simulink model "SimulinkAnalysisofCheetahTail"  (R2022a)
(part 3 of 21)

t1533 = t1424./2.0;
t1534 = t1425./2.0;
t1535 = t1426./2.0;
t1536 = dpsi1.*t1470;
t1541 = t1432./2.0;
t1572 = Mt.*t4.*t5.*t1381;
t1573 = T_cg_H.*t1512;
t1580 = dphi2.*t1512;
t1581 = dpsi1.*t1512;
t1585 = Mb.*t2.*t10.*t1382;
t1587 = Mb.*t7.*t10.*t1382;
t1592 = -t1540;
t1594 = -t1545;
t1595 = Mb.*t2.*t5.*t1362;
t1599 = Mb.*t5.*t7.*t1362;
t1601 = -t1553;
t1602 = -t1554;
t1603 = -t1556;
t1606 = t1488./2.0;
t1621 = Mm.*t9.*t10.*t1394;
t1624 = Mb.*t11.*t15.*t459.*t964;
t1655 = Mm.*t5.*t33.*t1394;
t1656 = Mm.*t5.*t38.*t1394;
t1658 = B_cg_H.*Mb.*t382.*t1178;
t1659 = Mm.*t4.*t10.*t1470;
t1669 = -t1629;
t1680 = Mm.*t381.*t1221;
t1681 = Mm.*t382.*t1221;
t1686 = -t1652;
t1695 = B_cg_H.*Mb.*t4.*t5.*t1512;
t1698 = t496.*t1178;
t1699 = B_cg_H.*Mb.*t9.*t10.*t1512;
t1703 = B_cg_H.*Mb.*t7.*t100.*t1382;
t1705 = t11.*t420.*t1178;
C = ft_5({B_cg_H,ITail,Mb,Mm,Mt,T_cg_H,dphi1,dphi2,dpsi1,dth1,dth2,dx,dy,dz,t10,t1003,t1004,t1005,t1006,t1007,t1008,t1009,t1010,t1011,t1012,t1013,t1014,t1015,t1016,t1017,t1018,t1019,t1020,t1021,t1023,t1024,t1025,t1026,t1029,t103,t1030,t1031,t1036,t1037,t1041,t1042,t1043,t1044,t1045,t1046,t1047,t1049,t105,t1050,t1051,t1052,t1053,t1054,t1055,t1056,t1057,t1058,t1059,t1060,t1061,t1062,t1063,t1064,t1065,t1067,t1068,t1071,t1072,t1073,t1074,t1075,t1076,t1077,t1078,t1079,t1080,t1081,t1082,t1084,t1085,t1086,t1088,t1093,t1095,t1097,t11,t1102,t1105,t1108,t1109,t1113,t1114,t1115,t1116,t1117,t1118,t1119,t1120,t1121,t1122,t1123,t1124,t1125,t1126,t1127,t1128,t1129,t1130,t1131,t1132,t1133,t1134,t1135,t1136,t1137,t1138,t1139,t1140,t1141,t1142,t1143,t1144,t1145,t1146,t1147,t1148,t1149,t1150,t1152,t1153,t1154,t1155,t1156,t1157,t1158,t1159,t1160,t1161,t1162,t1163,t1164,t1165,t1166,t1167,t1168,t1169,t1170,t1171,t1172,t1173,t1174,t1176,t1177,t1178,t1179,t1180,t1181,t1182,t1183,t1184,t1185,t1186,t1187,t1188,t1189,t1190,t1191,t1192,t1193,t1194,t1195,t1196,t1197,t1199,t120,t1200,t1201,t1202,t1203,t1205,t1206,t1207,t1209,t1211,t1212,t1213,t1214,t1215,t1216,t1217,t1218,t1221,t1223,t1224,t1225,t1226,t1227,t1228,t1229,t123,t1230,t1231,t1232,t1234,t1235,t1236,t1237,t1238,t1240,t1242,t1243,t1244,t1245,t1246,t1247,t1248,t1250,t1251,t1252,t1253,t1255,t1256,t1257,t1260,t1261,t1262,t1263,t1264,t1265,t1266,t1268,t1270,t1272,t1275,t1279,t1280,t1282,t1283,t1284,t1285,t1287,t1289,t1296,t130,t1301,t1302,t1303,t1304,t1305,t1306,t1307,t1308,t1309,t1311,t1312,t1313,t1319,t1320,t1322,t1323,t1324,t1325,t1328,t1329,t1331,t1332,t1334,t1335,t1337,t1338,t134,t1340,t1341,t1342,t1343,t1344,t1345,t1348,t1349,t1352,t1354,t1355,t1356,t1357,t1358,t1360,t1361,t1362,t1363,t1365,t1366,t1367,t1368,t1370,t1371,t1372,t1373,t1374,t1377,t1378,t1379,t1380,t1381,t1382,t1383,t1384,t1385,t1386,t1388,t1389,t1390,t1391,t1393,t1394,t1395,t1396,t1397,t1399,t1400,t1402,t1403,t1405,t1406,t1407,t1408,t1409,t1410,t1412,t1413,t1414,t1415,t1416,t1418,t1419,t1421,t1422,t1424,t1425,t1426,t1427,t1429,t1430,t1431,t1432,t1433,t1434,t1435,t1437,t1438,t1439,t144,t1440,t1441,t1442,t1443,t1444,t1445,t1446,t1447,t1448,t1450,t1451,t1453,t1454,t1455,t1456,t1457,t1458,t1459,t1460,t1461,t1462,t1463,t1465,t1466,t1467,t1468,t1469,t1470,t1471,t1472,t1475,t1476,t1477,t1478,t1479,t1481,t1482,t1483,t1484,t1486,t1487,t1488,t1489,t1491,t1492,t1493,t1494,t1495,t1496,t1497,t1498,t15,t1500,t1501,t1503,t1504,t1505,t1506,t1507,t1508,t1509,t1511,t1512,t1513,t1514,t1515,t1516,t1517,t1518,t1520,t1521,t1522,t1523,t1524,t1525,t1526,t1527,t1528,t1529,t1531,t1532,t1533,t1534,t1535,t1536,t1537,t1539,t1540,t1541,t1542,t1543,t1547,t1548,t1549,t1550,t1552,t1553,t1555,t1557,t1559,t1560,t1561,t1562,t1563,t1565,t1566,t1567,t1568,t1572,t1573,t1576,t1577,t1580,t1581,t1582,t1585,t1587,t1588,t1589,t1591,t1592,t1593,t1594,t1595,t1596,t1597,t1598,t1599,t160,t1600,t1601,t1602,t1603,t1605,t1606,t1609,t161,t1610,t1613,t1614,t1615,t1616,t1617,t1618,t1619,t162,t1620,t1621,t1624,t1627,t1628,t1632,t1635,t1636,t1637,t1639,t1640,t1641,t1642,t1644,t1645,t1646,t1647,t1648,t1649,t1651,t1652,t1653,t1654,t1655,t1656,t1657,t1658,t1659,t1660,t1661,t1663,t1664,t1665,t1667,t1668,t1669,t1670,t1671,t1672,t1673,t1674,t1675,t1676,t1677,t1678,t1679,t1680,t1681,t1682,t1683,t1684,t1685,t1686,t1687,t1688,t1689,t1690,t1691,t1692,t1693,t1694,t1695,t1698,t1699,t1700,t1701,t1702,t1703,t1704,t1705,t1706,t1707,t1708,t1709,t1710,t1711,t1712,t1714,t1715,t1716,t1717,t1718,t1723,t1726,t1727,t1731,t1732,t1733,t1734,t1737,t1741,t1742,t1743,t1744,t1745,t1747,t1749,t1751,t1758,t1759,t1760,t1761,t1762,t1764,t1765,t1769,t1770,t1773,t1775,t1777,t1784,t1786,t1788,t1791,t1796,t1798,t1799,t1801,t1802,t1803,t1805,t1806,t1808,t1810,t1812,t1813,t1814,t1815,t1817,t1819,t1820,t1824,t1825,t1826,t1829,t1830,t1832,t1836,t1837,t1838,t1839,t1841,t1844,t1851,t1852,t1856,t1862,t1865,t1866,t1867,t1871,t1873,t1874,t1875,t1881,t1884,t1888,t1894,t1895,t1896,t1897,t1899,t1903,t1905,t1906,t1907,t1908,t1909,t1910,t1911,t1912,t1913,t1914,t1915,t1916,t1918,t1919,t1921,t1922,t1926,t1928,t1930,t1931,t1936,t1940,t1941,t1942,t195,t1954,t1956,t1958,t1960,t1961,t1962,t1963,t1964,t1965,t1966,t1969,t197,t1970,t1971,t1973,t1974,t1975,t1979,t1981,t1982,t1983,t1985,t1989,t1990,t1998,t1999,t2,t2004,t2007,t2008,t2015,t2025,t2026,t2028,t2031,t2035,t2037,t2042,t2043,t2045,t2046,t2047,t2050,t2052,t2053,t2056,t2057,t2058,t2059,t2062,t2063,t2064,t2066,t2067,t2068,t2069,t2072,t2078,t2087,t2090,t2091,t2094,t2095,t2096,t2097,t2098,t2102,t2104,t2118,t2119,t2120,t2121,t2127,t213,t2130,t2131,t2134,t2135,t214,t2141,t2144,t2146,t2147,t2148,t2150,t2151,t2152,t2154,t2155,t2156,t2157,t2158,t2161,t2165,t2167,t2171,t2172,t2176,t2178,t2179,t2180,t2181,t2182,t2183,t2186,t2188,t2190,t2196,t2201,t2202,t2203,t2205,t2208,t2209,t2211,t2214,t2215,t2218,t2220,t2222,t2224,t2225,t2227,t2231,t2237,t2238,t2240,t2242,t2245,t2246,t2247,t2249,t2251,t2252,t2253,t2254,t2255,t2257,t2259,t2262,t2263,t2264,t2266,t2273,t2283,t2287,t2288,t2290,t2294,t2298,t23,t2303,t2305,t2306,t2307,t2312,t2320,t2321,t2322,t2323,t2324,t2326,t2327,t2328,t2331,t2335,t2336,t2339,t2340,t2341,t2342,t2343,t2345,t2346,t2347,t2349,t2350,t2351,t2356,t2358,t2359,t2360,t2362,t2363,t2376,t2379,t2383,t2385,t2386,t2387,t2388,t2389,t2390,t2392,t2397,t2399,t24,t2400,t2401,t2404,t2407,t2408,t2409,t2411,t2412,t2420,t2427,t2429,t2430,t2431,t2433,t2435,t2447,t2461,t2462,t2463,t2464,t2466,t2467,t2468,t2469,t2474,t2475,t2476,t2477,t2479,t2480,t2482,t2485,t2487,t2488,t2489,t2492,t2493,t2494,t2495,t2497,t25,t2503,t2504,t2505,t2512,t2514,t2515,t2516,t2518,t2519,t2520,t2527,t2530,t2531,t2532,t2534,t2539,t2544,t2545,t2546,t2560,t2562,t2563,t2564,t2565,t2566,t2570,t2576,t2577,t2581,t2584,t2586,t2587,t2588,t2589,t259,t2590,t2591,t2597,t2598,t2599,t26,t260,t2600,t2603,t2604,t2607,t2608,t2611,t2612,t2613,t2614,t2615,t2616,t2617,t2619,t262,t2620,t2621,t2622,t2624,t2626,t2627,t2632,t2634,t2638,t2654,t2660,t2662,t2663,t2664,t2665,t2668,t2669,t2671,t2673,t2681,t2682,t2689,t2692,t2693,t2694,t2695,t2698,t2699,t27,t2700,t2701,t2702,t2704,t2705,t2706,t2707,t2708,t2710,t2711,t2712,t2713,t2714,t2715,t2717,t2718,t2719,t2720,t2721,t2722,t2723,t2724,t273,t2730,t2731,t2732,t2740,t2742,t2745,t2749,t2751,t2752,t2756,t276,t2763,t2764,t2765,t2766,t277,t2774,t2776,t2781,t2782,t2783,t2784,t2786,t2787,t2788,t2790,t28,t2802,t2803,t2804,t2806,t2807,t2812,t2813,t2819,t2820,t2821,t2825,t2828,t283,t2835,t2837,t2839,t284,t2841,t2842,t2844,t285,t2857,t2859,t286,t287,t2870,t2872,t2874,t2875,t2879,t288,t2880,t2883,t2884,t2886,t2887,t2888,t2889,t289,t2890,t2892,t2895,t2896,t290,t2902,t2907,t2908,t2909,t291,t2912,t2913,t2916,t2918,t292,t2928,t2929,t293,t2932,t2938,t294,t2945,t2946,t2949,t2950,t2951,t2952,t2954,t2955,t2956,t2957,t2958,t2959,t2960,t2961,t2967,t2969,t2975,t2977,t2982,t2988,t2992,t2995,t3,t30,t3004,t3010,t3011,t3017,t3019,t3020,t3022,t3023,t3025,t3028,t3030,t3034,t3035,t3039,t304,t3047,t3048,t3051,t3055,t3058,t3059,t3060,t3063,t3065,t3067,t3068,t3074,t3075,t3077,t3078,t3081,t3085,t3088,t3090,t3105,t3109,t3111,t3117,t3120,t3124,t3130,t3132,t3134,t3135,t3136,t3138,t3153,t3165,t3170,t3173,t3177,t3181,t3182,t3186,t3188,t3191,t3194,t3199,t3200,t3201,t3204,t3210,t3212,t3218,t3235,t3237,t3243,t3247,t3248,t3249,t3256,t3260,t3265,t3266,t3269,t3272,t3285,t3291,t33,t3304,t3310,t3317,t3330,t3331,t3337,t3351,t3360,t3364,t3370,t3380,t34,t3419,t3426,t3428,t3434,t3438,t3441,t3449,t3459,t346,t3469,t347,t3471,t3478,t348,t3484,t3499,t35,t3504,t3520,t3521,t3522,t3527,t3531,t3565,t3580,t3581,t3644,t3701,t3704,t3709,t375,t376,t377,t38,t380,t381,t382,t3823,t383,t3847,t3858,t3862,t3880,t3881,t3882,t3883,t390,t3902,t3908,t3909,t3916,t3926,t3930,t3931,t3932,t3937,t394,t3940,t3944,t3955,t3957,t3959,t3962,t3963,t3964,t3965,t3969,t3971,t3982,t399,t3994,t3996,t3998,t4,t40,t400,t4003,t4008,t401,t4014,t4033,t4038,t4042,t4054,t4061,t4070,t4078,t4081,t4090,t4098,t41,t410,t411,t412,t4121,t413,t414,t4141,t4142,t4143,t415,t4153,t4161,t4172,t4181,t4182,t4189,t4190,t4197,t420,t421,t4210,t4218,t4234,t4235,t4236,t424,t425,t4256,t4269,t4294,t4295,t4297,t4298,t430,t431,t4323,t433,t434,t4349,t4355,t436,t4363,t44,t445,t4474,t4475,t448,t450,t4509,t451,t456,t459,t4597,t4598,t4599,t46,t4603,t463,t465,t466,t4752,t478,t479,t48,t480,t482,t483,t484,t485,t487,t488,t49,t491,t495,t496,t5,t50,t501,t502,t504,t505,t506,t51,t514,t519,t523,t524,t527,t530,t532,t533,t534,t537,t539,t54,t541,t542,t544,t545,t546,t547,t55,t550,t553,t555,t557,t558,t559,t56,t560,t561,t563,t568,t569,t57,t572,t573,t574,t575,t578,t581,t584,t587,t59,t595,t6,t602,t603,t61,t614,t623,t624,t627,t628,t629,t631,t632,t634,t641,t643,t644,t646,t648,t649,t65,t650,t651,t652,t653,t654,t655,t657,t662,t663,t664,t665,t666,t667,t668,t669,t672,t674,t675,t676,t68,t69,t693,t699,t7,t701,t71,t720,t721,t722,t724,t73,t731,t732,t735,t736,t741,t742,t743,t744,t746,t749,t750,t751,t752,t753,t754,t755,t756,t757,t759,t760,t761,t762,t764,t765,t768,t769,t772,t774,t776,t778,t779,t792,t794,t795,t797,t799,t8,t801,t802,t803,t804,t805,t806,t811,t817,t818,t819,t820,t821,t822,t823,t824,t826,t828,t829,t830,t831,t833,t834,t835,t836,t837,t838,t839,t841,t842,t843,t844,t845,t846,t847,t848,t850,t851,t852,t853,t854,t855,t858,t859,t862,t863,t864,t865,t867,t868,t869,t870,t871,t872,t873,t874,t875,t876,t877,t879,t881,t882,t884,t885,t886,t887,t888,t889,t890,t891,t892,t893,t894,t895,t896,t897,t898,t9,t900,t901,t902,t903,t904,t906,t907,t908,t909,t910,t912,t913,t914,t915,t916,t917,t918,t919,t923,t924,t925,t926,t927,t928,t933,t934,t936,t941,t947,t948,t949,t950,t951,t952,t953,t954,t955,t956,t957,t964,t965,t966,t968,t970,t972,t973,t974,t976,t977,t979,t980,t983,t985,t986,t987,t990,t991,t992,t993,t994,t995,t996});
end
function C = ft_5(ct)
B_cg_H = ct{1};
ITail = ct{2};
Mb = ct{3};
Mm = ct{4};
Mt = ct{5};
T_cg_H = ct{6};
dphi1 = ct{7};
dphi2 = ct{8};
dpsi1 = ct{9};
dth1 = ct{10};
dth2 = ct{11};
dx = ct{12};
dy = ct{13};
dz = ct{14};
t10 = ct{15};
t1003 = ct{16};
t1004 = ct{17};
t1005 = ct{18};
t1006 = ct{19};
t1007 = ct{20};
t1008 = ct{21};
t1009 = ct{22};
t1010 = ct{23};
t1011 = ct{24};
t1012 = ct{25};
t1013 = ct{26};
t1014 = ct{27};
t1015 = ct{28};
t1016 = ct{29};
t1017 = ct{30};
t1018 = ct{31};
t1019 = ct{32};
t1020 = ct{33};
t1021 = ct{34};
t1023 = ct{35};
t1024 = ct{36};
t1025 = ct{37};
t1026 = ct{38};
t1029 = ct{39};
t103 = ct{40};
t1030 = ct{41};
t1031 = ct{42};
t1036 = ct{43};
t1037 = ct{44};
t1041 = ct{45};
t1042 = ct{46};
t1043 = ct{47};
t1044 = ct{48};
t1045 = ct{49};
t1046 = ct{50};
t1047 = ct{51};
t1049 = ct{52};
t105 = ct{53};
t1050 = ct{54};
t1051 = ct{55};
t1052 = ct{56};
t1053 = ct{57};
t1054 = ct{58};
t1055 = ct{59};
t1056 = ct{60};
t1057 = ct{61};
t1058 = ct{62};
t1059 = ct{63};
t1060 = ct{64};
t1061 = ct{65};
t1062 = ct{66};
t1063 = ct{67};
t1064 = ct{68};
t1065 = ct{69};
t1067 = ct{70};
t1068 = ct{71};
t1071 = ct{72};
t1072 = ct{73};
t1073 = ct{74};
t1074 = ct{75};
t1075 = ct{76};
t1076 = ct{77};
t1077 = ct{78};
t1078 = ct{79};
t1079 = ct{80};
t1080 = ct{81};
t1081 = ct{82};
t1082 = ct{83};
t1084 = ct{84};
t1085 = ct{85};
t1086 = ct{86};
t1088 = ct{87};
t1093 = ct{88};
t1095 = ct{89};
t1097 = ct{90};
t11 = ct{91};
t1102 = ct{92};
t1105 = ct{93};
t1108 = ct{94};
t1109 = ct{95};
t1113 = ct{96};
t1114 = ct{97};
t1115 = ct{98};
t1116 = ct{99};
t1117 = ct{100};
t1118 = ct{101};
t1119 = ct{102};
t1120 = ct{103};
t1121 = ct{104};
t1122 = ct{105};
t1123 = ct{106};
t1124 = ct{107};
t1125 = ct{108};
t1126 = ct{109};
t1127 = ct{110};
t1128 = ct{111};
t1129 = ct{112};
t1130 = ct{113};
t1131 = ct{114};
t1132 = ct{115};
t1133 = ct{116};
t1134 = ct{117};
t1135 = ct{118};
t1136 = ct{119};
t1137 = ct{120};
t1138 = ct{121};
t1139 = ct{122};
t1140 = ct{123};
t1141 = ct{124};
t1142 = ct{125};
t1143 = ct{126};
t1144 = ct{127};
t1145 = ct{128};
t1146 = ct{129};
t1147 = ct{130};
t1148 = ct{131};
t1149 = ct{132};
t1150 = ct{133};
t1152 = ct{134};
t1153 = ct{135};
t1154 = ct{136};
t1155 = ct{137};
t1156 = ct{138};
t1157 = ct{139};
t1158 = ct{140};
t1159 = ct{141};
t1160 = ct{142};
t1161 = ct{143};
t1162 = ct{144};
t1163 = ct{145};
t1164 = ct{146};
t1165 = ct{147};
t1166 = ct{148};
t1167 = ct{149};
t1168 = ct{150};
t1169 = ct{151};
t1170 = ct{152};
t1171 = ct{153};
t1172 = ct{154};
t1173 = ct{155};
t1174 = ct{156};
t1176 = ct{157};
t1177 = ct{158};
t1178 = ct{159};
t1179 = ct{160};
t1180 = ct{161};
t1181 = ct{162};
t1182 = ct{163};
t1183 = ct{164};
t1184 = ct{165};
t1185 = ct{166};
t1186 = ct{167};
t1187 = ct{168};
t1188 = ct{169};
t1189 = ct{170};
t1190 = ct{171};
t1191 = ct{172};
t1192 = ct{173};
t1193 = ct{174};
t1194 = ct{175};
t1195 = ct{176};
t1196 = ct{177};
t1197 = ct{178};
t1199 = ct{179};
t120 = ct{180};
t1200 = ct{181};
t1201 = ct{182};
t1202 = ct{183};
t1203 = ct{184};
t1205 = ct{185};
t1206 = ct{186};
t1207 = ct{187};
t1209 = ct{188};
t1211 = ct{189};
t1212 = ct{190};
t1213 = ct{191};
t1214 = ct{192};
t1215 = ct{193};
t1216 = ct{194};
t1217 = ct{195};
t1218 = ct{196};
t1221 = ct{197};
t1223 = ct{198};
t1224 = ct{199};
t1225 = ct{200};
t1226 = ct{201};
t1227 = ct{202};
t1228 = ct{203};
t1229 = ct{204};
t123 = ct{205};
t1230 = ct{206};
t1231 = ct{207};
t1232 = ct{208};
t1234 = ct{209};
t1235 = ct{210};
t1236 = ct{211};
t1237 = ct{212};
t1238 = ct{213};
t1240 = ct{214};
t1242 = ct{215};
t1243 = ct{216};
t1244 = ct{217};
t1245 = ct{218};
t1246 = ct{219};
t1247 = ct{220};
t1248 = ct{221};
t1250 = ct{222};
t1251 = ct{223};
t1252 = ct{224};
t1253 = ct{225};
t1255 = ct{226};
t1256 = ct{227};
t1257 = ct{228};
t1260 = ct{229};
t1261 = ct{230};
t1262 = ct{231};
t1263 = ct{232};
t1264 = ct{233};
t1265 = ct{234};
t1266 = ct{235};
t1268 = ct{236};
t1270 = ct{237};
t1272 = ct{238};
t1275 = ct{239};
t1279 = ct{240};
t1280 = ct{241};
t1282 = ct{242};
t1283 = ct{243};
t1284 = ct{244};
t1285 = ct{245};
t1287 = ct{246};
t1289 = ct{247};
t1296 = ct{248};
t130 = ct{249};
t1301 = ct{250};
t1302 = ct{251};
t1303 = ct{252};
t1304 = ct{253};
t1305 = ct{254};
t1306 = ct{255};
t1307 = ct{256};
t1308 = ct{257};
t1309 = ct{258};
t1311 = ct{259};
t1312 = ct{260};
t1313 = ct{261};
t1319 = ct{262};
t1320 = ct{263};
t1322 = ct{264};
t1323 = ct{265};
t1324 = ct{266};
t1325 = ct{267};
t1328 = ct{268};
t1329 = ct{269};
t1331 = ct{270};
t1332 = ct{271};
t1334 = ct{272};
t1335 = ct{273};
t1337 = ct{274};
t1338 = ct{275};
t134 = ct{276};
t1340 = ct{277};
t1341 = ct{278};
t1342 = ct{279};
t1343 = ct{280};
t1344 = ct{281};
t1345 = ct{282};
t1348 = ct{283};
t1349 = ct{284};
t1352 = ct{285};
t1354 = ct{286};
t1355 = ct{287};
t1356 = ct{288};
t1357 = ct{289};
t1358 = ct{290};
t1360 = ct{291};
t1361 = ct{292};
t1362 = ct{293};
t1363 = ct{294};
t1365 = ct{295};
t1366 = ct{296};
t1367 = ct{297};
t1368 = ct{298};
t1370 = ct{299};
t1371 = ct{300};
t1372 = ct{301};
t1373 = ct{302};
t1374 = ct{303};
t1377 = ct{304};
t1378 = ct{305};
t1379 = ct{306};
t1380 = ct{307};
t1381 = ct{308};
t1382 = ct{309};
t1383 = ct{310};
t1384 = ct{311};
t1385 = ct{312};
t1386 = ct{313};
t1388 = ct{314};
t1389 = ct{315};
t1390 = ct{316};
t1391 = ct{317};
t1393 = ct{318};
t1394 = ct{319};
t1395 = ct{320};
t1396 = ct{321};
t1397 = ct{322};
t1399 = ct{323};
t1400 = ct{324};
t1402 = ct{325};
t1403 = ct{326};
t1405 = ct{327};
t1406 = ct{328};
t1407 = ct{329};
t1408 = ct{330};
t1409 = ct{331};
t1410 = ct{332};
t1412 = ct{333};
t1413 = ct{334};
t1414 = ct{335};
t1415 = ct{336};
t1416 = ct{337};
t1418 = ct{338};
t1419 = ct{339};
t1421 = ct{340};
t1422 = ct{341};
t1424 = ct{342};
t1425 = ct{343};
t1426 = ct{344};
t1427 = ct{345};
t1429 = ct{346};
t1430 = ct{347};
t1431 = ct{348};
t1432 = ct{349};
t1433 = ct{350};
t1434 = ct{351};
t1435 = ct{352};
t1437 = ct{353};
t1438 = ct{354};
t1439 = ct{355};
t144 = ct{356};
t1440 = ct{357};
t1441 = ct{358};
t1442 = ct{359};
t1443 = ct{360};
t1444 = ct{361};
t1445 = ct{362};
t1446 = ct{363};
t1447 = ct{364};
t1448 = ct{365};
t1450 = ct{366};
t1451 = ct{367};
t1453 = ct{368};
t1454 = ct{369};
t1455 = ct{370};
t1456 = ct{371};
t1457 = ct{372};
t1458 = ct{373};
t1459 = ct{374};
t1460 = ct{375};
t1461 = ct{376};
t1462 = ct{377};
t1463 = ct{378};
t1465 = ct{379};
t1466 = ct{380};
t1467 = ct{381};
t1468 = ct{382};
t1469 = ct{383};
t1470 = ct{384};
t1471 = ct{385};
t1472 = ct{386};
t1475 = ct{387};
t1476 = ct{388};
t1477 = ct{389};
t1478 = ct{390};
t1479 = ct{391};
t1481 = ct{392};
t1482 = ct{393};
t1483 = ct{394};
t1484 = ct{395};
t1486 = ct{396};
t1487 = ct{397};
t1488 = ct{398};
t1489 = ct{399};
t1491 = ct{400};
t1492 = ct{401};
t1493 = ct{402};
t1494 = ct{403};
t1495 = ct{404};
t1496 = ct{405};
t1497 = ct{406};
t1498 = ct{407};
t15 = ct{408};
t1500 = ct{409};
t1501 = ct{410};
t1503 = ct{411};
t1504 = ct{412};
t1505 = ct{413};
t1506 = ct{414};
t1507 = ct{415};
t1508 = ct{416};
t1509 = ct{417};
t1511 = ct{418};
t1512 = ct{419};
t1513 = ct{420};
t1514 = ct{421};
t1515 = ct{422};
t1516 = ct{423};
t1517 = ct{424};
t1518 = ct{425};
t1520 = ct{426};
t1521 = ct{427};
t1522 = ct{428};
t1523 = ct{429};
t1524 = ct{430};
t1525 = ct{431};
t1526 = ct{432};
t1527 = ct{433};
t1528 = ct{434};
t1529 = ct{435};
t1531 = ct{436};
t1532 = ct{437};
t1533 = ct{438};
t1534 = ct{439};
t1535 = ct{440};
t1536 = ct{441};
t1537 = ct{442};
t1539 = ct{443};
t1540 = ct{444};
t1541 = ct{445};
t1542 = ct{446};
t1543 = ct{447};
t1547 = ct{448};
t1548 = ct{449};
t1549 = ct{450};
t1550 = ct{451};
t1552 = ct{452};
t1553 = ct{453};
t1555 = ct{454};
t1557 = ct{455};
t1559 = ct{456};
t1560 = ct{457};
t1561 = ct{458};
t1562 = ct{459};
t1563 = ct{460};
t1565 = ct{461};
t1566 = ct{462};
t1567 = ct{463};
t1568 = ct{464};
t1572 = ct{465};
t1573 = ct{466};
t1576 = ct{467};
t1577 = ct{468};
t1580 = ct{469};
t1581 = ct{470};
t1582 = ct{471};
t1585 = ct{472};
t1587 = ct{473};
t1588 = ct{474};
t1589 = ct{475};
t1591 = ct{476};
t1592 = ct{477};
t1593 = ct{478};
t1594 = ct{479};
t1595 = ct{480};
t1596 = ct{481};
t1597 = ct{482};
t1598 = ct{483};
t1599 = ct{484};
t160 = ct{485};
t1600 = ct{486};
t1601 = ct{487};
t1602 = ct{488};
t1603 = ct{489};
t1605 = ct{490};
t1606 = ct{491};
t1609 = ct{492};
t161 = ct{493};
t1610 = ct{494};
t1613 = ct{495};
t1614 = ct{496};
t1615 = ct{497};
t1616 = ct{498};
t1617 = ct{499};
t1618 = ct{500};
t1619 = ct{501};
t162 = ct{502};
t1620 = ct{503};
t1621 = ct{504};
t1624 = ct{505};
t1627 = ct{506};
t1628 = ct{507};
t1632 = ct{508};
t1635 = ct{509};
t1636 = ct{510};
t1637 = ct{511};
t1639 = ct{512};
t1640 = ct{513};
t1641 = ct{514};
t1642 = ct{515};
t1644 = ct{516};
t1645 = ct{517};
t1646 = ct{518};
t1647 = ct{519};
t1648 = ct{520};
t1649 = ct{521};
t1651 = ct{522};
t1652 = ct{523};
t1653 = ct{524};
t1654 = ct{525};
t1655 = ct{526};
t1656 = ct{527};
t1657 = ct{528};
t1658 = ct{529};
t1659 = ct{530};
t1660 = ct{531};
t1661 = ct{532};
t1663 = ct{533};
t1664 = ct{534};
t1665 = ct{535};
t1667 = ct{536};
t1668 = ct{537};
t1669 = ct{538};
t1670 = ct{539};
t1671 = ct{540};
t1672 = ct{541};
t1673 = ct{542};
t1674 = ct{543};
t1675 = ct{544};
t1676 = ct{545};
t1677 = ct{546};
t1678 = ct{547};
t1679 = ct{548};
t1680 = ct{549};
t1681 = ct{550};
t1682 = ct{551};
t1683 = ct{552};
t1684 = ct{553};
t1685 = ct{554};
t1686 = ct{555};
t1687 = ct{556};
t1688 = ct{557};
t1689 = ct{558};
t1690 = ct{559};
t1691 = ct{560};
t1692 = ct{561};
t1693 = ct{562};
t1694 = ct{563};
t1695 = ct{564};
t1698 = ct{565};
t1699 = ct{566};
t1700 = ct{567};
t1701 = ct{568};
t1702 = ct{569};
t1703 = ct{570};
t1704 = ct{571};
t1705 = ct{572};
t1706 = ct{573};
t1707 = ct{574};
t1708 = ct{575};
t1709 = ct{576};
t1710 = ct{577};
t1711 = ct{578};
t1712 = ct{579};
t1714 = ct{580};
t1715 = ct{581};
t1716 = ct{582};
t1717 = ct{583};
t1718 = ct{584};
t1723 = ct{585};
t1726 = ct{586};
t1727 = ct{587};
t1731 = ct{588};
t1732 = ct{589};
t1733 = ct{590};
t1734 = ct{591};
t1737 = ct{592};
t1741 = ct{593};
t1742 = ct{594};
t1743 = ct{595};
t1744 = ct{596};
t1745 = ct{597};
t1747 = ct{598};
t1749 = ct{599};
t1751 = ct{600};
t1758 = ct{601};
t1759 = ct{602};
t1760 = ct{603};
t1761 = ct{604};
t1762 = ct{605};
t1764 = ct{606};
t1765 = ct{607};
t1769 = ct{608};
t1770 = ct{609};
t1773 = ct{610};
t1775 = ct{611};
t1777 = ct{612};
t1784 = ct{613};
t1786 = ct{614};
t1788 = ct{615};
t1791 = ct{616};
t1796 = ct{617};
t1798 = ct{618};
t1799 = ct{619};
t1801 = ct{620};
t1802 = ct{621};
t1803 = ct{622};
t1805 = ct{623};
t1806 = ct{624};
t1808 = ct{625};
t1810 = ct{626};
t1812 = ct{627};
t1813 = ct{628};
t1814 = ct{629};
t1815 = ct{630};
t1817 = ct{631};
t1819 = ct{632};
t1820 = ct{633};
t1824 = ct{634};
t1825 = ct{635};
t1826 = ct{636};
t1829 = ct{637};
t1830 = ct{638};
t1832 = ct{639};
t1836 = ct{640};
t1837 = ct{641};
t1838 = ct{642};
t1839 = ct{643};
t1841 = ct{644};
t1844 = ct{645};
t1851 = ct{646};
t1852 = ct{647};
t1856 = ct{648};
t1862 = ct{649};
t1865 = ct{650};
t1866 = ct{651};
t1867 = ct{652};
t1871 = ct{653};
t1873 = ct{654};
t1874 = ct{655};
t1875 = ct{656};
t1881 = ct{657};
t1884 = ct{658};
t1888 = ct{659};
t1894 = ct{660};
t1895 = ct{661};
t1896 = ct{662};
t1897 = ct{663};
t1899 = ct{664};
t1903 = ct{665};
t1905 = ct{666};
t1906 = ct{667};
t1907 = ct{668};
t1908 = ct{669};
t1909 = ct{670};
t1910 = ct{671};
t1911 = ct{672};
t1912 = ct{673};
t1913 = ct{674};
t1914 = ct{675};
t1915 = ct{676};
t1916 = ct{677};
t1918 = ct{678};
t1919 = ct{679};
t1921 = ct{680};
t1922 = ct{681};
t1926 = ct{682};
t1928 = ct{683};
t1930 = ct{684};
t1931 = ct{685};
t1936 = ct{686};
t1940 = ct{687};
t1941 = ct{688};
t1942 = ct{689};
t195 = ct{690};
t1954 = ct{691};
t1956 = ct{692};
t1958 = ct{693};
t1960 = ct{694};
t1961 = ct{695};
t1962 = ct{696};
t1963 = ct{697};
t1964 = ct{698};
t1965 = ct{699};
t1966 = ct{700};
t1969 = ct{701};
t197 = ct{702};
t1970 = ct{703};
t1971 = ct{704};
t1973 = ct{705};
t1974 = ct{706};
t1975 = ct{707};
t1979 = ct{708};
t1981 = ct{709};
t1982 = ct{710};
t1983 = ct{711};
t1985 = ct{712};
t1989 = ct{713};
t1990 = ct{714};
t1998 = ct{715};
t1999 = ct{716};
t2 = ct{717};
t2004 = ct{718};
t2007 = ct{719};
t2008 = ct{720};
t2015 = ct{721};
t2025 = ct{722};
t2026 = ct{723};
t2028 = ct{724};
t2031 = ct{725};
t2035 = ct{726};
t2037 = ct{727};
t2042 = ct{728};
t2043 = ct{729};
t2045 = ct{730};
t2046 = ct{731};
t2047 = ct{732};
t2050 = ct{733};
t2052 = ct{734};
t2053 = ct{735};
t2056 = ct{736};
t2057 = ct{737};
t2058 = ct{738};
t2059 = ct{739};
t2062 = ct{740};
t2063 = ct{741};
t2064 = ct{742};
t2066 = ct{743};
t2067 = ct{744};
t2068 = ct{745};
t2069 = ct{746};
t2072 = ct{747};
t2078 = ct{748};
t2087 = ct{749};
t2090 = ct{750};
t2091 = ct{751};
t2094 = ct{752};
t2095 = ct{753};
t2096 = ct{754};
t2097 = ct{755};
t2098 = ct{756};
t2102 = ct{757};
t2104 = ct{758};
t2118 = ct{759};
t2119 = ct{760};
t2120 = ct{761};
t2121 = ct{762};
t2127 = ct{763};
t213 = ct{764};
t2130 = ct{765};
t2131 = ct{766};
t2134 = ct{767};
t2135 = ct{768};
t214 = ct{769};
t2141 = ct{770};
t2144 = ct{771};
t2146 = ct{772};
t2147 = ct{773};
t2148 = ct{774};
t2150 = ct{775};
t2151 = ct{776};
t2152 = ct{777};
t2154 = ct{778};
t2155 = ct{779};
t2156 = ct{780};
t2157 = ct{781};
t2158 = ct{782};
t2161 = ct{783};
t2165 = ct{784};
t2167 = ct{785};
t2171 = ct{786};
t2172 = ct{787};
t2176 = ct{788};
t2178 = ct{789};
t2179 = ct{790};
t2180 = ct{791};
t2181 = ct{792};
t2182 = ct{793};
t2183 = ct{794};
t2186 = ct{795};
t2188 = ct{796};
t2190 = ct{797};
t2196 = ct{798};
t2201 = ct{799};
t2202 = ct{800};
t2203 = ct{801};
t2205 = ct{802};
t2208 = ct{803};
t2209 = ct{804};
t2211 = ct{805};
t2214 = ct{806};
t2215 = ct{807};
t2218 = ct{808};
t2220 = ct{809};
t2222 = ct{810};
t2224 = ct{811};
t2225 = ct{812};
t2227 = ct{813};
t2231 = ct{814};
t2237 = ct{815};
t2238 = ct{816};
t2240 = ct{817};
t2242 = ct{818};
t2245 = ct{819};
t2246 = ct{820};
t2247 = ct{821};
t2249 = ct{822};
t2251 = ct{823};
t2252 = ct{824};
t2253 = ct{825};
t2254 = ct{826};
t2255 = ct{827};
t2257 = ct{828};
t2259 = ct{829};
t2262 = ct{830};
t2263 = ct{831};
t2264 = ct{832};
t2266 = ct{833};
t2273 = ct{834};
t2283 = ct{835};
t2287 = ct{836};
t2288 = ct{837};
t2290 = ct{838};
t2294 = ct{839};
t2298 = ct{840};
t23 = ct{841};
t2303 = ct{842};
t2305 = ct{843};
t2306 = ct{844};
t2307 = ct{845};
t2312 = ct{846};
t2320 = ct{847};
t2321 = ct{848};
t2322 = ct{849};
t2323 = ct{850};
t2324 = ct{851};
t2326 = ct{852};
t2327 = ct{853};
t2328 = ct{854};
t2331 = ct{855};
t2335 = ct{856};
t2336 = ct{857};
t2339 = ct{858};
t2340 = ct{859};
t2341 = ct{860};
t2342 = ct{861};
t2343 = ct{862};
t2345 = ct{863};
t2346 = ct{864};
t2347 = ct{865};
t2349 = ct{866};
t2350 = ct{867};
t2351 = ct{868};
t2356 = ct{869};
t2358 = ct{870};
t2359 = ct{871};
t2360 = ct{872};
t2362 = ct{873};
t2363 = ct{874};
t2376 = ct{875};
t2379 = ct{876};
t2383 = ct{877};
t2385 = ct{878};
t2386 = ct{879};
t2387 = ct{880};
t2388 = ct{881};
t2389 = ct{882};
t2390 = ct{883};
t2392 = ct{884};
t2397 = ct{885};
t2399 = ct{886};
t24 = ct{887};
t2400 = ct{888};
t2401 = ct{889};
t2404 = ct{890};
t2407 = ct{891};
t2408 = ct{892};
t2409 = ct{893};
t2411 = ct{894};
t2412 = ct{895};
t2420 = ct{896};
t2427 = ct{897};
t2429 = ct{898};
t2430 = ct{899};
t2431 = ct{900};
t2433 = ct{901};
t2435 = ct{902};
t2447 = ct{903};
t2461 = ct{904};
t2462 = ct{905};
t2463 = ct{906};
t2464 = ct{907};
t2466 = ct{908};
t2467 = ct{909};
t2468 = ct{910};
t2469 = ct{911};
t2474 = ct{912};
t2475 = ct{913};
t2476 = ct{914};
t2477 = ct{915};
t2479 = ct{916};
t2480 = ct{917};
t2482 = ct{918};
t2485 = ct{919};
t2487 = ct{920};
t2488 = ct{921};
t2489 = ct{922};
t2492 = ct{923};
t2493 = ct{924};
t2494 = ct{925};
t2495 = ct{926};
t2497 = ct{927};
t25 = ct{928};
t2503 = ct{929};
t2504 = ct{930};
t2505 = ct{931};
t2512 = ct{932};
t2514 = ct{933};
t2515 = ct{934};
t2516 = ct{935};
t2518 = ct{936};
t2519 = ct{937};
t2520 = ct{938};
t2527 = ct{939};
t2530 = ct{940};
t2531 = ct{941};
t2532 = ct{942};
t2534 = ct{943};
t2539 = ct{944};
t2544 = ct{945};
t2545 = ct{946};
t2546 = ct{947};
t2560 = ct{948};
t2562 = ct{949};
t2563 = ct{950};
t2564 = ct{951};
t2565 = ct{952};
t2566 = ct{953};
t2570 = ct{954};
t2576 = ct{955};
t2577 = ct{956};
t2581 = ct{957};
t2584 = ct{958};
t2586 = ct{959};
t2587 = ct{960};
t2588 = ct{961};
t2589 = ct{962};
t259 = ct{963};
t2590 = ct{964};
t2591 = ct{965};
t2597 = ct{966};
t2598 = ct{967};
t2599 = ct{968};
t26 = ct{969};
t260 = ct{970};
t2600 = ct{971};
t2603 = ct{972};
t2604 = ct{973};
t2607 = ct{974};
t2608 = ct{975};
t2611 = ct{976};
t2612 = ct{977};
t2613 = ct{978};
t2614 = ct{979};
t2615 = ct{980};
t2616 = ct{981};
t2617 = ct{982};
t2619 = ct{983};
t262 = ct{984};
t2620 = ct{985};
t2621 = ct{986};
t2622 = ct{987};
t2624 = ct{988};
t2626 = ct{989};
t2627 = ct{990};
t2632 = ct{991};
t2634 = ct{992};
t2638 = ct{993};
t2654 = ct{994};
t2660 = ct{995};
t2662 = ct{996};
t2663 = ct{997};
t2664 = ct{998};
t2665 = ct{999};
t2668 = ct{1000};
t2669 = ct{1001};
t2671 = ct{1002};
t2673 = ct{1003};
t2681 = ct{1004};
t2682 = ct{1005};
t2689 = ct{1006};
t2692 = ct{1007};
t2693 = ct{1008};
t2694 = ct{1009};
t2695 = ct{1010};
t2698 = ct{1011};
t2699 = ct{1012};
t27 = ct{1013};
t2700 = ct{1014};
t2701 = ct{1015};
t2702 = ct{1016};
t2704 = ct{1017};
t2705 = ct{1018};
t2706 = ct{1019};
t2707 = ct{1020};
t2708 = ct{1021};
t2710 = ct{1022};
t2711 = ct{1023};
t2712 = ct{1024};
t2713 = ct{1025};
t2714 = ct{1026};
t2715 = ct{1027};
t2717 = ct{1028};
t2718 = ct{1029};
t2719 = ct{1030};
t2720 = ct{1031};
t2721 = ct{1032};
t2722 = ct{1033};
t2723 = ct{1034};
t2724 = ct{1035};
t273 = ct{1036};
t2730 = ct{1037};
t2731 = ct{1038};
t2732 = ct{1039};
t2740 = ct{1040};
t2742 = ct{1041};
t2745 = ct{1042};
t2749 = ct{1043};
t2751 = ct{1044};
t2752 = ct{1045};
t2756 = ct{1046};
t276 = ct{1047};
t2763 = ct{1048};
t2764 = ct{1049};
t2765 = ct{1050};
t2766 = ct{1051};
t277 = ct{1052};
t2774 = ct{1053};
t2776 = ct{1054};
t2781 = ct{1055};
t2782 = ct{1056};
t2783 = ct{1057};
t2784 = ct{1058};
t2786 = ct{1059};
t2787 = ct{1060};
t2788 = ct{1061};
t2790 = ct{1062};
t28 = ct{1063};
t2802 = ct{1064};
t2803 = ct{1065};
t2804 = ct{1066};
t2806 = ct{1067};
t2807 = ct{1068};
t2812 = ct{1069};
t2813 = ct{1070};
t2819 = ct{1071};
t2820 = ct{1072};
t2821 = ct{1073};
t2825 = ct{1074};
t2828 = ct{1075};
t283 = ct{1076};
t2835 = ct{1077};
t2837 = ct{1078};
t2839 = ct{1079};
t284 = ct{1080};
t2841 = ct{1081};
t2842 = ct{1082};
t2844 = ct{1083};
t285 = ct{1084};
t2857 = ct{1085};
t2859 = ct{1086};
t286 = ct{1087};
t287 = ct{1088};
t2870 = ct{1089};
t2872 = ct{1090};
t2874 = ct{1091};
t2875 = ct{1092};
t2879 = ct{1093};
t288 = ct{1094};
t2880 = ct{1095};
t2883 = ct{1096};
t2884 = ct{1097};
t2886 = ct{1098};
t2887 = ct{1099};
t2888 = ct{1100};
t2889 = ct{1101};
t289 = ct{1102};
t2890 = ct{1103};
t2892 = ct{1104};
t2895 = ct{1105};
t2896 = ct{1106};
t290 = ct{1107};
t2902 = ct{1108};
t2907 = ct{1109};
t2908 = ct{1110};
t2909 = ct{1111};
t291 = ct{1112};
t2912 = ct{1113};
t2913 = ct{1114};
t2916 = ct{1115};
t2918 = ct{1116};
t292 = ct{1117};
t2928 = ct{1118};
t2929 = ct{1119};
t293 = ct{1120};
t2932 = ct{1121};
t2938 = ct{1122};
t294 = ct{1123};
t2945 = ct{1124};
t2946 = ct{1125};
t2949 = ct{1126};
t2950 = ct{1127};
t2951 = ct{1128};
t2952 = ct{1129};
t2954 = ct{1130};
t2955 = ct{1131};
t2956 = ct{1132};
t2957 = ct{1133};
t2958 = ct{1134};
t2959 = ct{1135};
t2960 = ct{1136};
t2961 = ct{1137};
t2967 = ct{1138};
t2969 = ct{1139};
t2975 = ct{1140};
t2977 = ct{1141};
t2982 = ct{1142};
t2988 = ct{1143};
t2992 = ct{1144};
t2995 = ct{1145};
t3 = ct{1146};
t30 = ct{1147};
t3004 = ct{1148};
t3010 = ct{1149};
t3011 = ct{1150};
t3017 = ct{1151};
t3019 = ct{1152};
t3020 = ct{1153};
t3022 = ct{1154};
t3023 = ct{1155};
t3025 = ct{1156};
t3028 = ct{1157};
t3030 = ct{1158};
t3034 = ct{1159};
t3035 = ct{1160};
t3039 = ct{1161};
t304 = ct{1162};
t3047 = ct{1163};
t3048 = ct{1164};
t3051 = ct{1165};
t3055 = ct{1166};
t3058 = ct{1167};
t3059 = ct{1168};
t3060 = ct{1169};
t3063 = ct{1170};
t3065 = ct{1171};
t3067 = ct{1172};
t3068 = ct{1173};
t3074 = ct{1174};
t3075 = ct{1175};
t3077 = ct{1176};
t3078 = ct{1177};
t3081 = ct{1178};
t3085 = ct{1179};
t3088 = ct{1180};
t3090 = ct{1181};
t3105 = ct{1182};
t3109 = ct{1183};
t3111 = ct{1184};
t3117 = ct{1185};
t3120 = ct{1186};
t3124 = ct{1187};
t3130 = ct{1188};
t3132 = ct{1189};
t3134 = ct{1190};
t3135 = ct{1191};
t3136 = ct{1192};
t3138 = ct{1193};
t3153 = ct{1194};
t3165 = ct{1195};
t3170 = ct{1196};
t3173 = ct{1197};
t3177 = ct{1198};
t3181 = ct{1199};
t3182 = ct{1200};
t3186 = ct{1201};
t3188 = ct{1202};
t3191 = ct{1203};
t3194 = ct{1204};
t3199 = ct{1205};
t3200 = ct{1206};
t3201 = ct{1207};
t3204 = ct{1208};
t3210 = ct{1209};
t3212 = ct{1210};
t3218 = ct{1211};
t3235 = ct{1212};
t3237 = ct{1213};
t3243 = ct{1214};
t3247 = ct{1215};
t3248 = ct{1216};
t3249 = ct{1217};
t3256 = ct{1218};
t3260 = ct{1219};
t3265 = ct{1220};
t3266 = ct{1221};
t3269 = ct{1222};
t3272 = ct{1223};
t3285 = ct{1224};
t3291 = ct{1225};
t33 = ct{1226};
t3304 = ct{1227};
t3310 = ct{1228};
t3317 = ct{1229};
t3330 = ct{1230};
t3331 = ct{1231};
t3337 = ct{1232};
t3351 = ct{1233};
t3360 = ct{1234};
t3364 = ct{1235};
t3370 = ct{1236};
t3380 = ct{1237};
t34 = ct{1238};
t3419 = ct{1239};
t3426 = ct{1240};
t3428 = ct{1241};
t3434 = ct{1242};
t3438 = ct{1243};
t3441 = ct{1244};
t3449 = ct{1245};
t3459 = ct{1246};
t346 = ct{1247};
t3469 = ct{1248};
t347 = ct{1249};
t3471 = ct{1250};
t3478 = ct{1251};
t348 = ct{1252};
t3484 = ct{1253};
t3499 = ct{1254};
t35 = ct{1255};
t3504 = ct{1256};
t3520 = ct{1257};
t3521 = ct{1258};
t3522 = ct{1259};
t3527 = ct{1260};
t3531 = ct{1261};
t3565 = ct{1262};
t3580 = ct{1263};
t3581 = ct{1264};
t3644 = ct{1265};
t3701 = ct{1266};
t3704 = ct{1267};
t3709 = ct{1268};
t375 = ct{1269};
t376 = ct{1270};
t377 = ct{1271};
t38 = ct{1272};
t380 = ct{1273};
t381 = ct{1274};
t382 = ct{1275};
t3823 = ct{1276};
t383 = ct{1277};
t3847 = ct{1278};
t3858 = ct{1279};
t3862 = ct{1280};
t3880 = ct{1281};
t3881 = ct{1282};
t3882 = ct{1283};
t3883 = ct{1284};
t390 = ct{1285};
t3902 = ct{1286};
t3908 = ct{1287};
t3909 = ct{1288};
t3916 = ct{1289};
t3926 = ct{1290};
t3930 = ct{1291};
t3931 = ct{1292};
t3932 = ct{1293};
t3937 = ct{1294};
t394 = ct{1295};
t3940 = ct{1296};
t3944 = ct{1297};
t3955 = ct{1298};
t3957 = ct{1299};
t3959 = ct{1300};
t3962 = ct{1301};
t3963 = ct{1302};
t3964 = ct{1303};
t3965 = ct{1304};
t3969 = ct{1305};
t3971 = ct{1306};
t3982 = ct{1307};
t399 = ct{1308};
t3994 = ct{1309};
t3996 = ct{1310};
t3998 = ct{1311};
t4 = ct{1312};
t40 = ct{1313};
t400 = ct{1314};
t4003 = ct{1315};
t4008 = ct{1316};
t401 = ct{1317};
t4014 = ct{1318};
t4033 = ct{1319};
t4038 = ct{1320};
t4042 = ct{1321};
t4054 = ct{1322};
t4061 = ct{1323};
t4070 = ct{1324};
t4078 = ct{1325};
t4081 = ct{1326};
t4090 = ct{1327};
t4098 = ct{1328};
t41 = ct{1329};
t410 = ct{1330};
t411 = ct{1331};
t412 = ct{1332};
t4121 = ct{1333};
t413 = ct{1334};
t414 = ct{1335};
t4141 = ct{1336};
t4142 = ct{1337};
t4143 = ct{1338};
t415 = ct{1339};
t4153 = ct{1340};
t4161 = ct{1341};
t4172 = ct{1342};
t4181 = ct{1343};
t4182 = ct{1344};
t4189 = ct{1345};
t4190 = ct{1346};
t4197 = ct{1347};
t420 = ct{1348};
t421 = ct{1349};
t4210 = ct{1350};
t4218 = ct{1351};
t4234 = ct{1352};
t4235 = ct{1353};
t4236 = ct{1354};
t424 = ct{1355};
t425 = ct{1356};
t4256 = ct{1357};
t4269 = ct{1358};
t4294 = ct{1359};
t4295 = ct{1360};
t4297 = ct{1361};
t4298 = ct{1362};
t430 = ct{1363};
t431 = ct{1364};
t4323 = ct{1365};
t433 = ct{1366};
t434 = ct{1367};
t4349 = ct{1368};
t4355 = ct{1369};
t436 = ct{1370};
t4363 = ct{1371};
t44 = ct{1372};
t445 = ct{1373};
t4474 = ct{1374};
t4475 = ct{1375};
t448 = ct{1376};
t450 = ct{1377};
t4509 = ct{1378};
t451 = ct{1379};
t456 = ct{1380};
t459 = ct{1381};
t4597 = ct{1382};
t4598 = ct{1383};
t4599 = ct{1384};
t46 = ct{1385};
t4603 = ct{1386};
t463 = ct{1387};
t465 = ct{1388};
t466 = ct{1389};
t4752 = ct{1390};
t478 = ct{1391};
t479 = ct{1392};
t48 = ct{1393};
t480 = ct{1394};
t482 = ct{1395};
t483 = ct{1396};
t484 = ct{1397};
t485 = ct{1398};
t487 = ct{1399};
t488 = ct{1400};
t49 = ct{1401};
t491 = ct{1402};
t495 = ct{1403};
t496 = ct{1404};
t5 = ct{1405};
t50 = ct{1406};
t501 = ct{1407};
t502 = ct{1408};
t504 = ct{1409};
t505 = ct{1410};
t506 = ct{1411};
t51 = ct{1412};
t514 = ct{1413};
t519 = ct{1414};
t523 = ct{1415};
t524 = ct{1416};
t527 = ct{1417};
t530 = ct{1418};
t532 = ct{1419};
t533 = ct{1420};
t534 = ct{1421};
t537 = ct{1422};
t539 = ct{1423};
t54 = ct{1424};
t541 = ct{1425};
t542 = ct{1426};
t544 = ct{1427};
t545 = ct{1428};
t546 = ct{1429};
t547 = ct{1430};
t55 = ct{1431};
t550 = ct{1432};
t553 = ct{1433};
t555 = ct{1434};
t557 = ct{1435};
t558 = ct{1436};
t559 = ct{1437};
t56 = ct{1438};
t560 = ct{1439};
t561 = ct{1440};
t563 = ct{1441};
t568 = ct{1442};
t569 = ct{1443};
t57 = ct{1444};
t572 = ct{1445};
t573 = ct{1446};
t574 = ct{1447};
t575 = ct{1448};
t578 = ct{1449};
t581 = ct{1450};
t584 = ct{1451};
t587 = ct{1452};
t59 = ct{1453};
t595 = ct{1454};
t6 = ct{1455};
t602 = ct{1456};
t603 = ct{1457};
t61 = ct{1458};
t614 = ct{1459};
t623 = ct{1460};
t624 = ct{1461};
t627 = ct{1462};
t628 = ct{1463};
t629 = ct{1464};
t631 = ct{1465};
t632 = ct{1466};
t634 = ct{1467};
t641 = ct{1468};
t643 = ct{1469};
t644 = ct{1470};
t646 = ct{1471};
t648 = ct{1472};
t649 = ct{1473};
t65 = ct{1474};
t650 = ct{1475};
t651 = ct{1476};
t652 = ct{1477};
t653 = ct{1478};
t654 = ct{1479};
t655 = ct{1480};
t657 = ct{1481};
t662 = ct{1482};
t663 = ct{1483};
t664 = ct{1484};
t665 = ct{1485};
t666 = ct{1486};
t667 = ct{1487};
t668 = ct{1488};
t669 = ct{1489};
t672 = ct{1490};
t674 = ct{1491};
t675 = ct{1492};
t676 = ct{1493};
t68 = ct{1494};
t69 = ct{1495};
t693 = ct{1496};
t699 = ct{1497};
t7 = ct{1498};
t701 = ct{1499};
t71 = ct{1500};
t720 = ct{1501};
t721 = ct{1502};
t722 = ct{1503};
t724 = ct{1504};
t73 = ct{1505};
t731 = ct{1506};
t732 = ct{1507};
t735 = ct{1508};
t736 = ct{1509};
t741 = ct{1510};
t742 = ct{1511};
t743 = ct{1512};
t744 = ct{1513};
t746 = ct{1514};
t749 = ct{1515};
t750 = ct{1516};
t751 = ct{1517};
t752 = ct{1518};
t753 = ct{1519};
t754 = ct{1520};
t755 = ct{1521};
t756 = ct{1522};
t757 = ct{1523};
t759 = ct{1524};
t760 = ct{1525};
t761 = ct{1526};
t762 = ct{1527};
t764 = ct{1528};
t765 = ct{1529};
t768 = ct{1530};
t769 = ct{1531};
t772 = ct{1532};
t774 = ct{1533};
t776 = ct{1534};
t778 = ct{1535};
t779 = ct{1536};
t792 = ct{1537};
t794 = ct{1538};
t795 = ct{1539};
t797 = ct{1540};
t799 = ct{1541};
t8 = ct{1542};
t801 = ct{1543};
t802 = ct{1544};
t803 = ct{1545};
t804 = ct{1546};
t805 = ct{1547};
t806 = ct{1548};
t811 = ct{1549};
t817 = ct{1550};
t818 = ct{1551};
t819 = ct{1552};
t820 = ct{1553};
t821 = ct{1554};
t822 = ct{1555};
t823 = ct{1556};
t824 = ct{1557};
t826 = ct{1558};
t828 = ct{1559};
t829 = ct{1560};
t830 = ct{1561};
t831 = ct{1562};
t833 = ct{1563};
t834 = ct{1564};
t835 = ct{1565};
t836 = ct{1566};
t837 = ct{1567};
t838 = ct{1568};
t839 = ct{1569};
t841 = ct{1570};
t842 = ct{1571};
t843 = ct{1572};
t844 = ct{1573};
t845 = ct{1574};
t846 = ct{1575};
t847 = ct{1576};
t848 = ct{1577};
t850 = ct{1578};
t851 = ct{1579};
t852 = ct{1580};
t853 = ct{1581};
t854 = ct{1582};
t855 = ct{1583};
t858 = ct{1584};
t859 = ct{1585};
t862 = ct{1586};
t863 = ct{1587};
t864 = ct{1588};
t865 = ct{1589};
t867 = ct{1590};
t868 = ct{1591};
t869 = ct{1592};
t870 = ct{1593};
t871 = ct{1594};
t872 = ct{1595};
t873 = ct{1596};
t874 = ct{1597};
t875 = ct{1598};
t876 = ct{1599};
t877 = ct{1600};
t879 = ct{1601};
t881 = ct{1602};
t882 = ct{1603};
t884 = ct{1604};
t885 = ct{1605};
t886 = ct{1606};
t887 = ct{1607};
t888 = ct{1608};
t889 = ct{1609};
t890 = ct{1610};
t891 = ct{1611};
t892 = ct{1612};
t893 = ct{1613};
t894 = ct{1614};
t895 = ct{1615};
t896 = ct{1616};
t897 = ct{1617};
t898 = ct{1618};
t9 = ct{1619};
t900 = ct{1620};
t901 = ct{1621};
t902 = ct{1622};
t903 = ct{1623};
t904 = ct{1624};
t906 = ct{1625};
t907 = ct{1626};
t908 = ct{1627};
t909 = ct{1628};
t910 = ct{1629};
t912 = ct{1630};
t913 = ct{1631};
t914 = ct{1632};
t915 = ct{1633};
t916 = ct{1634};
t917 = ct{1635};
t918 = ct{1636};
t919 = ct{1637};
t923 = ct{1638};
t924 = ct{1639};
t925 = ct{1640};
t926 = ct{1641};
t927 = ct{1642};
t928 = ct{1643};
t933 = ct{1644};
t934 = ct{1645};
t936 = ct{1646};
t941 = ct{1647};
t947 = ct{1648};
t948 = ct{1649};
t949 = ct{1650};
t950 = ct{1651};
t951 = ct{1652};
t952 = ct{1653};
t953 = ct{1654};
t954 = ct{1655};
t955 = ct{1656};
t956 = ct{1657};
t957 = ct{1658};
t964 = ct{1659};
t965 = ct{1660};
t966 = ct{1661};
t968 = ct{1662};
t970 = ct{1663};
t972 = ct{1664};
t973 = ct{1665};
t974 = ct{1666};
t976 = ct{1667};
t977 = ct{1668};
t979 = ct{1669};
t980 = ct{1670};
t983 = ct{1671};
t985 = ct{1672};
t986 = ct{1673};
t987 = ct{1674};
t990 = ct{1675};
t991 = ct{1676};
t992 = ct{1677};
t993 = ct{1678};
t994 = ct{1679};
t995 = ct{1680};
t996 = ct{1681};
t1719 = Mm.*t5.*t30.*t1470;
t1721 = Mm.*t5.*t34.*t1470;
t1725 = B_cg_H.*Mb.*t420.*t1178;
t1729 = -t1672;
t1730 = t1646./2.0;
t1735 = Mm.*t420.*t1221;
t1736 = Mm.*t421.*t1221;
t1746 = Mb.*t15.*t675.*t964;
t1748 = B_cg_H.*Mb.*t5.*t38.*t1512;
t1750 = -t964.*(t105-t465);
t1753 = t903.*t977;
t1756 = -t977.*(t105-t465);
t1767 = -t1701;
t1768 = -t1702;
t1772 = -t1706;
t1774 = t35.*t38.*t1512;
t1776 = -t1716;
t1783 = B_cg_H.*Mb.*t5.*t33.*t1512;
t1785 = t1694./2.0;
t1789 = t1701./2.0;
t1790 = t1702./2.0;
t1793 = t1706./2.0;
t1794 = t1707./2.0;
t1795 = t1708./2.0;
t1797 = t1710./2.0;
t1811 = t4.*t871.*t964;
t1816 = t8.*t872.*t964;
t1821 = -t977.*(t103-t544);
t1827 = -t1759;
t1828 = -t1760;
t1831 = -t1764;
t1842 = Mt.*t381.*t1381;
t1845 = t964.*(t105-t465).*(-1.0./2.0);
t1846 = t1817.*(-1.0./2.0);
t1849 = t977.*(t105-t465).*(-1.0./2.0);
t1850 = t1826.*(-1.0./2.0);
t1857 = Mb.*t4.*t5.*t1660;
t1859 = Mm.*t382.*t1394;
t1860 = Mb.*t5.*t9.*t1676;
t1863 = -t1813;
t1864 = t1817./2.0;
t1870 = t1826./2.0;
t1872 = -t1851;
t1877 = Mt.*t421.*t1381;
t1882 = t1813./2.0;
t1883 = t817.*t1178;
t1887 = t1819./2.0;
t1890 = t977.*(t103-t544).*(-1.0./2.0);
t1891 = t11.*t381.*t1430;
t1893 = t1824./2.0;
t1898 = Mm.*t657.*t1221;
t1900 = Mm.*t420.*t1394;
t1901 = Mm.*t381.*t1470;
t1917 = t495.*t1390;
t1924 = -t1178.*(t105-t465);
t1927 = t496.*t1430;
t1929 = B_cg_H.*Mb.*t495.*t1382;
t1935 = t11.*t420.*t1430;
t1937 = t11.*t381.*t1512;
t1938 = t465.*t1512;
t1939 = B_cg_H.*Mb.*t485.*t1362;
t1943 = -t1897;
t1944 = Mm.*t421.*t1470;
t1950 = -t1903;
t1951 = B_cg_H.*Mb.*t381.*t1512;
t1952 = B_cg_H.*Mb.*t382.*t1512;
t1953 = t487.*t1430;
t1955 = t903.*t1178;
t1957 = t903.*t1180;
t1968 = -t1936;
t1976 = t555.*t1390;
t1977 = Mb.*t15.*t964.*t977;
t1980 = -t1954;
t1986 = -t1958;
t1994 = t11.*t545.*t1430;
t1995 = t496.*t1512;
t2000 = t6.*t420.*t1512;
t2005 = t11.*t420.*t1512;
t2016 = B_cg_H.*Mb.*t420.*t1512;
t2017 = B_cg_H.*Mb.*t421.*t1512;
t2020 = B_cg_H.*Mb.*t555.*t1382;
t2021 = t9.*t495.*t1430;
t2023 = B_cg_H.*Mb.*t557.*t1382;
t2024 = B_cg_H.*Mb.*t558.*t1382;
t2029 = t487.*t1512;
t2033 = t1178.*(t105-t465).*(-1.0./2.0);
t2034 = t1990.*(-1.0./2.0);
t2060 = Mb.*t10.*t1918;
t2061 = Mb.*t15.*t964.*t1037;
t2075 = t1956./2.0;
t2079 = t1990./2.0;
t2081 = -t2037;
t2083 = t568.*t1512;
t2084 = t569.*t1512;
t2099 = t964.*t1179;
t2100 = -t1178.*(t197-t537);
t2103 = t9.*t555.*t1430;
t2106 = Mm.*t657.*t1394;
t2108 = -t2015;
t2116 = t262+t479+t563+t649;
t2123 = t8.*t575.*t1430;
t2136 = Mb.*t2.*t5.*t1918;
t2140 = Mb.*t381.*t1660;
t2142 = Mb.*t5.*t7.*t1918;
t2149 = Mb.*t382.*t1676;
t2174 = t448+t826+t956;
t2185 = t804.*t1430;
t2187 = t1044.*t1178;
t2189 = Mm.*t651.*t1470;
t2191 = t819.*t1390;
t2206 = B_cg_H.*Mb.*t819.*t1382;
t2216 = Mb.*t421.*t1660;
t2221 = t2.*t2148;
t2223 = t7.*t2148;
t2228 = -t2148;
t2229 = Mb.*t420.*t1676;
t2233 = t1178.*(t197-t537).*(-1.0./2.0);
t2239 = t817.*t1430;
t2258 = -t2215;
t2260 = -t2220;
t2267 = -t2180;
t2271 = t868.*t1390;
t2274 = t871.*t1390;
t2275 = Mm.*t1007.*t1221;
t2281 = -t2196;
t2285 = Mm.*t1016.*t1221;
t2286 = Mb.*t11.*t15.*t542.*t1512;
t2293 = B_cg_H.*Mb.*t871.*t1362;
t2296 = -t2225;
t2297 = t2180./2.0;
t2299 = -t2231;
t2309 = t903.*t1430;
t2310 = t8.*t818.*t1430;
t2314 = -t1430.*(t105-t465);
t2315 = t9.*t819.*t1430;
t2316 = Mb.*t926.*t1382;
t2317 = t817.*t1512;
t2318 = -t2283;
t2334 = Mb.*t15.*t721.*t1512;
t2348 = Mb.*t11.*t15.*t641.*t1512;
t2353 = -t2294;
t2354 = Mt.*t10.*t2240;
t2357 = -t2298;
t2366 = t9.*t868.*t1430;
t2369 = -t1430.*(t103-t544);
t2371 = t9.*t871.*t1430;
t2372 = t3.*t873.*t1430;
t2375 = t903.*t1512;
t2378 = t8.*t873.*t1430;
t2380 = -t1512.*(t105-t465);
t2382 = -t2347;
t2402 = t1367.*3.36554e-3;
t2403 = -t2359;
t2417 = t1430.*(t105-t465).*(-1.0./2.0);
t2421 = t466+t879+t1095;
t2422 = -t2383;
t2423 = -t2387;
t2424 = Mt.*t2.*t5.*t2240;
t2425 = Mt.*t5.*t7.*t2240;
t2426 = t2.*t2356;
t2428 = t7.*t2356;
t2432 = -t1430.*(t197-t537);
t2436 = t977.*t1430;
t2438 = -t2404;
t2455 = -t1512.*(t103-t544);
t2456 = t9.*t871.*t1512;
t2458 = -t2379;
t2460 = t8.*t873.*t1512;
t2465 = Mm.*t1016.*t1394;
t2470 = t1424.*3.36554e-3;
t2471 = -t2390;
t2472 = t1425.*3.36554e-3;
t2473 = t1426.*3.36554e-3;
t2483 = t1432.*3.36554e-3;
t2484 = t1430.*(t197-t537).*-2.0;
t2502 = t1430.*(t103-t544).*(-1.0./2.0);
t2513 = t1512.*(t105-t465).*(-1.0./2.0);
t2525 = -t2427;
t2528 = -t2475;
t2529 = t1037.*t1430;
t2533 = -t2429;
t2535 = -t2482;
t2536 = t964.*t1512;
t2540 = t1044.*t1430;
t2543 = -t2487;
t2547 = -t2493;
t2550 = -t2494;
t2551 = -t2495;
t2552 = -t2497;
t2567 = Mm.*t1009.*t1470;
t2568 = t1488.*3.36554e-3;
t2579 = t2539.*(-1.0./2.0);
t2592 = t1367.*3.372786875e-3;
t2605 = t1367.*9.53094055e-4;
t2610 = t1512.*(t103-t544).*(-1.0./2.0);
t2628 = dth1.*t2527;
t2635 = t1031.*t1512;
t2637 = Mb.*t15.*t925.*t1512;
t2640 = t2539./2.0;
t2646 = dth1.*t2563;
t2647 = -t2587;
t2648 = -t2586;
t2649 = -t2591;
t2656 = -t2604;
t2657 = -t2603;
t2658 = -t2608;
t2677 = t1424.*3.372786875e-3;
t2679 = t1425.*3.372786875e-3;
t2680 = t1426.*3.372786875e-3;
t2683 = t1424.*9.53094055e-4;
t2687 = t1425.*9.53094055e-4;
t2688 = t1426.*9.53094055e-4;
t2696 = t1432.*3.372786875e-3;
t2703 = t1432.*9.53094055e-4;
t2725 = -t2626;
t2735 = Mb.*t15.*t1430.*(t197-t537);
t2743 = -t2693;
t2744 = -t2694;
t2746 = -Mb.*t15.*t1512.*(t214-t541);
t2747 = -t2700;
t2748 = -t2701;
t2750 = -t2708;
t2754 = -t2712;
t2755 = -t2713;
t2757 = B_cg_H.*Mb.*t485.*t1918;
t2758 = -t2719;
t2759 = -t2720;
t2760 = -t2721;
t2761 = -t2722;
t2762 = -t2724;
t2768 = t1488.*3.372786875e-3;
t2769 = t1488.*9.53094055e-4;
t2770 = t1178.*t1430;
t2771 = t1179.*t1430;
t2778 = Mm.*t1170.*t1394;
t2792 = Mb.*t4.*t5.*t2563;
t2797 = t1646.*3.36554e-3;
t2799 = Mb.*t9.*t10.*t2563;
t2811 = Mb.*t15.*t1047.*t1512;
t2816 = Mb.*t4.*t10.*t2527;
t2817 = Mb.*t5.*t9.*t2527;
t2823 = t380.*t2264;
t2824 = t380.*t2266;
t2830 = -t1430.*(t539+t641);
t2832 = -t2803;
t2833 = t1178.*t1512;
t2836 = Mm.*t1169.*t1470;
t2838 = -t2812;
t2843 = -B_cg_H.*Mb.*t1676.*(t197-t537);
t2845 = -t2820;
t2846 = t1694.*3.36554e-3;
t2847 = Mb.*t5.*t33.*t2563;
t2849 = Mb.*t5.*t38.*t2563;
t2855 = t1701.*3.36554e-3;
t2856 = t1702.*3.36554e-3;
t2863 = t1706.*3.36554e-3;
t2864 = t1707.*3.36554e-3;
t2865 = t1708.*3.36554e-3;
t2869 = Mb.*t5.*t9.*t2627;
t2871 = t1710.*3.36554e-3;
t2876 = Mb.*t5.*t30.*t2527;
t2877 = B_cg_H.*Mb.*t964.*t1660;
t2878 = Mb.*t5.*t34.*t2527;
t2885 = Mb.*t4.*t5.*t2638;
t2906 = -t1512.*(t534-t546);
t2915 = t829+t833+t1217;
t2917 = B_cg_H.*Mb.*t1676.*(t197-t537);
t2919 = t964.*(t105-t465).*(-3.36554e-3);
t2920 = t1817.*(-3.36554e-3);
t2926 = t977.*(t105-t465).*(-3.36554e-3);
t2927 = t1826.*(-3.36554e-3);
t2931 = Mt.*t4.*t5.*t2763;
t2940 = t1430.*(t539+t641).*(-1.0./2.0);
t2944 = -t2908;
t2953 = Mt.*t5.*t9.*t2730;
t2962 = t1646.*3.367829185e-3;
t2963 = -t2888;
t2964 = t1817.*3.36554e-3;
t2966 = t1826.*3.36554e-3;
t2976 = -t2945;
t2978 = Mb.*t1362.*t1382;
t2979 = -t2958;
t2983 = t1813.*3.36554e-3;
t2989 = t1819.*3.36554e-3;
t2990 = t977.*(t103-t544).*(-3.36554e-3);
t2991 = t1824.*3.36554e-3;
t2994 = t1646.*8.56645e-6;
t3001 = t1701.*3.372786875e-3;
t3002 = t1702.*3.372786875e-3;
t3003 = t1512.*(t534-t546).*(-1.0./2.0);
t3005 = t1706.*3.372786875e-3;
t3006 = t1707.*3.372786875e-3;
t3007 = t1708.*3.372786875e-3;
t3008 = t1701.*9.53094055e-4;
t3009 = t1702.*9.53094055e-4;
t3012 = t1710.*3.372786875e-3;
t3013 = t1706.*9.53094055e-4;
t3014 = t1707.*9.53094055e-4;
t3015 = t1708.*9.53094055e-4;
t3016 = t1694.*3.367829185e-3;
t3021 = t1710.*9.53094055e-4;
t3037 = t977.*(t103-t544).*3.36554e-3;
t3053 = B_cg_H.*Mb.*t871.*t1918;
t3054 = t1694.*8.56645e-6;
t3061 = t964.*(t105-t465).*(-3.372786875e-3);
t3062 = t1817.*(-3.372786875e-3);
t3069 = t964.*(t105-t465).*(-9.53094055e-4);
t3070 = t1817.*(-9.53094055e-4);
t3083 = t977.*(t105-t465).*(-3.367829185e-3);
t3084 = t1826.*(-3.367829185e-3);
t3089 = -t3055;
t3091 = Mb.*t381.*t2563;
t3092 = Mb.*t382.*t2563;
t3094 = -t3034;
t3098 = -t3058;
t3100 = t1817.*3.372786875e-3;
t3102 = t1817.*9.53094055e-4;
t3106 = Mb.*t381.*t2527;
t3107 = Mb.*t382.*t2527;
t3108 = t1826.*3.367829185e-3;
t3112 = -t3088;
t3115 = t977.*(t105-t465).*(-8.56645e-6);
t3116 = t1826.*(-8.56645e-6);
t3118 = t1813.*3.372786875e-3;
t3125 = t1813.*9.53094055e-4;
t3127 = t1819.*3.372786875e-3;
t3129 = t1430.*t1512;
t3133 = t1819.*9.53094055e-4;
t3140 = t977.*(t103-t544).*(-3.367829185e-3);
t3141 = t1824.*3.367829185e-3;
t3146 = t1956.*3.36554e-3;
t3148 = Mb.*t420.*t2563;
t3149 = Mb.*t421.*t2563;
t3151 = t1178.*(t105-t465).*(-3.36554e-3);
t3152 = t1990.*(-3.36554e-3);
t3157 = t1826.*8.56645e-6;
t3159 = Mb.*t382.*t2627;
t3160 = -t3120;
t3171 = Mb.*t420.*t2527;
t3172 = Mb.*t421.*t2527;
t3174 = t977.*(t103-t544).*3.367829185e-3;
t3175 = Mb.*t381.*t2638;
t3180 = -t3111;
t3184 = t1990.*3.36554e-3;
t3187 = t977.*(t103-t544).*(-8.56645e-6);
t3189 = t1824.*8.56645e-6;
t3203 = dphi1.*t3138;
t3220 = -t3186;
t3222 = Mt.*t381.*t2763;
t3224 = -t3188;
t3226 = -t3191;
t3228 = Mb.*t420.*t2627;
t3233 = -t3194;
t3238 = -t3199;
t3241 = -t3201;
t3242 = Mt.*t382.*t2730;
t3246 = Mb.*t421.*t2638;
t3263 = B_cg_H.*Mb.*t11.*t459.*t2527;
t3274 = Mt.*t421.*t2763;
t3277 = t1956.*3.372786875e-3;
t3284 = t1178.*(t105-t465).*(-3.372786875e-3);
t3286 = t1956.*9.53094055e-4;
t3290 = t1178.*(t105-t465).*(-9.53094055e-4);
t3294 = Mt.*t420.*t2730;
t3297 = t1990.*(-3.367829185e-3);
t3305 = t1178.*(t197-t537).*(-3.36554e-3);
t3318 = t646+t741+t936+t973;
t3319 = -t3269;
t3321 = B_cg_H.*Mb.*t11.*t542.*t2563;
t3322 = Mb.*t4.*t10.*t3138;
t3323 = Mb.*t5.*t9.*t3138;
t3325 = -t3256;
t3332 = t1990.*3.367829185e-3;
t3339 = -t3265;
t3341 = -t3310;
t3383 = t2180.*3.36554e-3;
t3394 = t1990.*(-8.56645e-6);
t3403 = B_cg_H.*Mb.*t675.*t2527;
t3415 = B_cg_H.*Mb.*t721.*t2563;
t3416 = Mb.*t5.*t30.*t3138;
t3417 = Mb.*t5.*t34.*t3138;
t3420 = t1990.*8.56645e-6;
t3453 = t1178.*(t197-t537).*(-9.52624335e-4);
t3457 = t1178.*(t197-t537).*(-3.372816795e-3);
t3474 = -t3428;
t3483 = t23+t40+t852+t2240;
t3487 = B_cg_H.*Mb.*t1512.*t1676;
t3495 = t1430.*(t105-t465).*(-3.36554e-3);
t3503 = t2180.*9.52624335e-4;
t3505 = t2180.*3.372816795e-3;
t3523 = t380.*t3067;
t3524 = t380.*t3068;
t3539 = t1430.*(t103-t544).*(-3.36554e-3);
t3547 = t1512.*(t105-t465).*(-3.36554e-3);
t3548 = t3471./2.0;
t3551 = t1430.*(t197-t537).*(-6.73108e-3);
t3559 = t1512.*(t105-t465).*3.36554e-3;
t3562 = t1430.*(t105-t465).*(-3.372786875e-3);
t3569 = t1430.*(t105-t465).*(-9.53094055e-4);
t3577 = Mb.*t1382.*t1918;
t3583 = t2539.*(-3.36554e-3);
t3595 = t1512.*(t103-t544).*(-3.36554e-3);
t3609 = B_cg_H.*Mb.*t925.*t2563;
t3611 = t2539.*3.36554e-3;
t3617 = Mb.*t381.*t3138;
t3619 = Mb.*t382.*t3138;
t3635 = t1430.*(t103-t544).*(-9.53094055e-4);
t3639 = t1512.*(t105-t465).*(-3.372786875e-3);
t3643 = t1512.*(t105-t465).*(-9.53094055e-4);
t3650 = t1512.*(t105-t465).*(-3.367829185e-3);
t3657 = Mb.*t1362.*t1981;
t3666 = t1430.*(t103-t544).*(-3.372786875e-3);
t3671 = -B_cg_H.*Mb.*t2527.*(t197-t537);
t3672 = B_cg_H.*Mb.*t977.*t2527;
t3677 = t1512.*(t105-t465).*3.367829185e-3;
t3678 = B_cg_H.*Mb.*t964.*t2563;
t3680 = -B_cg_H.*Mb.*t2563.*(t214-t541);
t3683 = Mb.*t420.*t3138;
t3684 = Mb.*t421.*t3138;
t3699 = t2.*t3644;
t3702 = t7.*t3644;
t3706 = -t3644;
t3708 = t1512.*(t103-t544).*(-3.367829185e-3);
t3713 = t1430.*(t197-t537).*(-1.90524867e-3);
t3715 = t2539.*(-9.52624335e-4);
t3717 = t1430.*(t197-t537).*(-6.74563359e-3);
t3721 = t2539.*(-3.372816795e-3);
t3730 = t1512.*(t105-t465).*(-8.56645e-6);
t3739 = B_cg_H.*Mb.*t1037.*t2527;
t3740 = -B_cg_H.*Mb.*t2527.*(t195-t634);
t3743 = B_cg_H.*Mb.*t964.*t2638;
t3749 = B_cg_H.*Mb.*t1047.*t2563;
t3750 = -B_cg_H.*Mb.*t2627.*(t197-t537);
t3752 = t2539.*9.52624335e-4;
t3761 = t2539.*3.372816795e-3;
t3768 = -t3704;
t3769 = -t3709;
t3771 = t480.*t3182;
t3772 = t485.*t3182;
t3787 = B_cg_H.*Mb.*t11.*t459.*t3138;
t3790 = t1512.*(t103-t544).*(-8.56645e-6);
t3791 = t1512.*t2031;
t3792 = B_cg_H.*Mb.*t2527.*(t195-t634);
t3819 = t1430.*(t539+t641).*(-3.36554e-3);
t3828 = B_cg_H.*Mb.*t675.*t3138;
t3832 = B_cg_H.*Mb.*t1178.*t2563;
t3835 = B_cg_H.*Mb.*t1179.*t2527;
t3842 = t1512.*(t534-t546).*(-3.36554e-3);
t3855 = Mt.*t1531.*t2240;
t3866 = t1430.*(t539+t641).*(-9.52624335e-4);
t3873 = t1430.*(t539+t641).*(-3.372816795e-3);
t3900 = t868.*t3182;
t3906 = t870.*t3182;
t3907 = t871.*t3182;
t3910 = t1512.*(t534-t546).*(-9.52624335e-4);
t3913 = t1512.*(t534-t546).*(-3.372816795e-3);
t3915 = -t3881;
t3917 = -t1512.*(t273-t602-t742+t743);
t3928 = -t3908;
t3929 = -t3909;
t3933 = -t3916;
t3936 = t1512.*(t273-t602-t742+t743);
t3942 = -t977.*(-t488+t603+dpsi1.*(t105-t465)+dth2.*(t103-t544));
t3952 = -B_cg_H.*Mb.*t3138.*(t197-t537);
t3956 = B_cg_H.*Mb.*t977.*t3138;
t3960 = dth1.*t3937;
t3961 = t532+t1708+t1714;
t3967 = t533+t1710+t1717;
t3968 = dth1.*t3940;
t3974 = B_cg_H.*Mb.*t1037.*t3138;
t3976 = -B_cg_H.*Mb.*t3138.*(t195-t634);
t3981 = B_cg_H.*Mb.*t3138.*(t197-t537);
t3983 = t3235.*3.36554e-3;
t3993 = B_cg_H.*Mb.*t1512.*t2527;
t3995 = -t3963;
t4004 = t3265.*3.36554e-3;
t4012 = B_cg_H.*Mb.*t1512.*t2627;
t4028 = Mt.*t4.*t10.*t3940;
t4029 = Mt.*t5.*t9.*t3940;
t4035 = Mt.*t4.*t5.*t3937;
t4036 = Mt.*t9.*t10.*t3937;
t4047 = Mb.*t1660.*t2527;
t4048 = B_cg_H.*Mb.*t1179.*t3138;
t4049 = Mt.*t4.*t5.*t3971;
t4051 = Mt.*t5.*t33.*t3937;
t4052 = Mt.*t5.*t38.*t3937;
t4056 = Mt.*t5.*t30.*t3940;
t4058 = Mt.*t5.*t34.*t3940;
t4059 = Mb.*t1676.*t2563;
t4060 = Mt.*t5.*t9.*t3969;
t4064 = t3471.*3.36554e-3;
t4068 = -t4054;
t4073 = t3521.*3.36554e-3;
t4074 = t3522.*3.36554e-3;
t4086 = t3471.*3.372786875e-3;
t4087 = t3471.*9.53094055e-4;
t4088 = dy.*t4078;
t4089 = dz.*t4081;
t4092 = Mt.*t381.*t3937;
t4093 = Mt.*t382.*t3937;
C = ft_6({B_cg_H,ITail,Mb,Mm,Mt,T_cg_H,dphi1,dphi2,dpsi1,dth1,dth2,dx,dy,dz,t10,t1003,t1004,t1005,t1006,t1007,t1008,t1009,t1010,t1011,t1012,t1013,t1014,t1015,t1016,t1017,t1018,t1019,t1020,t1021,t1023,t1024,t1025,t1026,t1029,t103,t1030,t1031,t1036,t1037,t1041,t1042,t1043,t1044,t1045,t1046,t1047,t1049,t105,t1050,t1051,t1052,t1053,t1054,t1055,t1056,t1057,t1058,t1059,t1060,t1061,t1062,t1063,t1064,t1065,t1067,t1068,t1071,t1072,t1073,t1074,t1075,t1076,t1077,t1078,t1079,t1080,t1081,t1082,t1084,t1085,t1086,t1088,t1093,t1097,t11,t1102,t1105,t1108,t1109,t1113,t1114,t1115,t1116,t1117,t1118,t1119,t1120,t1121,t1122,t1123,t1124,t1125,t1126,t1127,t1128,t1129,t1130,t1131,t1132,t1133,t1134,t1135,t1136,t1137,t1138,t1139,t1140,t1141,t1142,t1143,t1144,t1145,t1146,t1147,t1148,t1149,t1150,t1152,t1153,t1154,t1155,t1156,t1157,t1158,t1159,t1160,t1161,t1162,t1163,t1164,t1165,t1166,t1167,t1168,t1169,t1170,t1171,t1172,t1173,t1174,t1176,t1177,t1178,t1179,t1181,t1182,t1183,t1184,t1185,t1186,t1187,t1188,t1189,t1190,t1191,t1192,t1193,t1194,t1195,t1196,t1197,t1199,t120,t1200,t1201,t1202,t1203,t1205,t1206,t1207,t1209,t1211,t1212,t1213,t1214,t1215,t1216,t1218,t1221,t1223,t1224,t1225,t1226,t1227,t1228,t1229,t123,t1230,t1231,t1232,t1234,t1235,t1236,t1237,t1238,t1240,t1242,t1243,t1244,t1245,t1246,t1247,t1248,t1250,t1251,t1252,t1253,t1255,t1256,t1257,t1260,t1261,t1262,t1263,t1264,t1265,t1266,t1268,t1270,t1272,t1275,t1279,t1280,t1282,t1283,t1284,t1285,t1287,t1289,t1296,t130,t1301,t1302,t1303,t1304,t1305,t1306,t1307,t1308,t1309,t1311,t1312,t1313,t1319,t1320,t1322,t1323,t1324,t1325,t1328,t1329,t1331,t1332,t1334,t1335,t1337,t1338,t134,t1340,t1341,t1342,t1343,t1344,t1345,t1348,t1349,t1352,t1354,t1355,t1356,t1357,t1358,t1360,t1361,t1362,t1363,t1365,t1366,t1367,t1368,t1370,t1371,t1372,t1373,t1374,t1377,t1378,t1379,t1380,t1381,t1382,t1383,t1384,t1385,t1386,t1388,t1389,t1391,t1393,t1394,t1395,t1396,t1397,t1399,t1400,t1402,t1403,t1405,t1406,t1407,t1408,t1409,t1410,t1412,t1413,t1414,t1415,t1416,t1418,t1419,t1421,t1422,t1424,t1426,t1427,t1429,t1430,t1431,t1432,t1433,t1434,t1435,t1437,t1438,t1439,t144,t1440,t1441,t1442,t1443,t1444,t1445,t1446,t1447,t1448,t1450,t1451,t1453,t1454,t1455,t1456,t1457,t1458,t1459,t1460,t1461,t1462,t1463,t1465,t1466,t1467,t1468,t1469,t1470,t1471,t1472,t1475,t1476,t1477,t1478,t1479,t1481,t1482,t1483,t1484,t1486,t1487,t1488,t1489,t1491,t1492,t1493,t1494,t1495,t1496,t1497,t1498,t15,t1500,t1501,t1503,t1504,t1505,t1506,t1507,t1508,t1509,t1511,t1512,t1513,t1514,t1515,t1516,t1517,t1518,t1520,t1521,t1522,t1523,t1524,t1525,t1526,t1527,t1528,t1529,t1531,t1532,t1533,t1534,t1535,t1536,t1537,t1539,t1540,t1541,t1542,t1543,t1547,t1548,t1549,t1550,t1552,t1553,t1555,t1557,t1559,t1560,t1561,t1562,t1563,t1565,t1566,t1567,t1568,t1572,t1573,t1576,t1577,t1580,t1581,t1582,t1585,t1587,t1588,t1589,t1591,t1592,t1593,t1594,t1595,t1596,t1597,t1598,t1599,t160,t1600,t1601,t1602,t1603,t1605,t1606,t1609,t161,t1610,t1613,t1614,t1615,t1616,t1617,t1618,t1619,t162,t1620,t1621,t1624,t1627,t1628,t1632,t1635,t1636,t1637,t1639,t1640,t1641,t1642,t1644,t1645,t1646,t1647,t1648,t1649,t1651,t1652,t1653,t1654,t1655,t1656,t1657,t1658,t1659,t1660,t1661,t1663,t1664,t1665,t1667,t1668,t1669,t1670,t1671,t1672,t1673,t1674,t1675,t1676,t1677,t1678,t1679,t1680,t1681,t1682,t1683,t1684,t1685,t1686,t1687,t1688,t1689,t1690,t1691,t1692,t1693,t1694,t1695,t1698,t1699,t1700,t1701,t1702,t1703,t1704,t1705,t1706,t1707,t1709,t1711,t1712,t1715,t1716,t1718,t1719,t1721,t1723,t1725,t1726,t1727,t1729,t1730,t1731,t1732,t1733,t1734,t1735,t1736,t1737,t1741,t1742,t1743,t1744,t1745,t1746,t1747,t1748,t1749,t1750,t1751,t1753,t1756,t1758,t1759,t1760,t1761,t1762,t1764,t1765,t1767,t1768,t1769,t1770,t1772,t1773,t1774,t1775,t1776,t1777,t1783,t1784,t1785,t1786,t1788,t1789,t1790,t1791,t1793,t1794,t1795,t1796,t1797,t1798,t1799,t1801,t1802,t1803,t1805,t1806,t1808,t1810,t1811,t1812,t1813,t1814,t1815,t1816,t1817,t1819,t1820,t1821,t1824,t1825,t1826,t1827,t1828,t1829,t1830,t1831,t1832,t1836,t1837,t1838,t1839,t1841,t1842,t1844,t1845,t1846,t1849,t1851,t1852,t1856,t1857,t1859,t1860,t1862,t1863,t1864,t1865,t1866,t1867,t1870,t1871,t1872,t1873,t1874,t1875,t1877,t1881,t1882,t1883,t1884,t1887,t1888,t1890,t1891,t1893,t1894,t1895,t1896,t1897,t1898,t1899,t1900,t1901,t1903,t1905,t1906,t1907,t1908,t1909,t1910,t1911,t1912,t1913,t1914,t1915,t1916,t1917,t1918,t1919,t1921,t1922,t1924,t1926,t1927,t1928,t1929,t1930,t1931,t1935,t1937,t1938,t1939,t1940,t1941,t1942,t1943,t1944,t195,t1950,t1951,t1952,t1953,t1955,t1956,t1957,t1960,t1961,t1962,t1963,t1964,t1965,t1966,t1968,t1969,t197,t1970,t1971,t1973,t1974,t1975,t1976,t1977,t1979,t1980,t1981,t1982,t1983,t1985,t1986,t1989,t1990,t1994,t1995,t1998,t1999,t2,t2000,t2004,t2005,t2007,t2008,t2015,t2016,t2017,t2020,t2021,t2023,t2024,t2025,t2026,t2028,t2029,t2033,t2035,t2037,t2042,t2043,t2045,t2046,t2047,t2050,t2052,t2053,t2056,t2057,t2058,t2059,t2060,t2061,t2062,t2063,t2064,t2066,t2067,t2068,t2069,t2072,t2075,t2078,t2079,t2081,t2083,t2084,t2087,t2090,t2091,t2094,t2095,t2096,t2097,t2098,t2099,t2100,t2102,t2103,t2104,t2106,t2108,t2116,t2118,t2119,t2120,t2121,t2123,t2127,t213,t2130,t2131,t2134,t2135,t2136,t214,t2140,t2141,t2142,t2144,t2146,t2147,t2148,t2149,t2150,t2151,t2152,t2154,t2155,t2156,t2157,t2158,t2161,t2165,t2167,t2171,t2172,t2174,t2176,t2178,t2179,t2181,t2182,t2183,t2185,t2186,t2187,t2188,t2189,t2190,t2191,t2196,t2201,t2202,t2203,t2205,t2206,t2208,t2209,t2211,t2214,t2215,t2216,t2218,t2220,t2221,t2222,t2223,t2224,t2225,t2227,t2228,t2229,t2231,t2233,t2237,t2238,t2239,t2240,t2242,t2245,t2246,t2247,t2249,t2251,t2252,t2253,t2254,t2255,t2257,t2258,t2259,t2260,t2262,t2263,t2267,t2271,t2273,t2274,t2275,t2281,t2285,t2286,t2287,t2288,t2290,t2293,t2294,t2296,t2297,t2298,t2299,t2303,t2305,t2306,t2307,t2309,t2310,t2312,t2314,t2315,t2316,t2317,t2318,t2320,t2321,t2322,t2323,t2324,t2326,t2327,t2328,t2331,t2334,t2335,t2336,t2339,t2340,t2341,t2342,t2343,t2345,t2346,t2347,t2348,t2349,t2350,t2351,t2353,t2354,t2356,t2357,t2358,t2360,t2362,t2363,t2366,t2369,t2371,t2372,t2375,t2376,t2378,t2380,t2382,t2385,t2386,t2387,t2388,t2389,t2390,t2392,t2397,t2399,t24,t2400,t2401,t2402,t2403,t2404,t2407,t2408,t2409,t2411,t2412,t2417,t2420,t2422,t2423,t2424,t2425,t2426,t2427,t2428,t2429,t2430,t2431,t2432,t2433,t2435,t2436,t2438,t2447,t2455,t2456,t2458,t2460,t2461,t2462,t2463,t2464,t2465,t2466,t2467,t2468,t2469,t2470,t2471,t2472,t2473,t2474,t2476,t2477,t2479,t2480,t2483,t2484,t2485,t2487,t2488,t2489,t2492,t2495,t25,t2502,t2503,t2504,t2505,t2512,t2513,t2514,t2515,t2516,t2518,t2519,t2520,t2525,t2527,t2528,t2529,t2530,t2531,t2532,t2533,t2534,t2535,t2536,t2539,t2540,t2543,t2544,t2545,t2546,t2547,t2550,t2551,t2552,t2560,t2562,t2563,t2564,t2565,t2566,t2567,t2568,t2570,t2576,t2577,t2579,t2581,t2584,t2587,t2588,t2589,t259,t2590,t2591,t2592,t2597,t2598,t2599,t26,t260,t2600,t2605,t2607,t2610,t2611,t2612,t2613,t2614,t2615,t2616,t2617,t2619,t2620,t2621,t2622,t2624,t2627,t2628,t2632,t2634,t2635,t2637,t2638,t2640,t2646,t2647,t2648,t2649,t2654,t2656,t2657,t2658,t2660,t2662,t2663,t2664,t2665,t2668,t2669,t2671,t2673,t2677,t2679,t2680,t2681,t2682,t2683,t2687,t2688,t2689,t2692,t2695,t2696,t2698,t2699,t27,t2700,t2702,t2703,t2704,t2705,t2706,t2707,t2708,t2710,t2711,t2712,t2714,t2715,t2717,t2718,t2722,t2723,t2725,t2730,t2731,t2732,t2735,t2740,t2742,t2743,t2744,t2745,t2746,t2747,t2748,t2749,t2750,t2751,t2752,t2754,t2755,t2756,t2757,t2758,t2759,t276,t2760,t2761,t2762,t2763,t2764,t2765,t2766,t2768,t2769,t277,t2770,t2771,t2774,t2776,t2778,t2781,t2782,t2783,t2784,t2786,t2787,t2788,t2790,t2792,t2797,t2799,t28,t2802,t2803,t2804,t2806,t2807,t2811,t2813,t2816,t2817,t2819,t2821,t2823,t2824,t2825,t2828,t283,t2830,t2832,t2833,t2835,t2836,t2837,t2838,t2839,t284,t2841,t2842,t2843,t2844,t2845,t2846,t2847,t2849,t285,t2855,t2856,t2857,t2859,t286,t2863,t2864,t2865,t2869,t287,t2870,t2871,t2872,t2874,t2875,t2876,t2877,t2878,t2879,t288,t2880,t2883,t2884,t2885,t2886,t2887,t2889,t289,t2890,t2892,t2895,t2896,t290,t2902,t2906,t2907,t2909,t291,t2912,t2913,t2915,t2916,t2917,t2918,t2919,t292,t2920,t2926,t2927,t2928,t2929,t293,t2931,t2932,t2938,t294,t2940,t2944,t2945,t2946,t2949,t2950,t2951,t2952,t2953,t2954,t2955,t2956,t2957,t2959,t2960,t2961,t2962,t2963,t2964,t2966,t2967,t2969,t2975,t2976,t2977,t2978,t2979,t2982,t2983,t2988,t2989,t2991,t2992,t2994,t2995,t3,t30,t3001,t3002,t3003,t3004,t3005,t3006,t3007,t3008,t3009,t3010,t3011,t3012,t3013,t3014,t3015,t3016,t3017,t3019,t3020,t3021,t3022,t3023,t3025,t3028,t3030,t3034,t3035,t3037,t3039,t304,t3047,t3048,t3051,t3053,t3054,t3059,t3060,t3061,t3062,t3063,t3065,t3069,t3070,t3074,t3075,t3077,t3078,t3081,t3083,t3084,t3085,t3089,t3090,t3091,t3092,t3094,t3098,t3100,t3102,t3105,t3106,t3107,t3108,t3109,t3112,t3115,t3117,t3118,t3124,t3125,t3127,t3129,t3130,t3132,t3133,t3134,t3135,t3136,t3138,t3141,t3146,t3148,t3149,t3151,t3153,t3157,t3159,t3160,t3165,t3170,t3171,t3172,t3173,t3174,t3175,t3177,t3180,t3181,t3184,t3186,t3187,t3189,t3199,t3200,t3203,t3204,t3210,t3212,t3218,t3220,t3222,t3224,t3226,t3228,t3233,t3235,t3237,t3238,t3241,t3242,t3243,t3246,t3247,t3248,t3249,t3256,t3260,t3263,t3265,t3266,t3272,t3274,t3277,t3284,t3285,t3286,t3290,t3291,t3294,t33,t3304,t3305,t3317,t3319,t3321,t3322,t3323,t3325,t3330,t3331,t3332,t3337,t3339,t3341,t3351,t3360,t3364,t3370,t3380,t3383,t34,t3403,t3415,t3416,t3417,t3419,t3420,t3426,t3434,t3438,t3441,t3449,t3453,t3457,t3459,t346,t3469,t347,t3471,t3474,t3478,t348,t3483,t3484,t3487,t3495,t3499,t35,t3503,t3504,t3505,t3520,t3521,t3522,t3523,t3524,t3527,t3531,t3539,t3547,t3548,t3551,t3559,t3562,t3565,t3569,t3577,t3580,t3581,t3583,t3595,t3609,t3611,t3617,t3619,t3635,t3639,t3643,t3644,t3657,t3666,t3671,t3672,t3677,t3678,t3680,t3683,t3684,t3699,t3701,t3702,t3704,t3706,t3708,t3709,t3713,t3717,t3721,t3730,t3739,t3743,t3749,t375,t3750,t3752,t376,t3761,t3768,t3769,t377,t3771,t3772,t3787,t3790,t3791,t3792,t38,t381,t3819,t382,t3823,t3828,t383,t3832,t3835,t3842,t3847,t3855,t3858,t3862,t3866,t3873,t3880,t3882,t3883,t390,t3900,t3902,t3906,t3907,t3908,t3909,t3910,t3913,t3915,t3916,t3926,t3928,t3929,t3930,t3931,t3932,t3933,t3936,t3937,t394,t3940,t3942,t3944,t3952,t3955,t3956,t3957,t3959,t3960,t3961,t3962,t3964,t3965,t3967,t3968,t3969,t3971,t3974,t3976,t3981,t3982,t3983,t399,t3993,t3994,t3995,t3996,t3998,t4,t400,t4003,t4004,t4008,t401,t4012,t4014,t4028,t4029,t4033,t4035,t4036,t4038,t4042,t4047,t4048,t4049,t4051,t4052,t4054,t4056,t4058,t4059,t4060,t4061,t4064,t4068,t4070,t4073,t4074,t4078,t4081,t4086,t4087,t4088,t4089,t4090,t4092,t4093,t4098,t41,t410,t411,t412,t4121,t413,t414,t4141,t4142,t4143,t415,t4153,t4161,t4172,t4181,t4182,t4189,t4190,t4197,t420,t421,t4210,t4218,t4234,t4235,t4236,t424,t425,t4256,t4269,t4294,t4295,t4297,t4298,t430,t431,t4323,t433,t434,t4349,t4355,t436,t4363,t44,t445,t4474,t4475,t448,t450,t4509,t451,t456,t459,t4597,t4598,t4599,t46,t4603,t463,t465,t466,t4752,t478,t48,t482,t483,t484,t485,t487,t488,t49,t491,t495,t496,t5,t50,t501,t502,t504,t505,t506,t51,t514,t519,t523,t524,t527,t530,t534,t537,t539,t54,t541,t542,t544,t546,t547,t55,t550,t553,t555,t557,t558,t559,t56,t560,t561,t57,t572,t573,t574,t575,t578,t581,t584,t587,t59,t595,t6,t603,t61,t614,t623,t624,t627,t628,t629,t631,t632,t634,t641,t643,t644,t648,t65,t650,t651,t652,t653,t654,t655,t657,t662,t663,t664,t665,t666,t667,t668,t669,t672,t674,t675,t676,t68,t69,t693,t699,t7,t701,t71,t720,t721,t722,t724,t73,t731,t732,t735,t736,t741,t744,t746,t749,t750,t751,t752,t753,t754,t755,t756,t757,t759,t760,t761,t762,t764,t765,t768,t769,t772,t774,t776,t778,t779,t792,t794,t795,t797,t799,t8,t801,t802,t803,t805,t806,t811,t817,t818,t819,t820,t821,t822,t823,t824,t826,t828,t830,t831,t834,t835,t836,t837,t838,t839,t841,t842,t843,t844,t845,t846,t847,t848,t850,t851,t852,t853,t854,t855,t858,t859,t862,t863,t864,t865,t867,t868,t869,t870,t871,t872,t873,t874,t875,t876,t877,t879,t881,t882,t884,t885,t886,t887,t888,t889,t890,t891,t892,t893,t894,t895,t896,t897,t898,t9,t900,t901,t902,t903,t904,t906,t907,t908,t909,t910,t912,t913,t914,t915,t916,t917,t918,t919,t923,t924,t925,t926,t927,t928,t933,t934,t941,t947,t948,t949,t950,t951,t952,t953,t954,t955,t957,t964,t965,t966,t968,t970,t972,t974,t976,t977,t979,t980,t983,t985,t986,t987,t990,t991,t992,t993,t994,t995,t996});
end
function C = ft_6(ct)
B_cg_H = ct{1};
ITail = ct{2};
Mb = ct{3};
Mm = ct{4};
Mt = ct{5};
T_cg_H = ct{6};
dphi1 = ct{7};
dphi2 = ct{8};
dpsi1 = ct{9};
dth1 = ct{10};
dth2 = ct{11};
dx = ct{12};
dy = ct{13};
dz = ct{14};
t10 = ct{15};
t1003 = ct{16};
t1004 = ct{17};
t1005 = ct{18};
t1006 = ct{19};
t1007 = ct{20};
t1008 = ct{21};
t1009 = ct{22};
t1010 = ct{23};
t1011 = ct{24};
t1012 = ct{25};
t1013 = ct{26};
t1014 = ct{27};
t1015 = ct{28};
t1016 = ct{29};
t1017 = ct{30};
t1018 = ct{31};
t1019 = ct{32};
t1020 = ct{33};
t1021 = ct{34};
t1023 = ct{35};
t1024 = ct{36};
t1025 = ct{37};
t1026 = ct{38};
t1029 = ct{39};
t103 = ct{40};
t1030 = ct{41};
t1031 = ct{42};
t1036 = ct{43};
t1037 = ct{44};
t1041 = ct{45};
t1042 = ct{46};
t1043 = ct{47};
t1044 = ct{48};
t1045 = ct{49};
t1046 = ct{50};
t1047 = ct{51};
t1049 = ct{52};
t105 = ct{53};
t1050 = ct{54};
t1051 = ct{55};
t1052 = ct{56};
t1053 = ct{57};
t1054 = ct{58};
t1055 = ct{59};
t1056 = ct{60};
t1057 = ct{61};
t1058 = ct{62};
t1059 = ct{63};
t1060 = ct{64};
t1061 = ct{65};
t1062 = ct{66};
t1063 = ct{67};
t1064 = ct{68};
t1065 = ct{69};
t1067 = ct{70};
t1068 = ct{71};
t1071 = ct{72};
t1072 = ct{73};
t1073 = ct{74};
t1074 = ct{75};
t1075 = ct{76};
t1076 = ct{77};
t1077 = ct{78};
t1078 = ct{79};
t1079 = ct{80};
t1080 = ct{81};
t1081 = ct{82};
t1082 = ct{83};
t1084 = ct{84};
t1085 = ct{85};
t1086 = ct{86};
t1088 = ct{87};
t1093 = ct{88};
t1097 = ct{89};
t11 = ct{90};
t1102 = ct{91};
t1105 = ct{92};
t1108 = ct{93};
t1109 = ct{94};
t1113 = ct{95};
t1114 = ct{96};
t1115 = ct{97};
t1116 = ct{98};
t1117 = ct{99};
t1118 = ct{100};
t1119 = ct{101};
t1120 = ct{102};
t1121 = ct{103};
t1122 = ct{104};
t1123 = ct{105};
t1124 = ct{106};
t1125 = ct{107};
t1126 = ct{108};
t1127 = ct{109};
t1128 = ct{110};
t1129 = ct{111};
t1130 = ct{112};
t1131 = ct{113};
t1132 = ct{114};
t1133 = ct{115};
t1134 = ct{116};
t1135 = ct{117};
t1136 = ct{118};
t1137 = ct{119};
t1138 = ct{120};
t1139 = ct{121};
t1140 = ct{122};
t1141 = ct{123};
t1142 = ct{124};
t1143 = ct{125};
t1144 = ct{126};
t1145 = ct{127};
t1146 = ct{128};
t1147 = ct{129};
t1148 = ct{130};
t1149 = ct{131};
t1150 = ct{132};
t1152 = ct{133};
t1153 = ct{134};
t1154 = ct{135};
t1155 = ct{136};
t1156 = ct{137};
t1157 = ct{138};
t1158 = ct{139};
t1159 = ct{140};
t1160 = ct{141};
t1161 = ct{142};
t1162 = ct{143};
t1163 = ct{144};
t1164 = ct{145};
t1165 = ct{146};
t1166 = ct{147};
t1167 = ct{148};
t1168 = ct{149};
t1169 = ct{150};
t1170 = ct{151};
t1171 = ct{152};
t1172 = ct{153};
t1173 = ct{154};
t1174 = ct{155};
t1176 = ct{156};
t1177 = ct{157};
t1178 = ct{158};
t1179 = ct{159};
t1181 = ct{160};
t1182 = ct{161};
t1183 = ct{162};
t1184 = ct{163};
t1185 = ct{164};
t1186 = ct{165};
t1187 = ct{166};
t1188 = ct{167};
t1189 = ct{168};
t1190 = ct{169};
t1191 = ct{170};
t1192 = ct{171};
t1193 = ct{172};
t1194 = ct{173};
t1195 = ct{174};
t1196 = ct{175};
t1197 = ct{176};
t1199 = ct{177};
t120 = ct{178};
t1200 = ct{179};
t1201 = ct{180};
t1202 = ct{181};
t1203 = ct{182};
t1205 = ct{183};
t1206 = ct{184};
t1207 = ct{185};
t1209 = ct{186};
t1211 = ct{187};
t1212 = ct{188};
t1213 = ct{189};
t1214 = ct{190};
t1215 = ct{191};
t1216 = ct{192};
t1218 = ct{193};
t1221 = ct{194};
t1223 = ct{195};
t1224 = ct{196};
t1225 = ct{197};
t1226 = ct{198};
t1227 = ct{199};
t1228 = ct{200};
t1229 = ct{201};
t123 = ct{202};
t1230 = ct{203};
t1231 = ct{204};
t1232 = ct{205};
t1234 = ct{206};
t1235 = ct{207};
t1236 = ct{208};
t1237 = ct{209};
t1238 = ct{210};
t1240 = ct{211};
t1242 = ct{212};
t1243 = ct{213};
t1244 = ct{214};
t1245 = ct{215};
t1246 = ct{216};
t1247 = ct{217};
t1248 = ct{218};
t1250 = ct{219};
t1251 = ct{220};
t1252 = ct{221};
t1253 = ct{222};
t1255 = ct{223};
t1256 = ct{224};
t1257 = ct{225};
t1260 = ct{226};
t1261 = ct{227};
t1262 = ct{228};
t1263 = ct{229};
t1264 = ct{230};
t1265 = ct{231};
t1266 = ct{232};
t1268 = ct{233};
t1270 = ct{234};
t1272 = ct{235};
t1275 = ct{236};
t1279 = ct{237};
t1280 = ct{238};
t1282 = ct{239};
t1283 = ct{240};
t1284 = ct{241};
t1285 = ct{242};
t1287 = ct{243};
t1289 = ct{244};
t1296 = ct{245};
t130 = ct{246};
t1301 = ct{247};
t1302 = ct{248};
t1303 = ct{249};
t1304 = ct{250};
t1305 = ct{251};
t1306 = ct{252};
t1307 = ct{253};
t1308 = ct{254};
t1309 = ct{255};
t1311 = ct{256};
t1312 = ct{257};
t1313 = ct{258};
t1319 = ct{259};
t1320 = ct{260};
t1322 = ct{261};
t1323 = ct{262};
t1324 = ct{263};
t1325 = ct{264};
t1328 = ct{265};
t1329 = ct{266};
t1331 = ct{267};
t1332 = ct{268};
t1334 = ct{269};
t1335 = ct{270};
t1337 = ct{271};
t1338 = ct{272};
t134 = ct{273};
t1340 = ct{274};
t1341 = ct{275};
t1342 = ct{276};
t1343 = ct{277};
t1344 = ct{278};
t1345 = ct{279};
t1348 = ct{280};
t1349 = ct{281};
t1352 = ct{282};
t1354 = ct{283};
t1355 = ct{284};
t1356 = ct{285};
t1357 = ct{286};
t1358 = ct{287};
t1360 = ct{288};
t1361 = ct{289};
t1362 = ct{290};
t1363 = ct{291};
t1365 = ct{292};
t1366 = ct{293};
t1367 = ct{294};
t1368 = ct{295};
t1370 = ct{296};
t1371 = ct{297};
t1372 = ct{298};
t1373 = ct{299};
t1374 = ct{300};
t1377 = ct{301};
t1378 = ct{302};
t1379 = ct{303};
t1380 = ct{304};
t1381 = ct{305};
t1382 = ct{306};
t1383 = ct{307};
t1384 = ct{308};
t1385 = ct{309};
t1386 = ct{310};
t1388 = ct{311};
t1389 = ct{312};
t1391 = ct{313};
t1393 = ct{314};
t1394 = ct{315};
t1395 = ct{316};
t1396 = ct{317};
t1397 = ct{318};
t1399 = ct{319};
t1400 = ct{320};
t1402 = ct{321};
t1403 = ct{322};
t1405 = ct{323};
t1406 = ct{324};
t1407 = ct{325};
t1408 = ct{326};
t1409 = ct{327};
t1410 = ct{328};
t1412 = ct{329};
t1413 = ct{330};
t1414 = ct{331};
t1415 = ct{332};
t1416 = ct{333};
t1418 = ct{334};
t1419 = ct{335};
t1421 = ct{336};
t1422 = ct{337};
t1424 = ct{338};
t1426 = ct{339};
t1427 = ct{340};
t1429 = ct{341};
t1430 = ct{342};
t1431 = ct{343};
t1432 = ct{344};
t1433 = ct{345};
t1434 = ct{346};
t1435 = ct{347};
t1437 = ct{348};
t1438 = ct{349};
t1439 = ct{350};
t144 = ct{351};
t1440 = ct{352};
t1441 = ct{353};
t1442 = ct{354};
t1443 = ct{355};
t1444 = ct{356};
t1445 = ct{357};
t1446 = ct{358};
t1447 = ct{359};
t1448 = ct{360};
t1450 = ct{361};
t1451 = ct{362};
t1453 = ct{363};
t1454 = ct{364};
t1455 = ct{365};
t1456 = ct{366};
t1457 = ct{367};
t1458 = ct{368};
t1459 = ct{369};
t1460 = ct{370};
t1461 = ct{371};
t1462 = ct{372};
t1463 = ct{373};
t1465 = ct{374};
t1466 = ct{375};
t1467 = ct{376};
t1468 = ct{377};
t1469 = ct{378};
t1470 = ct{379};
t1471 = ct{380};
t1472 = ct{381};
t1475 = ct{382};
t1476 = ct{383};
t1477 = ct{384};
t1478 = ct{385};
t1479 = ct{386};
t1481 = ct{387};
t1482 = ct{388};
t1483 = ct{389};
t1484 = ct{390};
t1486 = ct{391};
t1487 = ct{392};
t1488 = ct{393};
t1489 = ct{394};
t1491 = ct{395};
t1492 = ct{396};
t1493 = ct{397};
t1494 = ct{398};
t1495 = ct{399};
t1496 = ct{400};
t1497 = ct{401};
t1498 = ct{402};
t15 = ct{403};
t1500 = ct{404};
t1501 = ct{405};
t1503 = ct{406};
t1504 = ct{407};
t1505 = ct{408};
t1506 = ct{409};
t1507 = ct{410};
t1508 = ct{411};
t1509 = ct{412};
t1511 = ct{413};
t1512 = ct{414};
t1513 = ct{415};
t1514 = ct{416};
t1515 = ct{417};
t1516 = ct{418};
t1517 = ct{419};
t1518 = ct{420};
t1520 = ct{421};
t1521 = ct{422};
t1522 = ct{423};
t1523 = ct{424};
t1524 = ct{425};
t1525 = ct{426};
t1526 = ct{427};
t1527 = ct{428};
t1528 = ct{429};
t1529 = ct{430};
t1531 = ct{431};
t1532 = ct{432};
t1533 = ct{433};
t1534 = ct{434};
t1535 = ct{435};
t1536 = ct{436};
t1537 = ct{437};
t1539 = ct{438};
t1540 = ct{439};
t1541 = ct{440};
t1542 = ct{441};
t1543 = ct{442};
t1547 = ct{443};
t1548 = ct{444};
t1549 = ct{445};
t1550 = ct{446};
t1552 = ct{447};
t1553 = ct{448};
t1555 = ct{449};
t1557 = ct{450};
t1559 = ct{451};
t1560 = ct{452};
t1561 = ct{453};
t1562 = ct{454};
t1563 = ct{455};
t1565 = ct{456};
t1566 = ct{457};
t1567 = ct{458};
t1568 = ct{459};
t1572 = ct{460};
t1573 = ct{461};
t1576 = ct{462};
t1577 = ct{463};
t1580 = ct{464};
t1581 = ct{465};
t1582 = ct{466};
t1585 = ct{467};
t1587 = ct{468};
t1588 = ct{469};
t1589 = ct{470};
t1591 = ct{471};
t1592 = ct{472};
t1593 = ct{473};
t1594 = ct{474};
t1595 = ct{475};
t1596 = ct{476};
t1597 = ct{477};
t1598 = ct{478};
t1599 = ct{479};
t160 = ct{480};
t1600 = ct{481};
t1601 = ct{482};
t1602 = ct{483};
t1603 = ct{484};
t1605 = ct{485};
t1606 = ct{486};
t1609 = ct{487};
t161 = ct{488};
t1610 = ct{489};
t1613 = ct{490};
t1614 = ct{491};
t1615 = ct{492};
t1616 = ct{493};
t1617 = ct{494};
t1618 = ct{495};
t1619 = ct{496};
t162 = ct{497};
t1620 = ct{498};
t1621 = ct{499};
t1624 = ct{500};
t1627 = ct{501};
t1628 = ct{502};
t1632 = ct{503};
t1635 = ct{504};
t1636 = ct{505};
t1637 = ct{506};
t1639 = ct{507};
t1640 = ct{508};
t1641 = ct{509};
t1642 = ct{510};
t1644 = ct{511};
t1645 = ct{512};
t1646 = ct{513};
t1647 = ct{514};
t1648 = ct{515};
t1649 = ct{516};
t1651 = ct{517};
t1652 = ct{518};
t1653 = ct{519};
t1654 = ct{520};
t1655 = ct{521};
t1656 = ct{522};
t1657 = ct{523};
t1658 = ct{524};
t1659 = ct{525};
t1660 = ct{526};
t1661 = ct{527};
t1663 = ct{528};
t1664 = ct{529};
t1665 = ct{530};
t1667 = ct{531};
t1668 = ct{532};
t1669 = ct{533};
t1670 = ct{534};
t1671 = ct{535};
t1672 = ct{536};
t1673 = ct{537};
t1674 = ct{538};
t1675 = ct{539};
t1676 = ct{540};
t1677 = ct{541};
t1678 = ct{542};
t1679 = ct{543};
t1680 = ct{544};
t1681 = ct{545};
t1682 = ct{546};
t1683 = ct{547};
t1684 = ct{548};
t1685 = ct{549};
t1686 = ct{550};
t1687 = ct{551};
t1688 = ct{552};
t1689 = ct{553};
t1690 = ct{554};
t1691 = ct{555};
t1692 = ct{556};
t1693 = ct{557};
t1694 = ct{558};
t1695 = ct{559};
t1698 = ct{560};
t1699 = ct{561};
t1700 = ct{562};
t1701 = ct{563};
t1702 = ct{564};
t1703 = ct{565};
t1704 = ct{566};
t1705 = ct{567};
t1706 = ct{568};
t1707 = ct{569};
t1709 = ct{570};
t1711 = ct{571};
t1712 = ct{572};
t1715 = ct{573};
t1716 = ct{574};
t1718 = ct{575};
t1719 = ct{576};
t1721 = ct{577};
t1723 = ct{578};
t1725 = ct{579};
t1726 = ct{580};
t1727 = ct{581};
t1729 = ct{582};
t1730 = ct{583};
t1731 = ct{584};
t1732 = ct{585};
t1733 = ct{586};
t1734 = ct{587};
t1735 = ct{588};
t1736 = ct{589};
t1737 = ct{590};
t1741 = ct{591};
t1742 = ct{592};
t1743 = ct{593};
t1744 = ct{594};
t1745 = ct{595};
t1746 = ct{596};
t1747 = ct{597};
t1748 = ct{598};
t1749 = ct{599};
t1750 = ct{600};
t1751 = ct{601};
t1753 = ct{602};
t1756 = ct{603};
t1758 = ct{604};
t1759 = ct{605};
t1760 = ct{606};
t1761 = ct{607};
t1762 = ct{608};
t1764 = ct{609};
t1765 = ct{610};
t1767 = ct{611};
t1768 = ct{612};
t1769 = ct{613};
t1770 = ct{614};
t1772 = ct{615};
t1773 = ct{616};
t1774 = ct{617};
t1775 = ct{618};
t1776 = ct{619};
t1777 = ct{620};
t1783 = ct{621};
t1784 = ct{622};
t1785 = ct{623};
t1786 = ct{624};
t1788 = ct{625};
t1789 = ct{626};
t1790 = ct{627};
t1791 = ct{628};
t1793 = ct{629};
t1794 = ct{630};
t1795 = ct{631};
t1796 = ct{632};
t1797 = ct{633};
t1798 = ct{634};
t1799 = ct{635};
t1801 = ct{636};
t1802 = ct{637};
t1803 = ct{638};
t1805 = ct{639};
t1806 = ct{640};
t1808 = ct{641};
t1810 = ct{642};
t1811 = ct{643};
t1812 = ct{644};
t1813 = ct{645};
t1814 = ct{646};
t1815 = ct{647};
t1816 = ct{648};
t1817 = ct{649};
t1819 = ct{650};
t1820 = ct{651};
t1821 = ct{652};
t1824 = ct{653};
t1825 = ct{654};
t1826 = ct{655};
t1827 = ct{656};
t1828 = ct{657};
t1829 = ct{658};
t1830 = ct{659};
t1831 = ct{660};
t1832 = ct{661};
t1836 = ct{662};
t1837 = ct{663};
t1838 = ct{664};
t1839 = ct{665};
t1841 = ct{666};
t1842 = ct{667};
t1844 = ct{668};
t1845 = ct{669};
t1846 = ct{670};
t1849 = ct{671};
t1851 = ct{672};
t1852 = ct{673};
t1856 = ct{674};
t1857 = ct{675};
t1859 = ct{676};
t1860 = ct{677};
t1862 = ct{678};
t1863 = ct{679};
t1864 = ct{680};
t1865 = ct{681};
t1866 = ct{682};
t1867 = ct{683};
t1870 = ct{684};
t1871 = ct{685};
t1872 = ct{686};
t1873 = ct{687};
t1874 = ct{688};
t1875 = ct{689};
t1877 = ct{690};
t1881 = ct{691};
t1882 = ct{692};
t1883 = ct{693};
t1884 = ct{694};
t1887 = ct{695};
t1888 = ct{696};
t1890 = ct{697};
t1891 = ct{698};
t1893 = ct{699};
t1894 = ct{700};
t1895 = ct{701};
t1896 = ct{702};
t1897 = ct{703};
t1898 = ct{704};
t1899 = ct{705};
t1900 = ct{706};
t1901 = ct{707};
t1903 = ct{708};
t1905 = ct{709};
t1906 = ct{710};
t1907 = ct{711};
t1908 = ct{712};
t1909 = ct{713};
t1910 = ct{714};
t1911 = ct{715};
t1912 = ct{716};
t1913 = ct{717};
t1914 = ct{718};
t1915 = ct{719};
t1916 = ct{720};
t1917 = ct{721};
t1918 = ct{722};
t1919 = ct{723};
t1921 = ct{724};
t1922 = ct{725};
t1924 = ct{726};
t1926 = ct{727};
t1927 = ct{728};
t1928 = ct{729};
t1929 = ct{730};
t1930 = ct{731};
t1931 = ct{732};
t1935 = ct{733};
t1937 = ct{734};
t1938 = ct{735};
t1939 = ct{736};
t1940 = ct{737};
t1941 = ct{738};
t1942 = ct{739};
t1943 = ct{740};
t1944 = ct{741};
t195 = ct{742};
t1950 = ct{743};
t1951 = ct{744};
t1952 = ct{745};
t1953 = ct{746};
t1955 = ct{747};
t1956 = ct{748};
t1957 = ct{749};
t1960 = ct{750};
t1961 = ct{751};
t1962 = ct{752};
t1963 = ct{753};
t1964 = ct{754};
t1965 = ct{755};
t1966 = ct{756};
t1968 = ct{757};
t1969 = ct{758};
t197 = ct{759};
t1970 = ct{760};
t1971 = ct{761};
t1973 = ct{762};
t1974 = ct{763};
t1975 = ct{764};
t1976 = ct{765};
t1977 = ct{766};
t1979 = ct{767};
t1980 = ct{768};
t1981 = ct{769};
t1982 = ct{770};
t1983 = ct{771};
t1985 = ct{772};
t1986 = ct{773};
t1989 = ct{774};
t1990 = ct{775};
t1994 = ct{776};
t1995 = ct{777};
t1998 = ct{778};
t1999 = ct{779};
t2 = ct{780};
t2000 = ct{781};
t2004 = ct{782};
t2005 = ct{783};
t2007 = ct{784};
t2008 = ct{785};
t2015 = ct{786};
t2016 = ct{787};
t2017 = ct{788};
t2020 = ct{789};
t2021 = ct{790};
t2023 = ct{791};
t2024 = ct{792};
t2025 = ct{793};
t2026 = ct{794};
t2028 = ct{795};
t2029 = ct{796};
t2033 = ct{797};
t2035 = ct{798};
t2037 = ct{799};
t2042 = ct{800};
t2043 = ct{801};
t2045 = ct{802};
t2046 = ct{803};
t2047 = ct{804};
t2050 = ct{805};
t2052 = ct{806};
t2053 = ct{807};
t2056 = ct{808};
t2057 = ct{809};
t2058 = ct{810};
t2059 = ct{811};
t2060 = ct{812};
t2061 = ct{813};
t2062 = ct{814};
t2063 = ct{815};
t2064 = ct{816};
t2066 = ct{817};
t2067 = ct{818};
t2068 = ct{819};
t2069 = ct{820};
t2072 = ct{821};
t2075 = ct{822};
t2078 = ct{823};
t2079 = ct{824};
t2081 = ct{825};
t2083 = ct{826};
t2084 = ct{827};
t2087 = ct{828};
t2090 = ct{829};
t2091 = ct{830};
t2094 = ct{831};
t2095 = ct{832};
t2096 = ct{833};
t2097 = ct{834};
t2098 = ct{835};
t2099 = ct{836};
t2100 = ct{837};
t2102 = ct{838};
t2103 = ct{839};
t2104 = ct{840};
t2106 = ct{841};
t2108 = ct{842};
t2116 = ct{843};
t2118 = ct{844};
t2119 = ct{845};
t2120 = ct{846};
t2121 = ct{847};
t2123 = ct{848};
t2127 = ct{849};
t213 = ct{850};
t2130 = ct{851};
t2131 = ct{852};
t2134 = ct{853};
t2135 = ct{854};
t2136 = ct{855};
t214 = ct{856};
t2140 = ct{857};
t2141 = ct{858};
t2142 = ct{859};
t2144 = ct{860};
t2146 = ct{861};
t2147 = ct{862};
t2148 = ct{863};
t2149 = ct{864};
t2150 = ct{865};
t2151 = ct{866};
t2152 = ct{867};
t2154 = ct{868};
t2155 = ct{869};
t2156 = ct{870};
t2157 = ct{871};
t2158 = ct{872};
t2161 = ct{873};
t2165 = ct{874};
t2167 = ct{875};
t2171 = ct{876};
t2172 = ct{877};
t2174 = ct{878};
t2176 = ct{879};
t2178 = ct{880};
t2179 = ct{881};
t2181 = ct{882};
t2182 = ct{883};
t2183 = ct{884};
t2185 = ct{885};
t2186 = ct{886};
t2187 = ct{887};
t2188 = ct{888};
t2189 = ct{889};
t2190 = ct{890};
t2191 = ct{891};
t2196 = ct{892};
t2201 = ct{893};
t2202 = ct{894};
t2203 = ct{895};
t2205 = ct{896};
t2206 = ct{897};
t2208 = ct{898};
t2209 = ct{899};
t2211 = ct{900};
t2214 = ct{901};
t2215 = ct{902};
t2216 = ct{903};
t2218 = ct{904};
t2220 = ct{905};
t2221 = ct{906};
t2222 = ct{907};
t2223 = ct{908};
t2224 = ct{909};
t2225 = ct{910};
t2227 = ct{911};
t2228 = ct{912};
t2229 = ct{913};
t2231 = ct{914};
t2233 = ct{915};
t2237 = ct{916};
t2238 = ct{917};
t2239 = ct{918};
t2240 = ct{919};
t2242 = ct{920};
t2245 = ct{921};
t2246 = ct{922};
t2247 = ct{923};
t2249 = ct{924};
t2251 = ct{925};
t2252 = ct{926};
t2253 = ct{927};
t2254 = ct{928};
t2255 = ct{929};
t2257 = ct{930};
t2258 = ct{931};
t2259 = ct{932};
t2260 = ct{933};
t2262 = ct{934};
t2263 = ct{935};
t2267 = ct{936};
t2271 = ct{937};
t2273 = ct{938};
t2274 = ct{939};
t2275 = ct{940};
t2281 = ct{941};
t2285 = ct{942};
t2286 = ct{943};
t2287 = ct{944};
t2288 = ct{945};
t2290 = ct{946};
t2293 = ct{947};
t2294 = ct{948};
t2296 = ct{949};
t2297 = ct{950};
t2298 = ct{951};
t2299 = ct{952};
t2303 = ct{953};
t2305 = ct{954};
t2306 = ct{955};
t2307 = ct{956};
t2309 = ct{957};
t2310 = ct{958};
t2312 = ct{959};
t2314 = ct{960};
t2315 = ct{961};
t2316 = ct{962};
t2317 = ct{963};
t2318 = ct{964};
t2320 = ct{965};
t2321 = ct{966};
t2322 = ct{967};
t2323 = ct{968};
t2324 = ct{969};
t2326 = ct{970};
t2327 = ct{971};
t2328 = ct{972};
t2331 = ct{973};
t2334 = ct{974};
t2335 = ct{975};
t2336 = ct{976};
t2339 = ct{977};
t2340 = ct{978};
t2341 = ct{979};
t2342 = ct{980};
t2343 = ct{981};
t2345 = ct{982};
t2346 = ct{983};
t2347 = ct{984};
t2348 = ct{985};
t2349 = ct{986};
t2350 = ct{987};
t2351 = ct{988};
t2353 = ct{989};
t2354 = ct{990};
t2356 = ct{991};
t2357 = ct{992};
t2358 = ct{993};
t2360 = ct{994};
t2362 = ct{995};
t2363 = ct{996};
t2366 = ct{997};
t2369 = ct{998};
t2371 = ct{999};
t2372 = ct{1000};
t2375 = ct{1001};
t2376 = ct{1002};
t2378 = ct{1003};
t2380 = ct{1004};
t2382 = ct{1005};
t2385 = ct{1006};
t2386 = ct{1007};
t2387 = ct{1008};
t2388 = ct{1009};
t2389 = ct{1010};
t2390 = ct{1011};
t2392 = ct{1012};
t2397 = ct{1013};
t2399 = ct{1014};
t24 = ct{1015};
t2400 = ct{1016};
t2401 = ct{1017};
t2402 = ct{1018};
t2403 = ct{1019};
t2404 = ct{1020};
t2407 = ct{1021};
t2408 = ct{1022};
t2409 = ct{1023};
t2411 = ct{1024};
t2412 = ct{1025};
t2417 = ct{1026};
t2420 = ct{1027};
t2422 = ct{1028};
t2423 = ct{1029};
t2424 = ct{1030};
t2425 = ct{1031};
t2426 = ct{1032};
t2427 = ct{1033};
t2428 = ct{1034};
t2429 = ct{1035};
t2430 = ct{1036};
t2431 = ct{1037};
t2432 = ct{1038};
t2433 = ct{1039};
t2435 = ct{1040};
t2436 = ct{1041};
t2438 = ct{1042};
t2447 = ct{1043};
t2455 = ct{1044};
t2456 = ct{1045};
t2458 = ct{1046};
t2460 = ct{1047};
t2461 = ct{1048};
t2462 = ct{1049};
t2463 = ct{1050};
t2464 = ct{1051};
t2465 = ct{1052};
t2466 = ct{1053};
t2467 = ct{1054};
t2468 = ct{1055};
t2469 = ct{1056};
t2470 = ct{1057};
t2471 = ct{1058};
t2472 = ct{1059};
t2473 = ct{1060};
t2474 = ct{1061};
t2476 = ct{1062};
t2477 = ct{1063};
t2479 = ct{1064};
t2480 = ct{1065};
t2483 = ct{1066};
t2484 = ct{1067};
t2485 = ct{1068};
t2487 = ct{1069};
t2488 = ct{1070};
t2489 = ct{1071};
t2492 = ct{1072};
t2495 = ct{1073};
t25 = ct{1074};
t2502 = ct{1075};
t2503 = ct{1076};
t2504 = ct{1077};
t2505 = ct{1078};
t2512 = ct{1079};
t2513 = ct{1080};
t2514 = ct{1081};
t2515 = ct{1082};
t2516 = ct{1083};
t2518 = ct{1084};
t2519 = ct{1085};
t2520 = ct{1086};
t2525 = ct{1087};
t2527 = ct{1088};
t2528 = ct{1089};
t2529 = ct{1090};
t2530 = ct{1091};
t2531 = ct{1092};
t2532 = ct{1093};
t2533 = ct{1094};
t2534 = ct{1095};
t2535 = ct{1096};
t2536 = ct{1097};
t2539 = ct{1098};
t2540 = ct{1099};
t2543 = ct{1100};
t2544 = ct{1101};
t2545 = ct{1102};
t2546 = ct{1103};
t2547 = ct{1104};
t2550 = ct{1105};
t2551 = ct{1106};
t2552 = ct{1107};
t2560 = ct{1108};
t2562 = ct{1109};
t2563 = ct{1110};
t2564 = ct{1111};
t2565 = ct{1112};
t2566 = ct{1113};
t2567 = ct{1114};
t2568 = ct{1115};
t2570 = ct{1116};
t2576 = ct{1117};
t2577 = ct{1118};
t2579 = ct{1119};
t2581 = ct{1120};
t2584 = ct{1121};
t2587 = ct{1122};
t2588 = ct{1123};
t2589 = ct{1124};
t259 = ct{1125};
t2590 = ct{1126};
t2591 = ct{1127};
t2592 = ct{1128};
t2597 = ct{1129};
t2598 = ct{1130};
t2599 = ct{1131};
t26 = ct{1132};
t260 = ct{1133};
t2600 = ct{1134};
t2605 = ct{1135};
t2607 = ct{1136};
t2610 = ct{1137};
t2611 = ct{1138};
t2612 = ct{1139};
t2613 = ct{1140};
t2614 = ct{1141};
t2615 = ct{1142};
t2616 = ct{1143};
t2617 = ct{1144};
t2619 = ct{1145};
t2620 = ct{1146};
t2621 = ct{1147};
t2622 = ct{1148};
t2624 = ct{1149};
t2627 = ct{1150};
t2628 = ct{1151};
t2632 = ct{1152};
t2634 = ct{1153};
t2635 = ct{1154};
t2637 = ct{1155};
t2638 = ct{1156};
t2640 = ct{1157};
t2646 = ct{1158};
t2647 = ct{1159};
t2648 = ct{1160};
t2649 = ct{1161};
t2654 = ct{1162};
t2656 = ct{1163};
t2657 = ct{1164};
t2658 = ct{1165};
t2660 = ct{1166};
t2662 = ct{1167};
t2663 = ct{1168};
t2664 = ct{1169};
t2665 = ct{1170};
t2668 = ct{1171};
t2669 = ct{1172};
t2671 = ct{1173};
t2673 = ct{1174};
t2677 = ct{1175};
t2679 = ct{1176};
t2680 = ct{1177};
t2681 = ct{1178};
t2682 = ct{1179};
t2683 = ct{1180};
t2687 = ct{1181};
t2688 = ct{1182};
t2689 = ct{1183};
t2692 = ct{1184};
t2695 = ct{1185};
t2696 = ct{1186};
t2698 = ct{1187};
t2699 = ct{1188};
t27 = ct{1189};
t2700 = ct{1190};
t2702 = ct{1191};
t2703 = ct{1192};
t2704 = ct{1193};
t2705 = ct{1194};
t2706 = ct{1195};
t2707 = ct{1196};
t2708 = ct{1197};
t2710 = ct{1198};
t2711 = ct{1199};
t2712 = ct{1200};
t2714 = ct{1201};
t2715 = ct{1202};
t2717 = ct{1203};
t2718 = ct{1204};
t2722 = ct{1205};
t2723 = ct{1206};
t2725 = ct{1207};
t2730 = ct{1208};
t2731 = ct{1209};
t2732 = ct{1210};
t2735 = ct{1211};
t2740 = ct{1212};
t2742 = ct{1213};
t2743 = ct{1214};
t2744 = ct{1215};
t2745 = ct{1216};
t2746 = ct{1217};
t2747 = ct{1218};
t2748 = ct{1219};
t2749 = ct{1220};
t2750 = ct{1221};
t2751 = ct{1222};
t2752 = ct{1223};
t2754 = ct{1224};
t2755 = ct{1225};
t2756 = ct{1226};
t2757 = ct{1227};
t2758 = ct{1228};
t2759 = ct{1229};
t276 = ct{1230};
t2760 = ct{1231};
t2761 = ct{1232};
t2762 = ct{1233};
t2763 = ct{1234};
t2764 = ct{1235};
t2765 = ct{1236};
t2766 = ct{1237};
t2768 = ct{1238};
t2769 = ct{1239};
t277 = ct{1240};
t2770 = ct{1241};
t2771 = ct{1242};
t2774 = ct{1243};
t2776 = ct{1244};
t2778 = ct{1245};
t2781 = ct{1246};
t2782 = ct{1247};
t2783 = ct{1248};
t2784 = ct{1249};
t2786 = ct{1250};
t2787 = ct{1251};
t2788 = ct{1252};
t2790 = ct{1253};
t2792 = ct{1254};
t2797 = ct{1255};
t2799 = ct{1256};
t28 = ct{1257};
t2802 = ct{1258};
t2803 = ct{1259};
t2804 = ct{1260};
t2806 = ct{1261};
t2807 = ct{1262};
t2811 = ct{1263};
t2813 = ct{1264};
t2816 = ct{1265};
t2817 = ct{1266};
t2819 = ct{1267};
t2821 = ct{1268};
t2823 = ct{1269};
t2824 = ct{1270};
t2825 = ct{1271};
t2828 = ct{1272};
t283 = ct{1273};
t2830 = ct{1274};
t2832 = ct{1275};
t2833 = ct{1276};
t2835 = ct{1277};
t2836 = ct{1278};
t2837 = ct{1279};
t2838 = ct{1280};
t2839 = ct{1281};
t284 = ct{1282};
t2841 = ct{1283};
t2842 = ct{1284};
t2843 = ct{1285};
t2844 = ct{1286};
t2845 = ct{1287};
t2846 = ct{1288};
t2847 = ct{1289};
t2849 = ct{1290};
t285 = ct{1291};
t2855 = ct{1292};
t2856 = ct{1293};
t2857 = ct{1294};
t2859 = ct{1295};
t286 = ct{1296};
t2863 = ct{1297};
t2864 = ct{1298};
t2865 = ct{1299};
t2869 = ct{1300};
t287 = ct{1301};
t2870 = ct{1302};
t2871 = ct{1303};
t2872 = ct{1304};
t2874 = ct{1305};
t2875 = ct{1306};
t2876 = ct{1307};
t2877 = ct{1308};
t2878 = ct{1309};
t2879 = ct{1310};
t288 = ct{1311};
t2880 = ct{1312};
t2883 = ct{1313};
t2884 = ct{1314};
t2885 = ct{1315};
t2886 = ct{1316};
t2887 = ct{1317};
t2889 = ct{1318};
t289 = ct{1319};
t2890 = ct{1320};
t2892 = ct{1321};
t2895 = ct{1322};
t2896 = ct{1323};
t290 = ct{1324};
t2902 = ct{1325};
t2906 = ct{1326};
t2907 = ct{1327};
t2909 = ct{1328};
t291 = ct{1329};
t2912 = ct{1330};
t2913 = ct{1331};
t2915 = ct{1332};
t2916 = ct{1333};
t2917 = ct{1334};
t2918 = ct{1335};
t2919 = ct{1336};
t292 = ct{1337};
t2920 = ct{1338};
t2926 = ct{1339};
t2927 = ct{1340};
t2928 = ct{1341};
t2929 = ct{1342};
t293 = ct{1343};
t2931 = ct{1344};
t2932 = ct{1345};
t2938 = ct{1346};
t294 = ct{1347};
t2940 = ct{1348};
t2944 = ct{1349};
t2945 = ct{1350};
t2946 = ct{1351};
t2949 = ct{1352};
t2950 = ct{1353};
t2951 = ct{1354};
t2952 = ct{1355};
t2953 = ct{1356};
t2954 = ct{1357};
t2955 = ct{1358};
t2956 = ct{1359};
t2957 = ct{1360};
t2959 = ct{1361};
t2960 = ct{1362};
t2961 = ct{1363};
t2962 = ct{1364};
t2963 = ct{1365};
t2964 = ct{1366};
t2966 = ct{1367};
t2967 = ct{1368};
t2969 = ct{1369};
t2975 = ct{1370};
t2976 = ct{1371};
t2977 = ct{1372};
t2978 = ct{1373};
t2979 = ct{1374};
t2982 = ct{1375};
t2983 = ct{1376};
t2988 = ct{1377};
t2989 = ct{1378};
t2991 = ct{1379};
t2992 = ct{1380};
t2994 = ct{1381};
t2995 = ct{1382};
t3 = ct{1383};
t30 = ct{1384};
t3001 = ct{1385};
t3002 = ct{1386};
t3003 = ct{1387};
t3004 = ct{1388};
t3005 = ct{1389};
t3006 = ct{1390};
t3007 = ct{1391};
t3008 = ct{1392};
t3009 = ct{1393};
t3010 = ct{1394};
t3011 = ct{1395};
t3012 = ct{1396};
t3013 = ct{1397};
t3014 = ct{1398};
t3015 = ct{1399};
t3016 = ct{1400};
t3017 = ct{1401};
t3019 = ct{1402};
t3020 = ct{1403};
t3021 = ct{1404};
t3022 = ct{1405};
t3023 = ct{1406};
t3025 = ct{1407};
t3028 = ct{1408};
t3030 = ct{1409};
t3034 = ct{1410};
t3035 = ct{1411};
t3037 = ct{1412};
t3039 = ct{1413};
t304 = ct{1414};
t3047 = ct{1415};
t3048 = ct{1416};
t3051 = ct{1417};
t3053 = ct{1418};
t3054 = ct{1419};
t3059 = ct{1420};
t3060 = ct{1421};
t3061 = ct{1422};
t3062 = ct{1423};
t3063 = ct{1424};
t3065 = ct{1425};
t3069 = ct{1426};
t3070 = ct{1427};
t3074 = ct{1428};
t3075 = ct{1429};
t3077 = ct{1430};
t3078 = ct{1431};
t3081 = ct{1432};
t3083 = ct{1433};
t3084 = ct{1434};
t3085 = ct{1435};
t3089 = ct{1436};
t3090 = ct{1437};
t3091 = ct{1438};
t3092 = ct{1439};
t3094 = ct{1440};
t3098 = ct{1441};
t3100 = ct{1442};
t3102 = ct{1443};
t3105 = ct{1444};
t3106 = ct{1445};
t3107 = ct{1446};
t3108 = ct{1447};
t3109 = ct{1448};
t3112 = ct{1449};
t3115 = ct{1450};
t3117 = ct{1451};
t3118 = ct{1452};
t3124 = ct{1453};
t3125 = ct{1454};
t3127 = ct{1455};
t3129 = ct{1456};
t3130 = ct{1457};
t3132 = ct{1458};
t3133 = ct{1459};
t3134 = ct{1460};
t3135 = ct{1461};
t3136 = ct{1462};
t3138 = ct{1463};
t3141 = ct{1464};
t3146 = ct{1465};
t3148 = ct{1466};
t3149 = ct{1467};
t3151 = ct{1468};
t3153 = ct{1469};
t3157 = ct{1470};
t3159 = ct{1471};
t3160 = ct{1472};
t3165 = ct{1473};
t3170 = ct{1474};
t3171 = ct{1475};
t3172 = ct{1476};
t3173 = ct{1477};
t3174 = ct{1478};
t3175 = ct{1479};
t3177 = ct{1480};
t3180 = ct{1481};
t3181 = ct{1482};
t3184 = ct{1483};
t3186 = ct{1484};
t3187 = ct{1485};
t3189 = ct{1486};
t3199 = ct{1487};
t3200 = ct{1488};
t3203 = ct{1489};
t3204 = ct{1490};
t3210 = ct{1491};
t3212 = ct{1492};
t3218 = ct{1493};
t3220 = ct{1494};
t3222 = ct{1495};
t3224 = ct{1496};
t3226 = ct{1497};
t3228 = ct{1498};
t3233 = ct{1499};
t3235 = ct{1500};
t3237 = ct{1501};
t3238 = ct{1502};
t3241 = ct{1503};
t3242 = ct{1504};
t3243 = ct{1505};
t3246 = ct{1506};
t3247 = ct{1507};
t3248 = ct{1508};
t3249 = ct{1509};
t3256 = ct{1510};
t3260 = ct{1511};
t3263 = ct{1512};
t3265 = ct{1513};
t3266 = ct{1514};
t3272 = ct{1515};
t3274 = ct{1516};
t3277 = ct{1517};
t3284 = ct{1518};
t3285 = ct{1519};
t3286 = ct{1520};
t3290 = ct{1521};
t3291 = ct{1522};
t3294 = ct{1523};
t33 = ct{1524};
t3304 = ct{1525};
t3305 = ct{1526};
t3317 = ct{1527};
t3319 = ct{1528};
t3321 = ct{1529};
t3322 = ct{1530};
t3323 = ct{1531};
t3325 = ct{1532};
t3330 = ct{1533};
t3331 = ct{1534};
t3332 = ct{1535};
t3337 = ct{1536};
t3339 = ct{1537};
t3341 = ct{1538};
t3351 = ct{1539};
t3360 = ct{1540};
t3364 = ct{1541};
t3370 = ct{1542};
t3380 = ct{1543};
t3383 = ct{1544};
t34 = ct{1545};
t3403 = ct{1546};
t3415 = ct{1547};
t3416 = ct{1548};
t3417 = ct{1549};
t3419 = ct{1550};
t3420 = ct{1551};
t3426 = ct{1552};
t3434 = ct{1553};
t3438 = ct{1554};
t3441 = ct{1555};
t3449 = ct{1556};
t3453 = ct{1557};
t3457 = ct{1558};
t3459 = ct{1559};
t346 = ct{1560};
t3469 = ct{1561};
t347 = ct{1562};
t3471 = ct{1563};
t3474 = ct{1564};
t3478 = ct{1565};
t348 = ct{1566};
t3483 = ct{1567};
t3484 = ct{1568};
t3487 = ct{1569};
t3495 = ct{1570};
t3499 = ct{1571};
t35 = ct{1572};
t3503 = ct{1573};
t3504 = ct{1574};
t3505 = ct{1575};
t3520 = ct{1576};
t3521 = ct{1577};
t3522 = ct{1578};
t3523 = ct{1579};
t3524 = ct{1580};
t3527 = ct{1581};
t3531 = ct{1582};
t3539 = ct{1583};
t3547 = ct{1584};
t3548 = ct{1585};
t3551 = ct{1586};
t3559 = ct{1587};
t3562 = ct{1588};
t3565 = ct{1589};
t3569 = ct{1590};
t3577 = ct{1591};
t3580 = ct{1592};
t3581 = ct{1593};
t3583 = ct{1594};
t3595 = ct{1595};
t3609 = ct{1596};
t3611 = ct{1597};
t3617 = ct{1598};
t3619 = ct{1599};
t3635 = ct{1600};
t3639 = ct{1601};
t3643 = ct{1602};
t3644 = ct{1603};
t3657 = ct{1604};
t3666 = ct{1605};
t3671 = ct{1606};
t3672 = ct{1607};
t3677 = ct{1608};
t3678 = ct{1609};
t3680 = ct{1610};
t3683 = ct{1611};
t3684 = ct{1612};
t3699 = ct{1613};
t3701 = ct{1614};
t3702 = ct{1615};
t3704 = ct{1616};
t3706 = ct{1617};
t3708 = ct{1618};
t3709 = ct{1619};
t3713 = ct{1620};
t3717 = ct{1621};
t3721 = ct{1622};
t3730 = ct{1623};
t3739 = ct{1624};
t3743 = ct{1625};
t3749 = ct{1626};
t375 = ct{1627};
t3750 = ct{1628};
t3752 = ct{1629};
t376 = ct{1630};
t3761 = ct{1631};
t3768 = ct{1632};
t3769 = ct{1633};
t377 = ct{1634};
t3771 = ct{1635};
t3772 = ct{1636};
t3787 = ct{1637};
t3790 = ct{1638};
t3791 = ct{1639};
t3792 = ct{1640};
t38 = ct{1641};
t381 = ct{1642};
t3819 = ct{1643};
t382 = ct{1644};
t3823 = ct{1645};
t3828 = ct{1646};
t383 = ct{1647};
t3832 = ct{1648};
t3835 = ct{1649};
t3842 = ct{1650};
t3847 = ct{1651};
t3855 = ct{1652};
t3858 = ct{1653};
t3862 = ct{1654};
t3866 = ct{1655};
t3873 = ct{1656};
t3880 = ct{1657};
t3882 = ct{1658};
t3883 = ct{1659};
t390 = ct{1660};
t3900 = ct{1661};
t3902 = ct{1662};
t3906 = ct{1663};
t3907 = ct{1664};
t3908 = ct{1665};
t3909 = ct{1666};
t3910 = ct{1667};
t3913 = ct{1668};
t3915 = ct{1669};
t3916 = ct{1670};
t3926 = ct{1671};
t3928 = ct{1672};
t3929 = ct{1673};
t3930 = ct{1674};
t3931 = ct{1675};
t3932 = ct{1676};
t3933 = ct{1677};
t3936 = ct{1678};
t3937 = ct{1679};
t394 = ct{1680};
t3940 = ct{1681};
t3942 = ct{1682};
t3944 = ct{1683};
t3952 = ct{1684};
t3955 = ct{1685};
t3956 = ct{1686};
t3957 = ct{1687};
t3959 = ct{1688};
t3960 = ct{1689};
t3961 = ct{1690};
t3962 = ct{1691};
t3964 = ct{1692};
t3965 = ct{1693};
t3967 = ct{1694};
t3968 = ct{1695};
t3969 = ct{1696};
t3971 = ct{1697};
t3974 = ct{1698};
t3976 = ct{1699};
t3981 = ct{1700};
t3982 = ct{1701};
t3983 = ct{1702};
t399 = ct{1703};
t3993 = ct{1704};
t3994 = ct{1705};
t3995 = ct{1706};
t3996 = ct{1707};
t3998 = ct{1708};
t4 = ct{1709};
t400 = ct{1710};
t4003 = ct{1711};
t4004 = ct{1712};
t4008 = ct{1713};
t401 = ct{1714};
t4012 = ct{1715};
t4014 = ct{1716};
t4028 = ct{1717};
t4029 = ct{1718};
t4033 = ct{1719};
t4035 = ct{1720};
t4036 = ct{1721};
t4038 = ct{1722};
t4042 = ct{1723};
t4047 = ct{1724};
t4048 = ct{1725};
t4049 = ct{1726};
t4051 = ct{1727};
t4052 = ct{1728};
t4054 = ct{1729};
t4056 = ct{1730};
t4058 = ct{1731};
t4059 = ct{1732};
t4060 = ct{1733};
t4061 = ct{1734};
t4064 = ct{1735};
t4068 = ct{1736};
t4070 = ct{1737};
t4073 = ct{1738};
t4074 = ct{1739};
t4078 = ct{1740};
t4081 = ct{1741};
t4086 = ct{1742};
t4087 = ct{1743};
t4088 = ct{1744};
t4089 = ct{1745};
t4090 = ct{1746};
t4092 = ct{1747};
t4093 = ct{1748};
t4098 = ct{1749};
t41 = ct{1750};
t410 = ct{1751};
t411 = ct{1752};
t412 = ct{1753};
t4121 = ct{1754};
t413 = ct{1755};
t414 = ct{1756};
t4141 = ct{1757};
t4142 = ct{1758};
t4143 = ct{1759};
t415 = ct{1760};
t4153 = ct{1761};
t4161 = ct{1762};
t4172 = ct{1763};
t4181 = ct{1764};
t4182 = ct{1765};
t4189 = ct{1766};
t4190 = ct{1767};
t4197 = ct{1768};
t420 = ct{1769};
t421 = ct{1770};
t4210 = ct{1771};
t4218 = ct{1772};
t4234 = ct{1773};
t4235 = ct{1774};
t4236 = ct{1775};
t424 = ct{1776};
t425 = ct{1777};
t4256 = ct{1778};
t4269 = ct{1779};
t4294 = ct{1780};
t4295 = ct{1781};
t4297 = ct{1782};
t4298 = ct{1783};
t430 = ct{1784};
t431 = ct{1785};
t4323 = ct{1786};
t433 = ct{1787};
t434 = ct{1788};
t4349 = ct{1789};
t4355 = ct{1790};
t436 = ct{1791};
t4363 = ct{1792};
t44 = ct{1793};
t445 = ct{1794};
t4474 = ct{1795};
t4475 = ct{1796};
t448 = ct{1797};
t450 = ct{1798};
t4509 = ct{1799};
t451 = ct{1800};
t456 = ct{1801};
t459 = ct{1802};
t4597 = ct{1803};
t4598 = ct{1804};
t4599 = ct{1805};
t46 = ct{1806};
t4603 = ct{1807};
t463 = ct{1808};
t465 = ct{1809};
t466 = ct{1810};
t4752 = ct{1811};
t478 = ct{1812};
t48 = ct{1813};
t482 = ct{1814};
t483 = ct{1815};
t484 = ct{1816};
t485 = ct{1817};
t487 = ct{1818};
t488 = ct{1819};
t49 = ct{1820};
t491 = ct{1821};
t495 = ct{1822};
t496 = ct{1823};
t5 = ct{1824};
t50 = ct{1825};
t501 = ct{1826};
t502 = ct{1827};
t504 = ct{1828};
t505 = ct{1829};
t506 = ct{1830};
t51 = ct{1831};
t514 = ct{1832};
t519 = ct{1833};
t523 = ct{1834};
t524 = ct{1835};
t527 = ct{1836};
t530 = ct{1837};
t534 = ct{1838};
t537 = ct{1839};
t539 = ct{1840};
t54 = ct{1841};
t541 = ct{1842};
t542 = ct{1843};
t544 = ct{1844};
t546 = ct{1845};
t547 = ct{1846};
t55 = ct{1847};
t550 = ct{1848};
t553 = ct{1849};
t555 = ct{1850};
t557 = ct{1851};
t558 = ct{1852};
t559 = ct{1853};
t56 = ct{1854};
t560 = ct{1855};
t561 = ct{1856};
t57 = ct{1857};
t572 = ct{1858};
t573 = ct{1859};
t574 = ct{1860};
t575 = ct{1861};
t578 = ct{1862};
t581 = ct{1863};
t584 = ct{1864};
t587 = ct{1865};
t59 = ct{1866};
t595 = ct{1867};
t6 = ct{1868};
t603 = ct{1869};
t61 = ct{1870};
t614 = ct{1871};
t623 = ct{1872};
t624 = ct{1873};
t627 = ct{1874};
t628 = ct{1875};
t629 = ct{1876};
t631 = ct{1877};
t632 = ct{1878};
t634 = ct{1879};
t641 = ct{1880};
t643 = ct{1881};
t644 = ct{1882};
t648 = ct{1883};
t65 = ct{1884};
t650 = ct{1885};
t651 = ct{1886};
t652 = ct{1887};
t653 = ct{1888};
t654 = ct{1889};
t655 = ct{1890};
t657 = ct{1891};
t662 = ct{1892};
t663 = ct{1893};
t664 = ct{1894};
t665 = ct{1895};
t666 = ct{1896};
t667 = ct{1897};
t668 = ct{1898};
t669 = ct{1899};
t672 = ct{1900};
t674 = ct{1901};
t675 = ct{1902};
t676 = ct{1903};
t68 = ct{1904};
t69 = ct{1905};
t693 = ct{1906};
t699 = ct{1907};
t7 = ct{1908};
t701 = ct{1909};
t71 = ct{1910};
t720 = ct{1911};
t721 = ct{1912};
t722 = ct{1913};
t724 = ct{1914};
t73 = ct{1915};
t731 = ct{1916};
t732 = ct{1917};
t735 = ct{1918};
t736 = ct{1919};
t741 = ct{1920};
t744 = ct{1921};
t746 = ct{1922};
t749 = ct{1923};
t750 = ct{1924};
t751 = ct{1925};
t752 = ct{1926};
t753 = ct{1927};
t754 = ct{1928};
t755 = ct{1929};
t756 = ct{1930};
t757 = ct{1931};
t759 = ct{1932};
t760 = ct{1933};
t761 = ct{1934};
t762 = ct{1935};
t764 = ct{1936};
t765 = ct{1937};
t768 = ct{1938};
t769 = ct{1939};
t772 = ct{1940};
t774 = ct{1941};
t776 = ct{1942};
t778 = ct{1943};
t779 = ct{1944};
t792 = ct{1945};
t794 = ct{1946};
t795 = ct{1947};
t797 = ct{1948};
t799 = ct{1949};
t8 = ct{1950};
t801 = ct{1951};
t802 = ct{1952};
t803 = ct{1953};
t805 = ct{1954};
t806 = ct{1955};
t811 = ct{1956};
t817 = ct{1957};
t818 = ct{1958};
t819 = ct{1959};
t820 = ct{1960};
t821 = ct{1961};
t822 = ct{1962};
t823 = ct{1963};
t824 = ct{1964};
t826 = ct{1965};
t828 = ct{1966};
t830 = ct{1967};
t831 = ct{1968};
t834 = ct{1969};
t835 = ct{1970};
t836 = ct{1971};
t837 = ct{1972};
t838 = ct{1973};
t839 = ct{1974};
t841 = ct{1975};
t842 = ct{1976};
t843 = ct{1977};
t844 = ct{1978};
t845 = ct{1979};
t846 = ct{1980};
t847 = ct{1981};
t848 = ct{1982};
t850 = ct{1983};
t851 = ct{1984};
t852 = ct{1985};
t853 = ct{1986};
t854 = ct{1987};
t855 = ct{1988};
t858 = ct{1989};
t859 = ct{1990};
t862 = ct{1991};
t863 = ct{1992};
t864 = ct{1993};
t865 = ct{1994};
t867 = ct{1995};
t868 = ct{1996};
t869 = ct{1997};
t870 = ct{1998};
t871 = ct{1999};
t872 = ct{2000};
t873 = ct{2001};
t874 = ct{2002};
t875 = ct{2003};
t876 = ct{2004};
t877 = ct{2005};
t879 = ct{2006};
t881 = ct{2007};
t882 = ct{2008};
t884 = ct{2009};
t885 = ct{2010};
t886 = ct{2011};
t887 = ct{2012};
t888 = ct{2013};
t889 = ct{2014};
t890 = ct{2015};
t891 = ct{2016};
t892 = ct{2017};
t893 = ct{2018};
t894 = ct{2019};
t895 = ct{2020};
t896 = ct{2021};
t897 = ct{2022};
t898 = ct{2023};
t9 = ct{2024};
t900 = ct{2025};
t901 = ct{2026};
t902 = ct{2027};
t903 = ct{2028};
t904 = ct{2029};
t906 = ct{2030};
t907 = ct{2031};
t908 = ct{2032};
t909 = ct{2033};
t910 = ct{2034};
t912 = ct{2035};
t913 = ct{2036};
t914 = ct{2037};
t915 = ct{2038};
t916 = ct{2039};
t917 = ct{2040};
t918 = ct{2041};
t919 = ct{2042};
t923 = ct{2043};
t924 = ct{2044};
t925 = ct{2045};
t926 = ct{2046};
t927 = ct{2047};
t928 = ct{2048};
t933 = ct{2049};
t934 = ct{2050};
t941 = ct{2051};
t947 = ct{2052};
t948 = ct{2053};
t949 = ct{2054};
t950 = ct{2055};
t951 = ct{2056};
t952 = ct{2057};
t953 = ct{2058};
t954 = ct{2059};
t955 = ct{2060};
t957 = ct{2061};
t964 = ct{2062};
t965 = ct{2063};
t966 = ct{2064};
t968 = ct{2065};
t970 = ct{2066};
t972 = ct{2067};
t974 = ct{2068};
t976 = ct{2069};
t977 = ct{2070};
t979 = ct{2071};
t980 = ct{2072};
t983 = ct{2073};
t985 = ct{2074};
t986 = ct{2075};
t987 = ct{2076};
t990 = ct{2077};
t991 = ct{2078};
t992 = ct{2079};
t993 = ct{2080};
t994 = ct{2081};
t995 = ct{2082};
t996 = ct{2083};
t4094 = Mt.*t381.*t3940;
t4095 = Mt.*t382.*t3940;
t4099 = -t4090;
t4101 = Mt.*t381.*t3971;
t4103 = Mt.*t420.*t3937;
t4104 = Mt.*t421.*t3937;
t4106 = Mt.*t382.*t3969;
t4109 = Mt.*t420.*t3940;
t4110 = Mt.*t421.*t3940;
t4112 = t399+t530+t736+t836+t858+t1287;
t4113 = t663+t768+t968+t1097+t1150;
t4114 = t676+t910+t933+t1093+t1109;
t4118 = Mt.*t421.*t3971;
t4119 = B_cg_H.*Mb.*t1512.*t3138;
t4124 = Mt.*t420.*t3969;
t4136 = t722+t913+t941+t1105+t1148;
t4149 = Mt.*t2240.*(-t44+t390+t430-t524+t587);
t4155 = -t4141;
t4156 = -t4142;
t4159 = -t1512.*(t553-t741+dpsi1.*(t103-t544)+dth2.*(t105-t465));
t4164 = t1185+t1707+t1775;
t4169 = Mb.*t1660.*t3138;
t4171 = -t4153;
t4185 = dx.*t4172;
t4188 = dx.*t4161;
t4196 = t3862.*3.36554e-3;
t4207 = -t4189;
t4222 = -Mt.*t2730.*(t433-t828+T_cg_H.*(t197-t537));
t4224 = t3930.*3.36554e-3;
t4231 = t977.*(-t488+t603+dpsi1.*(t105-t465)+dth2.*(t103-t544)).*(-3.36554e-3);
t4232 = Mt.*t2730.*(t433-t828+T_cg_H.*(t197-t537));
t4253 = -t4235;
t4279 = t4070.*(-3.36554e-3);
t4282 = t4070.*3.36554e-3;
t4290 = -t4098.*(t105-t465);
t4301 = Mt.*t1381.*t3940;
t4304 = -t4294;
t4306 = -t4297;
t4316 = Mb.*t2563.*t3138;
t4330 = Mb.*t2638.*t3138;
t4332 = -t4323;
t4335 = Mt.*t2240.*t3531;
t4342 = t1512.*(t553-t741+dpsi1.*(t103-t544)+dth2.*(t105-t465)).*(-3.36554e-3);
t4354 = Mt.*t1734.*t3937;
t4356 = Mt.*t1727.*t3940;
t4358 = -t4349;
t4367 = dy.*t4363;
t4368 = dz.*t4363;
t4418 = t4098.*(t105-t465).*(-3.36554e-3);
t4420 = -Mt.*t3937.*(t451-t831+T_cg_H.*(t214-t541));
t4421 = -Mt.*t3940.*(t433-t828+T_cg_H.*(t197-t537));
t4432 = -Mt.*t3969.*(t433-t828+T_cg_H.*(t197-t537));
t4454 = t822+t1377+t1432+t1454+t1514;
t4457 = Mt.*t2763.*t3940;
t4458 = Mt.*t2730.*t3937;
t4479 = Mt.*t3940.*(-t120+t425+t519-t651+t765);
t4481 = Mt.*t3937.*(-t130+t436+t523-t657+t769);
t4492 = -t4474;
t4512 = dphi1.*t4509;
t4581 = t986+t1062+t1372+t1424+t1507+t1524;
t4714 = t346+t347+t348+t578+t581+t584+t652+t653+t654+t4081;
t4716 = -dphi1.*(t4078-t4081);
t4796 = t28+t57+t160+t1600+t2306+t2477+t3580;
t4995 = t4181+t4599;
t1099 = -t1024;
t1107 = -t1030;
t1220 = -t1167;
t1271 = -t1202;
t1276 = B_cg_H.*t1240;
t1278 = -t1207;
t1286 = T_cg_H.*t1240;
t1288 = -t1218;
t1291 = dphi1.*t1238;
t1293 = dphi1.*t1240;
t1295 = dphi2.*t1240;
t1297 = dpsi1.*t1240;
t1299 = -t1230;
t1423 = -t1363;
t1473 = -t1400;
t1480 = -t1406;
t1510 = t213+t1238;
t1519 = -t1447;
t1544 = t1435./2.0;
t1546 = -t1468;
t1551 = -t1471;
t1558 = B_cg_H.*t1505;
t1564 = T_cg_H.*t1505;
t1570 = dphi2.*t1505;
t1571 = dpsi1.*t1505;
t1578 = t2.*t1508;
t1579 = -t1501;
t1583 = -t1534;
t1584 = -t1535;
t1586 = t7.*t1508;
t1590 = -t1508;
t1604 = t1505.^2;
t1607 = t1501./2.0;
t1612 = B_cg_H.*t1580;
t1625 = -t1572;
t1626 = t1527./2.0;
t1633 = -t1585;
t1638 = -t1595;
t1643 = Mb.*t5.*t9.*t1487;
t1666 = Mt.*t5.*t9.*t1528;
t1720 = -t1655;
t1722 = -t1656;
t1739 = -t1680;
t1740 = -t1681;
t1754 = t496.*t1240;
t1755 = -t1698;
t1771 = t11.*t420.*t1240;
t1778 = -t1719;
t1779 = -t1721;
t1787 = t1698./2.0;
t1792 = t1705./2.0;
t1800 = -t1736;
t1809 = -t1746;
t1833 = -t1789;
t1834 = -t1790;
t1835 = -t1793;
t1843 = -t1783;
t1847 = t1753./2.0;
t1858 = t1774./2.0;
t1878 = -t1842;
t1880 = t1811./2.0;
t1885 = t1816./2.0;
t1902 = Mb.*t382.*t1487;
t1904 = -t1882;
t1920 = Mt.*t382.*t1528;
t1923 = t817.*t1240;
t1933 = t11.*t381.*t1505;
t1945 = -t1901;
t1949 = Mb.*t420.*t1487;
t1959 = t1883./2.0;
t1967 = t1891./2.0;
t1978 = -t1917;
t1984 = Mt.*t420.*t1528;
t1987 = t11.*t463.*t1505;
t1988 = -t1240.*(t105-t465);
t1992 = -t1927;
t1993 = -t1929;
t1996 = t11.*t420.*t1505;
t2006 = -t1938;
t2009 = -t1944;
t2014 = t487.*t1505;
t2018 = -t1952;
t2022 = t8.*t1927;
t2027 = t903.*t1240;
t2030 = t496.*t1505;
t2036 = t1927./2.0;
t2041 = t1935./2.0;
t2048 = t1937./2.0;
t2049 = t1938./2.0;
t2065 = -t1977;
t2070 = t1953./2.0;
t2074 = t1955./2.0;
t2076 = t1957./2.0;
t2077 = t9.*t871.*t1240;
t2082 = t8.*t873.*t1240;
t2088 = -t2000;
t2092 = -t2005;
t2105 = t4.*t495.*t1505;
t2109 = -t2016;
t2110 = t8.*t506.*t1505;
t2113 = -t2020;
t2114 = -t2021;
t2117 = -t2024;
t2124 = -t2029;
t2126 = t1240.*(t105-t465).*(-1.0./2.0);
t2129 = t1994./2.0;
t2132 = t1995./2.0;
t2137 = t2000./2.0;
t2143 = t2005./2.0;
t2153 = -t2061;
t2163 = t2021./2.0;
t2168 = t2029./2.0;
t2184 = t4.*t555.*t1505;
t2192 = -t2106;
t2199 = -t2123;
t2212 = t2083./2.0;
t2213 = t2084./2.0;
t2217 = -t2140;
t2219 = -t2142;
t2230 = -t2149;
t2232 = t2099./2.0;
t2235 = t2103./2.0;
t2248 = t2123./2.0;
t2265 = t794.*t1505;
t2268 = Mb.*t15.*t2099;
t2269 = Mb.*t15.*t2100;
t2272 = -t2185;
t2276 = -t2189;
t2277 = -t2191;
t2289 = -t2206;
t2292 = -t2216;
t2301 = t2185./2.0;
t2304 = t2187./2.0;
t2308 = t817.*t1505;
t2319 = t424+t881+t1021;
t2325 = t434+t884+t1025;
t2330 = -t2297;
t2338 = -t2275;
t2344 = t2239./2.0;
t2352 = -t2293;
t2361 = t2274./2.0;
t2364 = t903.*t1505;
t2365 = t4.*t819.*t1505;
t2367 = -t1505.*(t105-t465);
t2373 = -t2310;
t2377 = -t2315;
t2381 = -t2317;
t2396 = Mt.*t5.*t9.*t2174;
t2406 = -t2334;
t2414 = t2309./2.0;
t2415 = t2310./2.0;
t2418 = t2315./2.0;
t2419 = t2317./2.0;
t2434 = t1178.*t1240;
t2437 = -t2402;
t2439 = t4.*t868.*t1505;
t2440 = t4.*t871.*t1505;
t2441 = t3.*t872.*t1505;
t2442 = t8.*t869.*t1505;
t2443 = -t1505.*(t103-t544);
t2445 = -t2366;
t2446 = t8.*t872.*t1505;
t2449 = t1505.*(t105-t465);
t2453 = -t2372;
t2486 = t1435.*3.36554e-3;
t2499 = t2366./2.0;
t2506 = t2371./2.0;
t2507 = t2372./2.0;
t2509 = t2375./2.0;
t2511 = t2378./2.0;
t2521 = -t2424;
t2522 = -t2473;
t2523 = -t2426;
t2524 = t964.*t1505;
t2526 = -t2428;
t2541 = -t1505.*(t214-t541);
t2542 = -t2436;
t2561 = -t2456;
t2569 = -t2465;
t2571 = t1501.*3.36554e-3;
t2580 = t2540.*2.0;
t2582 = t2436./2.0;
t2596 = t1505.*(t103-t544).*(-1.0./2.0);
t2618 = t2456./2.0;
t2623 = t2460./2.0;
t2629 = t1527.*3.36554e-3;
t2631 = t1031.*t1505;
t2636 = Mb.*t15.*t2432;
t2641 = t1047.*t1505;
t2643 = -t2540;
t2650 = -t2592;
t2666 = t1435.*3.367829185e-3;
t2667 = -t2567;
t2678 = t2529./2.0;
t2684 = t2536./2.0;
t2691 = t1505.*(t214-t541).*(-1.0./2.0);
t2727 = -t2628;
t2729 = -Mt.*t4.*t5.*(t431+t909+T_cg_H.*(t195-t634));
t2733 = Mb.*t15.*t2536;
t2736 = -t2680;
t2738 = -t2687;
t2739 = -t2688;
t2772 = t2635./2.0;
t2775 = t1435.*8.56645e-6;
t2785 = t1501.*3.367829185e-3;
t2791 = Mt.*t382.*t2174;
t2793 = t1527.*9.52624335e-4;
t2795 = Mt.*t4.*t5.*(t431+t909+T_cg_H.*(t195-t634));
t2800 = t1527.*3.372816795e-3;
t2818 = -t2757;
t2822 = t1501.*8.56645e-6;
t2826 = t1178.*t1505;
t2827 = t1179.*t1505;
t2831 = t1240.*t1430;
t2834 = -t2778;
t2850 = t1698.*3.36554e-3;
t2851 = Mt.*t420.*t2174;
t2853 = -t2792;
t2860 = t1705.*3.36554e-3;
t2862 = -t2799;
t2866 = t2770./2.0;
t2867 = t2771./2.0;
t2881 = -t2816;
t2882 = -t2817;
t2897 = -t2855;
t2898 = -t2856;
t2899 = t1238.*t1505;
t2900 = -t1505.*(t534-t546);
t2903 = -t2863;
t2914 = t750+t882+t1216;
t2923 = -t2847;
t2924 = t1753.*3.36554e-3;
t2935 = t1505.*(t534-t546).*-2.0;
t2942 = t1774.*3.36554e-3;
t2943 = t2833./2.0;
t2947 = -t2876;
t2972 = Mb.*t15.*t2833;
t2981 = t1811.*3.36554e-3;
t2985 = t1816.*3.36554e-3;
t2996 = -t2931;
t2998 = t1505.*(t534-t546).*(-1.0./2.0);
t3026 = t1698.*3.367829185e-3;
t3027 = -t2953;
t3031 = t1705.*3.367829185e-3;
t3033 = -t2983;
t3036 = -Mt.*t381.*(t431+t909+T_cg_H.*(t195-t634));
t3038 = -t2991;
t3041 = -t3001;
t3042 = -t3002;
t3043 = -t3005;
t3044 = -t3008;
t3045 = -t3009;
t3046 = -t3013;
t3050 = -t2978;
t3057 = t1698.*8.56645e-6;
t3064 = t1705.*8.56645e-6;
t3066 = t1753.*3.372786875e-3;
t3072 = t1753.*9.53094055e-4;
t3082 = t400+t1170+t1279;
t3087 = t1774.*3.367829185e-3;
t3093 = t1883.*3.36554e-3;
t3095 = -Mt.*t421.*(t431+t909+T_cg_H.*(t195-t634));
t3097 = t1891.*3.36554e-3;
t3099 = Mt.*t4.*t5.*t2915;
t3110 = -t3053;
t3113 = t561+t631+t895+t974;
t3114 = t1811.*9.52624335e-4;
t3119 = t1816.*9.52624335e-4;
t3122 = t1811.*3.372816795e-3;
t3128 = t1816.*3.372816795e-3;
t3131 = t1774.*8.56645e-6;
t3142 = t1917.*3.36554e-3;
t3143 = t478+t701+t894+t976;
t3145 = t1955.*3.36554e-3;
t3147 = t1957.*3.36554e-3;
t3154 = t1927.*3.36554e-3;
t3158 = -t3118;
t3162 = t1935.*3.36554e-3;
t3164 = -t3125;
t3166 = t1937.*3.36554e-3;
t3167 = t1938.*3.36554e-3;
t3169 = t3129.*2.0;
t3176 = -t3141;
t3179 = t1953.*3.36554e-3;
t3195 = t1505.*t1512;
t3197 = -t3129;
t3207 = t1976.*3.36554e-3;
t3213 = t2029.*3.36554e-3;
t3216 = -t3148;
t3217 = t1240.*(t105-t465).*(-3.36554e-3);
t3221 = t1994.*3.36554e-3;
t3223 = t1995.*3.36554e-3;
t3229 = -t3159;
t3230 = t2000.*3.36554e-3;
t3236 = t2005.*3.36554e-3;
t3239 = t1891.*3.372786875e-3;
t3240 = t1891.*9.53094055e-4;
t3244 = t1883.*3.367829185e-3;
t3245 = -t3172;
t3252 = t2021.*3.36554e-3;
t3270 = t2123.*3.36554e-3;
t3273 = t1953.*3.372786875e-3;
t3275 = -t3222;
t3278 = t1957.*3.372786875e-3;
t3279 = t2083.*3.36554e-3;
t3280 = t2084.*3.36554e-3;
t3281 = t1953.*9.53094055e-4;
t3282 = -t3228;
t3287 = t1957.*9.53094055e-4;
t3295 = -t3242;
t3296 = t1955.*3.367829185e-3;
t3298 = t1927.*3.367829185e-3;
t3301 = t2099.*3.36554e-3;
t3303 = t1935.*3.367829185e-3;
t3306 = t1937.*3.367829185e-3;
t3307 = t1938.*3.367829185e-3;
t3309 = t2103.*3.36554e-3;
t3315 = t1883.*8.56645e-6;
t3333 = -t3263;
t3345 = t2021.*9.52624335e-4;
t3353 = t1935.*8.56645e-6;
t3357 = t2021.*3.372816795e-3;
t3359 = t1240.*(t105-t465).*(-3.372786875e-3);
t3361 = t1937.*8.56645e-6;
t3362 = t1938.*8.56645e-6;
t3366 = t1994.*9.52624335e-4;
t3368 = t1995.*3.372786875e-3;
t3369 = t1240.*(t105-t465).*(-9.53094055e-4);
t3372 = t1994.*3.372816795e-3;
t3373 = t1995.*9.53094055e-4;
t3376 = t2005.*3.372786875e-3;
t3378 = t2005.*9.53094055e-4;
t3379 = -t3294;
t3381 = t2029.*3.367829185e-3;
t3384 = t1995.*3.367829185e-3;
t3385 = t2000.*3.367829185e-3;
t3389 = t2185.*3.36554e-3;
t3390 = t2005.*3.367829185e-3;
t3391 = t2187.*3.36554e-3;
t3392 = t2191.*3.36554e-3;
t3393 = t1955.*8.56645e-6;
t3395 = t1927.*8.56645e-6;
t3397 = Mt.*t381.*t2915;
t3399 = -t3322;
t3412 = -t3383;
t3418 = t2239.*3.36554e-3;
t3422 = t2103.*3.372816795e-3;
t3425 = t1995.*8.56645e-6;
t3427 = t2123.*9.52624335e-4;
t3429 = t2000.*8.56645e-6;
t3436 = t2005.*8.56645e-6;
t3437 = t2123.*3.372816795e-3;
t3446 = t2083.*3.367829185e-3;
t3447 = t2084.*3.367829185e-3;
t3448 = t2271.*3.36554e-3;
t3450 = t2099.*9.52624335e-4;
t3451 = t2274.*3.36554e-3;
t3454 = t2099.*3.372816795e-3;
t3460 = t2103.*9.52624335e-4;
t3461 = t2029.*8.56645e-6;
t3468 = Mt.*t421.*t2915;
t3488 = -t3416;
t3490 = t2309.*3.36554e-3;
t3492 = -t3417;
t3493 = t2310.*3.36554e-3;
t3498 = t2315.*3.36554e-3;
t3500 = t2317.*3.36554e-3;
t3501 = t2083.*8.56645e-6;
t3502 = t2084.*8.56645e-6;
t3507 = t2185.*9.52624335e-4;
t3512 = t2187.*9.52624335e-4;
t3514 = t2185.*3.372816795e-3;
t3516 = t2187.*3.372816795e-3;
t3525 = t2239.*3.367829185e-3;
t3528 = -t3503;
t3529 = -t3505;
t3530 = -t3487;
t3536 = t2366.*3.36554e-3;
t3542 = t2371.*3.36554e-3;
t3543 = t2372.*3.36554e-3;
t3545 = t2375.*3.36554e-3;
t3546 = t2378.*3.36554e-3;
t3549 = t2274.*3.367829185e-3;
t3560 = t2310.*9.52624335e-4;
t3561 = t2460.*3.36554e-3;
t3564 = t2309.*9.53094055e-4;
t3566 = t2315.*9.52624335e-4;
t3567 = t2310.*3.372816795e-3;
t3568 = t2317.*3.372786875e-3;
t3570 = -t3523;
t3571 = -t3524;
t3572 = t2315.*3.372816795e-3;
t3573 = t2317.*9.53094055e-4;
t3574 = Mt.*t10.*t3483;
t3576 = t2309.*3.367829185e-3;
t3579 = t2317.*3.367829185e-3;
t3584 = t2436.*3.36554e-3;
t3589 = t1505.*(t103-t544).*(-3.36554e-3);
t3590 = t2239.*8.56645e-6;
t3596 = t2456.*3.36554e-3;
t3598 = t2309.*3.372786875e-3;
t3612 = t2540.*6.73108e-3;
t3614 = t2274.*8.56645e-6;
t3621 = t1505.*(t103-t544).*3.36554e-3;
t3626 = t2371.*9.52624335e-4;
t3627 = t2372.*9.52624335e-4;
t3628 = Mt.*t5.*t7.*t3483;
t3630 = t2366.*3.372816795e-3;
t3632 = t2375.*3.372786875e-3;
t3636 = t2378.*9.52624335e-4;
t3637 = t2371.*3.372816795e-3;
t3638 = t2372.*3.372816795e-3;
t3641 = t2375.*9.53094055e-4;
t3642 = t2378.*3.372816795e-3;
t3647 = -t3577;
t3649 = t2375.*3.367829185e-3;
t3651 = t2529.*3.36554e-3;
t3652 = t2536.*3.36554e-3;
t3655 = t1505.*(t214-t541).*(-3.36554e-3);
t3656 = t2309.*8.56645e-6;
t3659 = t2317.*8.56645e-6;
t3662 = t2366.*9.52624335e-4;
t3663 = Mt.*t2.*t5.*t3483;
t3679 = t448+t826+t835+t1494;
t3686 = -t3617;
t3687 = -t3619;
t3696 = t2456.*9.52624335e-4;
t3698 = t2460.*9.52624335e-4;
t3700 = t2456.*3.372816795e-3;
t3703 = t2460.*3.372816795e-3;
t3705 = t1505.*(t103-t544).*(-3.367829185e-3);
t3710 = t2635.*3.36554e-3;
t3716 = t2436.*9.52624335e-4;
t3722 = t2436.*3.372816795e-3;
t3724 = -t3657;
t3726 = t2375.*8.56645e-6;
C = ft_7({B_cg_H,ITail,Mb,Mm,Mt,T_cg_H,dphi1,dphi2,dpsi1,dth1,dth2,dx,dy,dz,t10,t1003,t1004,t1005,t1006,t1007,t1008,t1009,t1010,t1011,t1012,t1013,t1014,t1015,t1016,t1017,t1018,t1019,t1020,t1023,t1026,t1029,t103,t1031,t1036,t1037,t1041,t1042,t1043,t1044,t1045,t1046,t1047,t1049,t105,t1050,t1051,t1052,t1053,t1054,t1055,t1056,t1057,t1058,t1059,t1060,t1061,t1063,t1064,t1065,t1067,t1068,t1071,t1072,t1073,t1074,t1075,t1076,t1077,t1078,t1079,t1080,t1081,t1082,t1084,t1085,t1086,t1088,t1097,t1099,t11,t1102,t1107,t1108,t1113,t1114,t1115,t1116,t1117,t1118,t1119,t1120,t1121,t1122,t1123,t1124,t1125,t1126,t1127,t1128,t1129,t1130,t1131,t1132,t1133,t1134,t1135,t1136,t1137,t1138,t1139,t1140,t1141,t1142,t1143,t1144,t1145,t1146,t1147,t1149,t1152,t1153,t1154,t1155,t1156,t1157,t1158,t1159,t1160,t1161,t1162,t1163,t1164,t1165,t1166,t1167,t1168,t1169,t1170,t1171,t1172,t1173,t1174,t1176,t1177,t1178,t1179,t1181,t1182,t1183,t1184,t1185,t1186,t1187,t1188,t1189,t1190,t1191,t1192,t1193,t1194,t1195,t1196,t1197,t1199,t120,t1200,t1201,t1202,t1203,t1205,t1206,t1209,t1211,t1212,t1213,t1214,t1215,t1220,t1221,t1223,t1224,t1225,t1226,t1227,t1228,t1229,t123,t1230,t1231,t1232,t1234,t1235,t1236,t1237,t1240,t1242,t1243,t1244,t1245,t1246,t1247,t1248,t1250,t1251,t1252,t1253,t1255,t1256,t1257,t1260,t1261,t1262,t1263,t1264,t1265,t1266,t1268,t1270,t1271,t1272,t1275,t1276,t1278,t1280,t1282,t1283,t1284,t1285,t1286,t1288,t1289,t1291,t1293,t1295,t1296,t1297,t1299,t130,t1301,t1302,t1303,t1304,t1305,t1306,t1307,t1308,t1309,t1311,t1312,t1313,t1319,t1320,t1322,t1323,t1324,t1325,t1328,t1329,t1331,t1332,t1334,t1335,t1337,t1338,t134,t1340,t1341,t1342,t1343,t1344,t1345,t1348,t1349,t1352,t1354,t1355,t1356,t1357,t1358,t1360,t1361,t1362,t1365,t1366,t1367,t1368,t1370,t1371,t1373,t1374,t1378,t1379,t1380,t1381,t1382,t1383,t1384,t1385,t1386,t1388,t1389,t1391,t1393,t1394,t1395,t1396,t1397,t1399,t1402,t1403,t1405,t1406,t1407,t1408,t1409,t1410,t1412,t1413,t1414,t1415,t1416,t1418,t1419,t1421,t1422,t1423,t1426,t1427,t1429,t1430,t1431,t1433,t1434,t1435,t1437,t1438,t1439,t144,t1440,t1441,t1442,t1443,t1444,t1445,t1446,t1448,t1450,t1451,t1453,t1455,t1456,t1457,t1458,t1459,t1460,t1461,t1462,t1463,t1465,t1466,t1467,t1468,t1469,t1470,t1472,t1473,t1475,t1476,t1477,t1478,t1479,t1480,t1481,t1482,t1483,t1484,t1486,t1487,t1488,t1489,t1491,t1492,t1493,t1495,t1496,t1497,t1498,t15,t1500,t1503,t1504,t1505,t1506,t1508,t1509,t1510,t1511,t1512,t1513,t1515,t1516,t1517,t1518,t1519,t1520,t1521,t1522,t1523,t1525,t1526,t1527,t1528,t1529,t1531,t1532,t1533,t1535,t1536,t1537,t1539,t1540,t1541,t1542,t1543,t1544,t1546,t1547,t1548,t1549,t1550,t1551,t1552,t1553,t1555,t1557,t1558,t1559,t1560,t1561,t1562,t1563,t1564,t1565,t1566,t1567,t1568,t1570,t1571,t1573,t1576,t1577,t1578,t1579,t1580,t1581,t1582,t1583,t1584,t1585,t1586,t1587,t1588,t1589,t1590,t1591,t1592,t1593,t1594,t1595,t1596,t1597,t1598,t1599,t160,t1601,t1602,t1603,t1604,t1605,t1606,t1607,t1609,t161,t1610,t1612,t1613,t1614,t1615,t1616,t1617,t1618,t1619,t162,t1620,t1621,t1624,t1625,t1626,t1627,t1628,t1632,t1633,t1635,t1636,t1637,t1638,t1639,t1640,t1641,t1642,t1643,t1644,t1645,t1646,t1647,t1648,t1649,t1651,t1652,t1653,t1654,t1655,t1656,t1657,t1658,t1659,t1660,t1661,t1663,t1664,t1665,t1666,t1667,t1668,t1669,t1670,t1671,t1672,t1673,t1674,t1675,t1676,t1677,t1678,t1679,t1680,t1681,t1682,t1683,t1684,t1685,t1686,t1687,t1688,t1689,t1690,t1691,t1692,t1693,t1694,t1695,t1698,t1699,t1700,t1701,t1702,t1703,t1704,t1705,t1706,t1709,t1711,t1712,t1715,t1716,t1718,t1719,t1720,t1721,t1722,t1723,t1725,t1726,t1727,t1729,t1730,t1731,t1732,t1733,t1734,t1735,t1736,t1737,t1739,t1740,t1741,t1742,t1743,t1744,t1745,t1746,t1747,t1748,t1749,t1750,t1751,t1753,t1754,t1755,t1756,t1758,t1759,t1760,t1761,t1762,t1764,t1765,t1767,t1768,t1769,t1770,t1771,t1772,t1773,t1774,t1776,t1777,t1778,t1779,t1783,t1784,t1785,t1786,t1787,t1788,t1789,t1790,t1791,t1792,t1794,t1795,t1796,t1797,t1798,t1799,t1800,t1801,t1802,t1803,t1805,t1806,t1808,t1809,t1810,t1811,t1812,t1813,t1814,t1815,t1816,t1817,t1819,t1820,t1821,t1824,t1825,t1826,t1827,t1828,t1829,t1830,t1831,t1832,t1833,t1834,t1835,t1836,t1837,t1838,t1839,t1841,t1842,t1843,t1844,t1845,t1846,t1847,t1849,t1851,t1852,t1856,t1857,t1858,t1859,t1860,t1862,t1863,t1864,t1865,t1866,t1867,t1870,t1871,t1872,t1873,t1874,t1875,t1877,t1878,t1880,t1881,t1882,t1883,t1884,t1885,t1887,t1888,t1890,t1891,t1893,t1894,t1895,t1896,t1897,t1898,t1899,t1900,t1902,t1903,t1904,t1905,t1906,t1907,t1908,t1909,t1910,t1911,t1912,t1913,t1914,t1915,t1916,t1917,t1918,t1919,t1920,t1921,t1922,t1923,t1924,t1926,t1928,t1929,t1930,t1931,t1933,t1935,t1937,t1938,t1939,t1940,t1941,t1942,t1943,t1945,t1949,t195,t1950,t1951,t1952,t1953,t1955,t1956,t1957,t1959,t1960,t1961,t1962,t1963,t1964,t1965,t1966,t1967,t1968,t1969,t197,t1970,t1971,t1973,t1974,t1975,t1976,t1977,t1978,t1979,t1980,t1981,t1982,t1983,t1984,t1985,t1986,t1987,t1988,t1989,t1990,t1992,t1993,t1994,t1995,t1996,t1998,t1999,t2,t2000,t2004,t2005,t2006,t2007,t2008,t2009,t2014,t2015,t2016,t2017,t2018,t2020,t2022,t2023,t2024,t2025,t2026,t2027,t2028,t2030,t2033,t2035,t2036,t2037,t2041,t2042,t2043,t2045,t2046,t2047,t2048,t2049,t2050,t2052,t2053,t2056,t2057,t2058,t2059,t2060,t2061,t2062,t2063,t2064,t2065,t2066,t2067,t2068,t2069,t2070,t2072,t2074,t2075,t2076,t2077,t2078,t2079,t2081,t2082,t2083,t2084,t2087,t2088,t2090,t2091,t2092,t2094,t2095,t2096,t2097,t2098,t2099,t2100,t2102,t2103,t2104,t2105,t2106,t2108,t2109,t2110,t2113,t2114,t2116,t2117,t2118,t2119,t2120,t2121,t2123,t2124,t2126,t2127,t2129,t2130,t2131,t2132,t2134,t2135,t2136,t2137,t214,t2141,t2142,t2143,t2144,t2146,t2147,t2148,t2149,t2150,t2151,t2152,t2153,t2154,t2155,t2156,t2157,t2158,t2161,t2163,t2165,t2167,t2168,t2171,t2172,t2174,t2176,t2178,t2179,t2181,t2182,t2183,t2184,t2186,t2187,t2188,t2189,t2190,t2191,t2192,t2196,t2199,t2201,t2202,t2203,t2205,t2206,t2208,t2209,t2211,t2212,t2213,t2214,t2215,t2216,t2217,t2218,t2219,t2220,t2221,t2222,t2223,t2224,t2225,t2227,t2228,t2229,t2230,t2231,t2232,t2233,t2235,t2237,t2238,t2239,t2240,t2242,t2245,t2246,t2247,t2248,t2249,t2251,t2252,t2253,t2254,t2255,t2257,t2258,t2259,t2260,t2262,t2263,t2265,t2267,t2268,t2269,t2271,t2272,t2273,t2274,t2276,t2277,t2281,t2285,t2286,t2287,t2288,t2289,t2290,t2292,t2293,t2294,t2296,t2298,t2299,t2301,t2303,t2304,t2305,t2307,t2308,t2309,t2312,t2314,t2316,t2317,t2318,t2319,t2320,t2321,t2322,t2323,t2324,t2325,t2326,t2327,t2328,t2330,t2331,t2334,t2335,t2336,t2338,t2339,t2340,t2341,t2342,t2343,t2344,t2345,t2346,t2347,t2348,t2349,t2350,t2351,t2352,t2353,t2354,t2356,t2357,t2358,t2360,t2361,t2362,t2363,t2364,t2365,t2369,t2371,t2373,t2375,t2376,t2377,t2378,t2380,t2381,t2382,t2385,t2386,t2387,t2388,t2389,t2390,t2392,t2396,t2397,t2399,t24,t2400,t2401,t2403,t2404,t2406,t2407,t2408,t2409,t2411,t2412,t2414,t2415,t2417,t2418,t2419,t2420,t2422,t2423,t2425,t2426,t2427,t2428,t2429,t2430,t2431,t2432,t2433,t2434,t2435,t2436,t2437,t2438,t2439,t2440,t2441,t2442,t2443,t2445,t2446,t2447,t2449,t2453,t2455,t2458,t2460,t2461,t2462,t2463,t2464,t2465,t2466,t2467,t2468,t2469,t2470,t2471,t2472,t2474,t2476,t2479,t2480,t2483,t2484,t2485,t2486,t2487,t2488,t2489,t2492,t2495,t2499,t25,t2502,t2503,t2504,t2505,t2506,t2507,t2509,t2511,t2512,t2513,t2514,t2515,t2516,t2518,t2519,t2520,t2521,t2522,t2523,t2524,t2525,t2526,t2527,t2528,t2529,t2530,t2531,t2532,t2533,t2534,t2535,t2536,t2539,t2540,t2541,t2542,t2543,t2544,t2545,t2546,t2547,t2550,t2551,t2552,t2560,t2561,t2562,t2563,t2564,t2565,t2566,t2567,t2568,t2569,t2570,t2571,t2576,t2577,t2579,t2580,t2581,t2582,t2584,t2587,t2588,t2589,t259,t2590,t2591,t2596,t2597,t2598,t2599,t26,t260,t2600,t2605,t2607,t2610,t2611,t2612,t2613,t2614,t2615,t2616,t2617,t2618,t2619,t2620,t2621,t2622,t2623,t2624,t2627,t2629,t2631,t2632,t2634,t2635,t2636,t2637,t2638,t2640,t2641,t2643,t2646,t2647,t2648,t2649,t2650,t2654,t2656,t2657,t2658,t2660,t2662,t2663,t2664,t2665,t2666,t2667,t2668,t2669,t2671,t2673,t2677,t2678,t2679,t2681,t2682,t2683,t2684,t2688,t2689,t2691,t2692,t2695,t2696,t2698,t2699,t27,t2700,t2702,t2703,t2704,t2705,t2706,t2707,t2708,t2710,t2711,t2712,t2714,t2715,t2717,t2718,t2722,t2723,t2725,t2727,t2730,t2731,t2732,t2733,t2735,t2736,t2738,t2739,t2740,t2742,t2743,t2744,t2745,t2746,t2747,t2748,t2749,t2750,t2751,t2752,t2754,t2755,t2756,t2758,t2759,t276,t2760,t2761,t2762,t2763,t2764,t2765,t2766,t2768,t2769,t277,t2770,t2771,t2772,t2774,t2775,t2776,t2778,t2781,t2782,t2783,t2784,t2785,t2786,t2787,t2788,t2790,t2791,t2792,t2793,t2795,t2797,t2799,t28,t2800,t2802,t2803,t2804,t2806,t2807,t2811,t2813,t2816,t2817,t2818,t2819,t2821,t2822,t2823,t2824,t2825,t2826,t2827,t2828,t283,t2830,t2831,t2832,t2833,t2834,t2835,t2836,t2837,t2838,t2839,t284,t2841,t2842,t2843,t2844,t2845,t2846,t2847,t2849,t285,t2850,t2851,t2853,t2857,t2859,t286,t2860,t2862,t2864,t2865,t2866,t2867,t2869,t287,t2870,t2871,t2872,t2874,t2875,t2876,t2877,t2878,t2879,t288,t2880,t2881,t2882,t2883,t2884,t2885,t2886,t2887,t2889,t289,t2890,t2892,t2895,t2896,t2897,t2898,t2899,t290,t2900,t2902,t2903,t2906,t2907,t2909,t291,t2912,t2913,t2914,t2915,t2916,t2917,t2918,t2919,t292,t2920,t2923,t2924,t2926,t2927,t2928,t2929,t293,t2931,t2932,t2935,t2938,t294,t2940,t2942,t2943,t2944,t2945,t2946,t2947,t2949,t2950,t2951,t2952,t2953,t2954,t2955,t2956,t2957,t2959,t2960,t2961,t2962,t2963,t2964,t2966,t2967,t2969,t2972,t2975,t2976,t2977,t2978,t2979,t2981,t2982,t2985,t2988,t2989,t2992,t2994,t2995,t2996,t2998,t3,t30,t3003,t3004,t3006,t3007,t3008,t3009,t3010,t3011,t3012,t3014,t3015,t3016,t3017,t3019,t3020,t3021,t3022,t3023,t3025,t3026,t3027,t3028,t3030,t3031,t3033,t3034,t3035,t3036,t3037,t3038,t3039,t304,t3041,t3042,t3043,t3044,t3045,t3046,t3047,t3048,t3050,t3051,t3054,t3057,t3059,t3060,t3061,t3062,t3063,t3064,t3065,t3066,t3069,t3070,t3072,t3074,t3075,t3077,t3078,t3081,t3082,t3083,t3084,t3085,t3087,t3089,t3090,t3091,t3092,t3093,t3094,t3095,t3097,t3098,t3099,t3100,t3102,t3105,t3106,t3107,t3108,t3109,t3110,t3112,t3113,t3114,t3115,t3117,t3119,t3122,t3124,t3127,t3128,t3129,t3130,t3131,t3132,t3133,t3134,t3135,t3136,t3138,t3142,t3143,t3145,t3146,t3147,t3149,t3151,t3153,t3154,t3157,t3158,t3160,t3162,t3164,t3165,t3166,t3167,t3169,t3170,t3171,t3173,t3174,t3175,t3176,t3177,t3179,t3180,t3181,t3184,t3186,t3187,t3189,t3195,t3197,t3199,t3200,t3203,t3204,t3207,t3210,t3212,t3213,t3216,t3217,t3218,t3220,t3221,t3222,t3223,t3224,t3226,t3228,t3229,t3230,t3233,t3235,t3236,t3237,t3238,t3239,t3240,t3241,t3243,t3244,t3245,t3246,t3247,t3248,t3249,t3252,t3256,t3260,t3263,t3265,t3266,t3270,t3272,t3273,t3274,t3275,t3277,t3278,t3279,t3280,t3281,t3282,t3284,t3285,t3286,t3287,t3290,t3291,t3294,t3295,t3296,t3298,t33,t3301,t3303,t3304,t3305,t3306,t3307,t3309,t3315,t3317,t3319,t3321,t3322,t3323,t3325,t3330,t3331,t3332,t3333,t3337,t3339,t3341,t3345,t3351,t3353,t3357,t3359,t3360,t3361,t3362,t3364,t3366,t3368,t3369,t3370,t3372,t3373,t3376,t3378,t3379,t3380,t3381,t3384,t3385,t3389,t3390,t3391,t3392,t3393,t3395,t3397,t3399,t34,t3403,t3412,t3415,t3416,t3418,t3419,t3420,t3422,t3425,t3426,t3427,t3429,t3434,t3436,t3437,t3438,t3441,t3446,t3447,t3448,t3449,t3450,t3451,t3453,t3454,t3457,t3459,t3460,t3461,t3468,t3469,t3471,t3474,t3478,t3483,t3484,t3487,t3488,t3490,t3492,t3493,t3495,t3498,t3499,t35,t3500,t3501,t3502,t3504,t3507,t3512,t3514,t3516,t3520,t3521,t3522,t3523,t3524,t3525,t3527,t3528,t3529,t3530,t3531,t3536,t3539,t3542,t3543,t3545,t3546,t3547,t3548,t3549,t3551,t3559,t3560,t3561,t3562,t3564,t3565,t3566,t3567,t3568,t3569,t3570,t3571,t3572,t3573,t3574,t3576,t3579,t3581,t3583,t3584,t3590,t3595,t3596,t3598,t3609,t3611,t3612,t3614,t3617,t3619,t3621,t3626,t3627,t3628,t3630,t3632,t3635,t3636,t3637,t3638,t3639,t3641,t3642,t3643,t3644,t3647,t3649,t3651,t3652,t3655,t3656,t3657,t3659,t3662,t3663,t3666,t3671,t3672,t3677,t3678,t3679,t3680,t3683,t3684,t3686,t3687,t3696,t3698,t3699,t3700,t3701,t3702,t3703,t3704,t3706,t3708,t3709,t3710,t3713,t3716,t3717,t3721,t3722,t3724,t3726,t3730,t3739,t3743,t3749,t375,t3750,t3752,t376,t3761,t3768,t3769,t377,t3771,t3772,t3787,t3790,t3791,t3792,t38,t381,t3819,t382,t3823,t3828,t383,t3832,t3835,t3842,t3847,t3855,t3858,t3862,t3866,t3873,t3880,t3882,t3883,t390,t3900,t3902,t3906,t3907,t3908,t3909,t3910,t3913,t3915,t3916,t3926,t3928,t3929,t3930,t3931,t3932,t3933,t3936,t3937,t394,t3940,t3942,t3944,t3952,t3955,t3956,t3957,t3959,t3960,t3961,t3962,t3964,t3965,t3967,t3968,t3969,t3971,t3974,t3976,t3981,t3982,t3983,t3993,t3994,t3995,t3996,t3998,t4,t400,t4003,t4004,t4008,t401,t4012,t4014,t4028,t4029,t4033,t4035,t4036,t4038,t4042,t4047,t4048,t4049,t4051,t4052,t4054,t4056,t4058,t4059,t4060,t4061,t4064,t4068,t4070,t4073,t4074,t4078,t4081,t4086,t4087,t4088,t4089,t4090,t4092,t4093,t4094,t4095,t4098,t4099,t41,t410,t4101,t4103,t4104,t4106,t4109,t411,t4110,t4112,t4113,t4114,t4118,t4119,t412,t4121,t4124,t413,t4136,t414,t4141,t4143,t4149,t415,t4153,t4155,t4156,t4159,t4164,t4169,t4171,t4182,t4185,t4188,t4189,t4190,t4196,t4197,t420,t4207,t421,t4210,t4218,t4222,t4224,t4231,t4232,t4234,t4236,t425,t4253,t4256,t4269,t4282,t4290,t4295,t4298,t430,t4301,t4304,t4306,t431,t4316,t4323,t433,t4330,t4332,t4335,t4342,t4349,t4354,t4355,t4356,t4358,t436,t4367,t4368,t44,t4418,t4420,t4421,t4432,t445,t4454,t4457,t4458,t4475,t4479,t4481,t4492,t450,t451,t4512,t456,t4581,t459,t4597,t4598,t46,t4603,t465,t466,t4716,t4752,t4796,t48,t482,t483,t484,t485,t487,t488,t49,t491,t496,t4995,t5,t50,t501,t502,t504,t505,t51,t514,t519,t523,t524,t527,t530,t534,t537,t539,t54,t541,t542,t544,t546,t547,t55,t550,t553,t557,t558,t559,t56,t560,t57,t572,t573,t574,t575,t587,t59,t595,t6,t603,t61,t614,t623,t624,t627,t628,t629,t632,t634,t641,t643,t644,t648,t65,t650,t651,t655,t657,t662,t664,t665,t666,t667,t668,t669,t672,t674,t675,t68,t69,t693,t699,t7,t71,t720,t721,t724,t73,t731,t732,t735,t736,t741,t744,t746,t749,t751,t752,t753,t754,t755,t756,t757,t759,t760,t761,t762,t764,t765,t769,t772,t774,t776,t778,t779,t792,t795,t797,t799,t8,t801,t802,t803,t805,t806,t811,t817,t818,t820,t821,t823,t824,t828,t830,t831,t834,t837,t838,t839,t841,t842,t843,t844,t845,t846,t847,t848,t850,t851,t852,t853,t854,t855,t859,t862,t863,t864,t865,t867,t868,t870,t871,t872,t874,t875,t876,t877,t879,t885,t886,t887,t888,t889,t890,t891,t892,t893,t896,t897,t898,t9,t900,t901,t902,t903,t904,t906,t907,t908,t909,t912,t914,t915,t916,t917,t918,t919,t923,t924,t925,t926,t927,t928,t934,t947,t948,t949,t950,t951,t952,t953,t954,t955,t957,t964,t965,t966,t970,t972,t977,t979,t980,t983,t985,t987,t990,t991,t992,t993,t994,t995,t996});
end
function C = ft_7(ct)
B_cg_H = ct{1};
ITail = ct{2};
Mb = ct{3};
Mm = ct{4};
Mt = ct{5};
T_cg_H = ct{6};
dphi1 = ct{7};
dphi2 = ct{8};
dpsi1 = ct{9};
dth1 = ct{10};
dth2 = ct{11};
dx = ct{12};
dy = ct{13};
dz = ct{14};
t10 = ct{15};
t1003 = ct{16};
t1004 = ct{17};
t1005 = ct{18};
t1006 = ct{19};
t1007 = ct{20};
t1008 = ct{21};
t1009 = ct{22};
t1010 = ct{23};
t1011 = ct{24};
t1012 = ct{25};
t1013 = ct{26};
t1014 = ct{27};
t1015 = ct{28};
t1016 = ct{29};
t1017 = ct{30};
t1018 = ct{31};
t1019 = ct{32};
t1020 = ct{33};
t1023 = ct{34};
t1026 = ct{35};
t1029 = ct{36};
t103 = ct{37};
t1031 = ct{38};
t1036 = ct{39};
t1037 = ct{40};
t1041 = ct{41};
t1042 = ct{42};
t1043 = ct{43};
t1044 = ct{44};
t1045 = ct{45};
t1046 = ct{46};
t1047 = ct{47};
t1049 = ct{48};
t105 = ct{49};
t1050 = ct{50};
t1051 = ct{51};
t1052 = ct{52};
t1053 = ct{53};
t1054 = ct{54};
t1055 = ct{55};
t1056 = ct{56};
t1057 = ct{57};
t1058 = ct{58};
t1059 = ct{59};
t1060 = ct{60};
t1061 = ct{61};
t1063 = ct{62};
t1064 = ct{63};
t1065 = ct{64};
t1067 = ct{65};
t1068 = ct{66};
t1071 = ct{67};
t1072 = ct{68};
t1073 = ct{69};
t1074 = ct{70};
t1075 = ct{71};
t1076 = ct{72};
t1077 = ct{73};
t1078 = ct{74};
t1079 = ct{75};
t1080 = ct{76};
t1081 = ct{77};
t1082 = ct{78};
t1084 = ct{79};
t1085 = ct{80};
t1086 = ct{81};
t1088 = ct{82};
t1097 = ct{83};
t1099 = ct{84};
t11 = ct{85};
t1102 = ct{86};
t1107 = ct{87};
t1108 = ct{88};
t1113 = ct{89};
t1114 = ct{90};
t1115 = ct{91};
t1116 = ct{92};
t1117 = ct{93};
t1118 = ct{94};
t1119 = ct{95};
t1120 = ct{96};
t1121 = ct{97};
t1122 = ct{98};
t1123 = ct{99};
t1124 = ct{100};
t1125 = ct{101};
t1126 = ct{102};
t1127 = ct{103};
t1128 = ct{104};
t1129 = ct{105};
t1130 = ct{106};
t1131 = ct{107};
t1132 = ct{108};
t1133 = ct{109};
t1134 = ct{110};
t1135 = ct{111};
t1136 = ct{112};
t1137 = ct{113};
t1138 = ct{114};
t1139 = ct{115};
t1140 = ct{116};
t1141 = ct{117};
t1142 = ct{118};
t1143 = ct{119};
t1144 = ct{120};
t1145 = ct{121};
t1146 = ct{122};
t1147 = ct{123};
t1149 = ct{124};
t1152 = ct{125};
t1153 = ct{126};
t1154 = ct{127};
t1155 = ct{128};
t1156 = ct{129};
t1157 = ct{130};
t1158 = ct{131};
t1159 = ct{132};
t1160 = ct{133};
t1161 = ct{134};
t1162 = ct{135};
t1163 = ct{136};
t1164 = ct{137};
t1165 = ct{138};
t1166 = ct{139};
t1167 = ct{140};
t1168 = ct{141};
t1169 = ct{142};
t1170 = ct{143};
t1171 = ct{144};
t1172 = ct{145};
t1173 = ct{146};
t1174 = ct{147};
t1176 = ct{148};
t1177 = ct{149};
t1178 = ct{150};
t1179 = ct{151};
t1181 = ct{152};
t1182 = ct{153};
t1183 = ct{154};
t1184 = ct{155};
t1185 = ct{156};
t1186 = ct{157};
t1187 = ct{158};
t1188 = ct{159};
t1189 = ct{160};
t1190 = ct{161};
t1191 = ct{162};
t1192 = ct{163};
t1193 = ct{164};
t1194 = ct{165};
t1195 = ct{166};
t1196 = ct{167};
t1197 = ct{168};
t1199 = ct{169};
t120 = ct{170};
t1200 = ct{171};
t1201 = ct{172};
t1202 = ct{173};
t1203 = ct{174};
t1205 = ct{175};
t1206 = ct{176};
t1209 = ct{177};
t1211 = ct{178};
t1212 = ct{179};
t1213 = ct{180};
t1214 = ct{181};
t1215 = ct{182};
t1220 = ct{183};
t1221 = ct{184};
t1223 = ct{185};
t1224 = ct{186};
t1225 = ct{187};
t1226 = ct{188};
t1227 = ct{189};
t1228 = ct{190};
t1229 = ct{191};
t123 = ct{192};
t1230 = ct{193};
t1231 = ct{194};
t1232 = ct{195};
t1234 = ct{196};
t1235 = ct{197};
t1236 = ct{198};
t1237 = ct{199};
t1240 = ct{200};
t1242 = ct{201};
t1243 = ct{202};
t1244 = ct{203};
t1245 = ct{204};
t1246 = ct{205};
t1247 = ct{206};
t1248 = ct{207};
t1250 = ct{208};
t1251 = ct{209};
t1252 = ct{210};
t1253 = ct{211};
t1255 = ct{212};
t1256 = ct{213};
t1257 = ct{214};
t1260 = ct{215};
t1261 = ct{216};
t1262 = ct{217};
t1263 = ct{218};
t1264 = ct{219};
t1265 = ct{220};
t1266 = ct{221};
t1268 = ct{222};
t1270 = ct{223};
t1271 = ct{224};
t1272 = ct{225};
t1275 = ct{226};
t1276 = ct{227};
t1278 = ct{228};
t1280 = ct{229};
t1282 = ct{230};
t1283 = ct{231};
t1284 = ct{232};
t1285 = ct{233};
t1286 = ct{234};
t1288 = ct{235};
t1289 = ct{236};
t1291 = ct{237};
t1293 = ct{238};
t1295 = ct{239};
t1296 = ct{240};
t1297 = ct{241};
t1299 = ct{242};
t130 = ct{243};
t1301 = ct{244};
t1302 = ct{245};
t1303 = ct{246};
t1304 = ct{247};
t1305 = ct{248};
t1306 = ct{249};
t1307 = ct{250};
t1308 = ct{251};
t1309 = ct{252};
t1311 = ct{253};
t1312 = ct{254};
t1313 = ct{255};
t1319 = ct{256};
t1320 = ct{257};
t1322 = ct{258};
t1323 = ct{259};
t1324 = ct{260};
t1325 = ct{261};
t1328 = ct{262};
t1329 = ct{263};
t1331 = ct{264};
t1332 = ct{265};
t1334 = ct{266};
t1335 = ct{267};
t1337 = ct{268};
t1338 = ct{269};
t134 = ct{270};
t1340 = ct{271};
t1341 = ct{272};
t1342 = ct{273};
t1343 = ct{274};
t1344 = ct{275};
t1345 = ct{276};
t1348 = ct{277};
t1349 = ct{278};
t1352 = ct{279};
t1354 = ct{280};
t1355 = ct{281};
t1356 = ct{282};
t1357 = ct{283};
t1358 = ct{284};
t1360 = ct{285};
t1361 = ct{286};
t1362 = ct{287};
t1365 = ct{288};
t1366 = ct{289};
t1367 = ct{290};
t1368 = ct{291};
t1370 = ct{292};
t1371 = ct{293};
t1373 = ct{294};
t1374 = ct{295};
t1378 = ct{296};
t1379 = ct{297};
t1380 = ct{298};
t1381 = ct{299};
t1382 = ct{300};
t1383 = ct{301};
t1384 = ct{302};
t1385 = ct{303};
t1386 = ct{304};
t1388 = ct{305};
t1389 = ct{306};
t1391 = ct{307};
t1393 = ct{308};
t1394 = ct{309};
t1395 = ct{310};
t1396 = ct{311};
t1397 = ct{312};
t1399 = ct{313};
t1402 = ct{314};
t1403 = ct{315};
t1405 = ct{316};
t1406 = ct{317};
t1407 = ct{318};
t1408 = ct{319};
t1409 = ct{320};
t1410 = ct{321};
t1412 = ct{322};
t1413 = ct{323};
t1414 = ct{324};
t1415 = ct{325};
t1416 = ct{326};
t1418 = ct{327};
t1419 = ct{328};
t1421 = ct{329};
t1422 = ct{330};
t1423 = ct{331};
t1426 = ct{332};
t1427 = ct{333};
t1429 = ct{334};
t1430 = ct{335};
t1431 = ct{336};
t1433 = ct{337};
t1434 = ct{338};
t1435 = ct{339};
t1437 = ct{340};
t1438 = ct{341};
t1439 = ct{342};
t144 = ct{343};
t1440 = ct{344};
t1441 = ct{345};
t1442 = ct{346};
t1443 = ct{347};
t1444 = ct{348};
t1445 = ct{349};
t1446 = ct{350};
t1448 = ct{351};
t1450 = ct{352};
t1451 = ct{353};
t1453 = ct{354};
t1455 = ct{355};
t1456 = ct{356};
t1457 = ct{357};
t1458 = ct{358};
t1459 = ct{359};
t1460 = ct{360};
t1461 = ct{361};
t1462 = ct{362};
t1463 = ct{363};
t1465 = ct{364};
t1466 = ct{365};
t1467 = ct{366};
t1468 = ct{367};
t1469 = ct{368};
t1470 = ct{369};
t1472 = ct{370};
t1473 = ct{371};
t1475 = ct{372};
t1476 = ct{373};
t1477 = ct{374};
t1478 = ct{375};
t1479 = ct{376};
t1480 = ct{377};
t1481 = ct{378};
t1482 = ct{379};
t1483 = ct{380};
t1484 = ct{381};
t1486 = ct{382};
t1487 = ct{383};
t1488 = ct{384};
t1489 = ct{385};
t1491 = ct{386};
t1492 = ct{387};
t1493 = ct{388};
t1495 = ct{389};
t1496 = ct{390};
t1497 = ct{391};
t1498 = ct{392};
t15 = ct{393};
t1500 = ct{394};
t1503 = ct{395};
t1504 = ct{396};
t1505 = ct{397};
t1506 = ct{398};
t1508 = ct{399};
t1509 = ct{400};
t1510 = ct{401};
t1511 = ct{402};
t1512 = ct{403};
t1513 = ct{404};
t1515 = ct{405};
t1516 = ct{406};
t1517 = ct{407};
t1518 = ct{408};
t1519 = ct{409};
t1520 = ct{410};
t1521 = ct{411};
t1522 = ct{412};
t1523 = ct{413};
t1525 = ct{414};
t1526 = ct{415};
t1527 = ct{416};
t1528 = ct{417};
t1529 = ct{418};
t1531 = ct{419};
t1532 = ct{420};
t1533 = ct{421};
t1535 = ct{422};
t1536 = ct{423};
t1537 = ct{424};
t1539 = ct{425};
t1540 = ct{426};
t1541 = ct{427};
t1542 = ct{428};
t1543 = ct{429};
t1544 = ct{430};
t1546 = ct{431};
t1547 = ct{432};
t1548 = ct{433};
t1549 = ct{434};
t1550 = ct{435};
t1551 = ct{436};
t1552 = ct{437};
t1553 = ct{438};
t1555 = ct{439};
t1557 = ct{440};
t1558 = ct{441};
t1559 = ct{442};
t1560 = ct{443};
t1561 = ct{444};
t1562 = ct{445};
t1563 = ct{446};
t1564 = ct{447};
t1565 = ct{448};
t1566 = ct{449};
t1567 = ct{450};
t1568 = ct{451};
t1570 = ct{452};
t1571 = ct{453};
t1573 = ct{454};
t1576 = ct{455};
t1577 = ct{456};
t1578 = ct{457};
t1579 = ct{458};
t1580 = ct{459};
t1581 = ct{460};
t1582 = ct{461};
t1583 = ct{462};
t1584 = ct{463};
t1585 = ct{464};
t1586 = ct{465};
t1587 = ct{466};
t1588 = ct{467};
t1589 = ct{468};
t1590 = ct{469};
t1591 = ct{470};
t1592 = ct{471};
t1593 = ct{472};
t1594 = ct{473};
t1595 = ct{474};
t1596 = ct{475};
t1597 = ct{476};
t1598 = ct{477};
t1599 = ct{478};
t160 = ct{479};
t1601 = ct{480};
t1602 = ct{481};
t1603 = ct{482};
t1604 = ct{483};
t1605 = ct{484};
t1606 = ct{485};
t1607 = ct{486};
t1609 = ct{487};
t161 = ct{488};
t1610 = ct{489};
t1612 = ct{490};
t1613 = ct{491};
t1614 = ct{492};
t1615 = ct{493};
t1616 = ct{494};
t1617 = ct{495};
t1618 = ct{496};
t1619 = ct{497};
t162 = ct{498};
t1620 = ct{499};
t1621 = ct{500};
t1624 = ct{501};
t1625 = ct{502};
t1626 = ct{503};
t1627 = ct{504};
t1628 = ct{505};
t1632 = ct{506};
t1633 = ct{507};
t1635 = ct{508};
t1636 = ct{509};
t1637 = ct{510};
t1638 = ct{511};
t1639 = ct{512};
t1640 = ct{513};
t1641 = ct{514};
t1642 = ct{515};
t1643 = ct{516};
t1644 = ct{517};
t1645 = ct{518};
t1646 = ct{519};
t1647 = ct{520};
t1648 = ct{521};
t1649 = ct{522};
t1651 = ct{523};
t1652 = ct{524};
t1653 = ct{525};
t1654 = ct{526};
t1655 = ct{527};
t1656 = ct{528};
t1657 = ct{529};
t1658 = ct{530};
t1659 = ct{531};
t1660 = ct{532};
t1661 = ct{533};
t1663 = ct{534};
t1664 = ct{535};
t1665 = ct{536};
t1666 = ct{537};
t1667 = ct{538};
t1668 = ct{539};
t1669 = ct{540};
t1670 = ct{541};
t1671 = ct{542};
t1672 = ct{543};
t1673 = ct{544};
t1674 = ct{545};
t1675 = ct{546};
t1676 = ct{547};
t1677 = ct{548};
t1678 = ct{549};
t1679 = ct{550};
t1680 = ct{551};
t1681 = ct{552};
t1682 = ct{553};
t1683 = ct{554};
t1684 = ct{555};
t1685 = ct{556};
t1686 = ct{557};
t1687 = ct{558};
t1688 = ct{559};
t1689 = ct{560};
t1690 = ct{561};
t1691 = ct{562};
t1692 = ct{563};
t1693 = ct{564};
t1694 = ct{565};
t1695 = ct{566};
t1698 = ct{567};
t1699 = ct{568};
t1700 = ct{569};
t1701 = ct{570};
t1702 = ct{571};
t1703 = ct{572};
t1704 = ct{573};
t1705 = ct{574};
t1706 = ct{575};
t1709 = ct{576};
t1711 = ct{577};
t1712 = ct{578};
t1715 = ct{579};
t1716 = ct{580};
t1718 = ct{581};
t1719 = ct{582};
t1720 = ct{583};
t1721 = ct{584};
t1722 = ct{585};
t1723 = ct{586};
t1725 = ct{587};
t1726 = ct{588};
t1727 = ct{589};
t1729 = ct{590};
t1730 = ct{591};
t1731 = ct{592};
t1732 = ct{593};
t1733 = ct{594};
t1734 = ct{595};
t1735 = ct{596};
t1736 = ct{597};
t1737 = ct{598};
t1739 = ct{599};
t1740 = ct{600};
t1741 = ct{601};
t1742 = ct{602};
t1743 = ct{603};
t1744 = ct{604};
t1745 = ct{605};
t1746 = ct{606};
t1747 = ct{607};
t1748 = ct{608};
t1749 = ct{609};
t1750 = ct{610};
t1751 = ct{611};
t1753 = ct{612};
t1754 = ct{613};
t1755 = ct{614};
t1756 = ct{615};
t1758 = ct{616};
t1759 = ct{617};
t1760 = ct{618};
t1761 = ct{619};
t1762 = ct{620};
t1764 = ct{621};
t1765 = ct{622};
t1767 = ct{623};
t1768 = ct{624};
t1769 = ct{625};
t1770 = ct{626};
t1771 = ct{627};
t1772 = ct{628};
t1773 = ct{629};
t1774 = ct{630};
t1776 = ct{631};
t1777 = ct{632};
t1778 = ct{633};
t1779 = ct{634};
t1783 = ct{635};
t1784 = ct{636};
t1785 = ct{637};
t1786 = ct{638};
t1787 = ct{639};
t1788 = ct{640};
t1789 = ct{641};
t1790 = ct{642};
t1791 = ct{643};
t1792 = ct{644};
t1794 = ct{645};
t1795 = ct{646};
t1796 = ct{647};
t1797 = ct{648};
t1798 = ct{649};
t1799 = ct{650};
t1800 = ct{651};
t1801 = ct{652};
t1802 = ct{653};
t1803 = ct{654};
t1805 = ct{655};
t1806 = ct{656};
t1808 = ct{657};
t1809 = ct{658};
t1810 = ct{659};
t1811 = ct{660};
t1812 = ct{661};
t1813 = ct{662};
t1814 = ct{663};
t1815 = ct{664};
t1816 = ct{665};
t1817 = ct{666};
t1819 = ct{667};
t1820 = ct{668};
t1821 = ct{669};
t1824 = ct{670};
t1825 = ct{671};
t1826 = ct{672};
t1827 = ct{673};
t1828 = ct{674};
t1829 = ct{675};
t1830 = ct{676};
t1831 = ct{677};
t1832 = ct{678};
t1833 = ct{679};
t1834 = ct{680};
t1835 = ct{681};
t1836 = ct{682};
t1837 = ct{683};
t1838 = ct{684};
t1839 = ct{685};
t1841 = ct{686};
t1842 = ct{687};
t1843 = ct{688};
t1844 = ct{689};
t1845 = ct{690};
t1846 = ct{691};
t1847 = ct{692};
t1849 = ct{693};
t1851 = ct{694};
t1852 = ct{695};
t1856 = ct{696};
t1857 = ct{697};
t1858 = ct{698};
t1859 = ct{699};
t1860 = ct{700};
t1862 = ct{701};
t1863 = ct{702};
t1864 = ct{703};
t1865 = ct{704};
t1866 = ct{705};
t1867 = ct{706};
t1870 = ct{707};
t1871 = ct{708};
t1872 = ct{709};
t1873 = ct{710};
t1874 = ct{711};
t1875 = ct{712};
t1877 = ct{713};
t1878 = ct{714};
t1880 = ct{715};
t1881 = ct{716};
t1882 = ct{717};
t1883 = ct{718};
t1884 = ct{719};
t1885 = ct{720};
t1887 = ct{721};
t1888 = ct{722};
t1890 = ct{723};
t1891 = ct{724};
t1893 = ct{725};
t1894 = ct{726};
t1895 = ct{727};
t1896 = ct{728};
t1897 = ct{729};
t1898 = ct{730};
t1899 = ct{731};
t1900 = ct{732};
t1902 = ct{733};
t1903 = ct{734};
t1904 = ct{735};
t1905 = ct{736};
t1906 = ct{737};
t1907 = ct{738};
t1908 = ct{739};
t1909 = ct{740};
t1910 = ct{741};
t1911 = ct{742};
t1912 = ct{743};
t1913 = ct{744};
t1914 = ct{745};
t1915 = ct{746};
t1916 = ct{747};
t1917 = ct{748};
t1918 = ct{749};
t1919 = ct{750};
t1920 = ct{751};
t1921 = ct{752};
